simulink model "deltino"  (R2021b)
settings: Solver=VariableStepAuto  StartTime=0.0  StopTime=inf  FixedStep=0.0001  RelTol=1e-3
values from neighbouring files (symbols this model uses):
  alpha1 = 0    [compute_deltino_dyn_parallel.m]
  alpha2 = 2/3*pi    (= 2.09439510239)    [compute_deltino_dyn_parallel.m]
  alpha3 = 4/3*pi    (= 4.18879020479)    [compute_deltino_dyn_parallel.m]
  H = 0.05    [main.m]
  J_T = [J_1', J_2', J_3', J_4']    [main.m]
  K_d = 10    [main.m]
  K_el = 10000    [main.m]
  K_i = 1    [main.m]
  K_p = 200    [main.m]
  K_v = 10    [main.m]
  mu = 0.8    [main.m]
  ni_0 = zeros(18,1)    [main.m]
  offset1 = [l1/2; l2/2; -h/2]    [compute_deltino_dyn_parallel.m]    (also in main.m = [+l1/2; +l2/2; -h/2])
  offset2 = [l1/2; -l2/2; -h/2]    [compute_deltino_dyn_parallel.m]    (also in main.m = [+l1/2; -l2/2; -h/2])
  offset3 = [-l1/2; -l2/2; -h/2]    [compute_deltino_dyn_parallel.m]    (also in main.m)
  offset4 = [-l1/2; l2/2; -h/2]    [compute_deltino_dyn_parallel.m]    (also in main.m = [-l1/2; +l2/2; -h/2])
  p_leg1_0 = forward_kin(theta_leg1_0)    [main.m]
  p_leg2_0 = forward_kin(theta_leg2_0)    [main.m]
  p_leg3_0 = forward_kin(theta_leg3_0)    [main.m]
  p_leg4_0 = forward_kin(theta_leg4_0)    [main.m]
  points_ccw = [+0.1,  0.00 ... (first row only)    [main.m]
  points_cw = [-0.1,  0.00 ... (first row only)    [main.m]
  q_0 = [base_0; ypr_0; theta_leg1_0; ee_leg1_0; theta_leg2_0; ee_leg2_0;        theta_leg3_0; ee_leg3_0; theta_leg4_0; ee_leg4_0;]    [main.m]
  ratio = 2    [main.m]
  steps = 4+2*ratio    (= 8)    [main.m]
  theta_leg1_0 = [pi/6; pi/6; pi/6]    [main.m]
  theta_leg2_0 = [pi/6; pi/6; pi/6]    [main.m]
  theta_leg3_0 = [pi/6; pi/6; pi/6]    [main.m]
  theta_leg4_0 = [pi/6; pi/6; pi/6]    [main.m]
  ts = T/steps    (= 0.1875)    [main.m]
  ts2 = 3*ts    (= 0.5625)    [main.m]
  vel = 0.2    [main.m]
undefined symbols (not defined in the file or in its folder): l1, l_A, l_B, R, radius0, radius1, radius2, theta, WPs
libraries: simulink x14, dspsigops x12
(part 7 of 10)

== matlab function deltino/DELTINO DYNAMICS /compute_C ==
  data: q input; C output; q_dot input
function C = C(q, q_dot)
%#codegen

%    This function was generated by the Symbolic Math Toolbox version 9.0.
%    03-May-2022 19:50:17
phi = q(4); zeta = q(5); psi = q(6);
th11 = q(7); th12 = q(8); th13 = q(9);
th21 = q(13); th22 = q(14); th23 = q(15);
th31 = q(19); th32 = q(20); th33 = q(21);
th41 = q(25); th42 = q(26); th43 = q(27);

bx_dot = q_dot(1); by_dot = q_dot(2); bz_dot = q_dot(3);
phi_dot = q_dot(4); zeta_dot = q_dot(5); psi_dot = q(6);
th11_dot = q_dot(7); th12_dot = q_dot(8); th13_dot = q_dot(9);
th21_dot = q_dot(13); th22_dot = q_dot(14); th23_dot = q_dot(15);
th31_dot = q_dot(19); th32_dot = q_dot(20); th33_dot = q_dot(21);
th41_dot = q_dot(25); th42_dot = q_dot(26); th43_dot = q_dot(27);

t2 = cos(phi);
t3 = cos(psi);
t4 = cos(th11);
t5 = cos(th12);
t6 = cos(th13);
t7 = cos(th21);
t8 = cos(th22);
t9 = cos(th23);
t10 = cos(th31);
t11 = cos(th32);
t12 = cos(th33);
t13 = cos(th41);
t14 = cos(th42);
t15 = cos(th43);
t16 = cos(zeta);
t17 = sin(phi);
t18 = sin(psi);
t19 = sin(th11);
t20 = sin(th12);
t21 = sin(th13);
t22 = sin(th21);
t23 = sin(th22);
t24 = sin(th23);
t25 = sin(th31);
t26 = sin(th32);
t27 = sin(th33);
t28 = sin(th41);
t29 = sin(th42);
t30 = sin(th43);
t31 = sin(zeta);
t32 = psi.*2.0;
t33 = th11.*2.0;
t34 = th12.*2.0;
t35 = th13.*2.0;
t36 = th21.*2.0;
t37 = th22.*2.0;
t38 = th23.*2.0;
t39 = th31.*2.0;
t40 = th32.*2.0;
t41 = th33.*2.0;
t42 = th41.*2.0;
t43 = th42.*2.0;
t44 = th43.*2.0;
t45 = zeta.*2.0;
t92 = sqrt(3.0);
t46 = cos(t32);
t47 = t3.^2;
t48 = cos(t33);
t49 = cos(t34);
t50 = cos(t35);
t51 = cos(t36);
t52 = cos(t37);
t53 = cos(t38);
t54 = cos(t39);
t55 = cos(t40);
t56 = cos(t41);
t57 = cos(t42);
t58 = cos(t43);
t59 = cos(t44);
t60 = t4.^2;
t61 = t5.^2;
t62 = t6.^2;
t63 = t7.^2;
t64 = t8.^2;
t65 = t9.^2;
t66 = t10.^2;
t67 = t11.^2;
t68 = t12.^2;
t69 = t13.^2;
t70 = t14.^2;
t71 = t15.^2;
t72 = cos(t45);
t73 = t16.^2;
t74 = sin(t32);
t75 = sin(t33);
t76 = sin(t34);
t77 = sin(t35);
t78 = sin(t36);
t79 = sin(t37);
t80 = sin(t38);
t81 = sin(t39);
t82 = sin(t40);
t83 = sin(t41);
t84 = sin(t42);
t85 = sin(t43);
t86 = sin(t44);
t87 = sin(t45);
t88 = t2.*t3;
t89 = t2.*t18;
t90 = t3.*t17;
t91 = t17.*t18;
t93 = t19.*t31.*3.0;
t94 = t22.*t31.*3.0;
t95 = t25.*t31.*3.0;
t96 = t28.*t31.*3.0;
t97 = t31./2.0;
t102 = (t2.*t16)./2.0;
t104 = (t16.*t17)./2.0;
t106 = t3.*t4.*t16.*3.0;
t107 = t3.*t7.*t16.*3.0;
t108 = t3.*t10.*t16.*3.0;
t109 = t3.*t13.*t16.*3.0;
t112 = phi_dot.*t4.*(3.0./5.0e+2);
t113 = phi_dot.*t5.*(3.0./5.0e+2);
t114 = phi_dot.*t6.*(3.0./5.0e+2);
t115 = phi_dot.*t7.*(3.0./5.0e+2);
t116 = phi_dot.*t8.*(3.0./5.0e+2);
t117 = phi_dot.*t9.*(3.0./5.0e+2);
t118 = phi_dot.*t10.*(3.0./5.0e+2);
t119 = phi_dot.*t11.*(3.0./5.0e+2);
t120 = phi_dot.*t12.*(3.0./5.0e+2);
t121 = phi_dot.*t13.*(3.0./5.0e+2);
t122 = phi_dot.*t14.*(3.0./5.0e+2);
t123 = phi_dot.*t15.*(3.0./5.0e+2);
t124 = psi_dot.*t4.*(3.0./5.0e+2);
t125 = psi_dot.*t5.*(3.0./5.0e+2);
t126 = psi_dot.*t6.*(3.0./5.0e+2);
t127 = psi_dot.*t7.*(3.0./5.0e+2);
t128 = psi_dot.*t8.*(3.0./5.0e+2);
t129 = psi_dot.*t9.*(3.0./5.0e+2);
t130 = psi_dot.*t10.*(3.0./5.0e+2);
t131 = psi_dot.*t11.*(3.0./5.0e+2);
t132 = psi_dot.*t12.*(3.0./5.0e+2);
t133 = psi_dot.*t13.*(3.0./5.0e+2);
t134 = psi_dot.*t14.*(3.0./5.0e+2);
t135 = psi_dot.*t15.*(3.0./5.0e+2);
t136 = psi_dot.*t18.*(2.0./3.75e+2);
t137 = psi_dot.*t18.*(4.0./3.75e+2);
t138 = t18.*th11_dot.*(2.0./3.75e+2);
t139 = (t18.*th12_dot)./3.75e+2;
t140 = (t18.*th13_dot)./3.75e+2;
t141 = t18.*th21_dot.*(2.0./3.75e+2);
t142 = (t18.*th22_dot)./3.75e+2;
t143 = (t18.*th23_dot)./3.75e+2;
t144 = t18.*th31_dot.*(2.0./3.75e+2);
t145 = (t18.*th32_dot)./3.75e+2;
t146 = (t18.*th33_dot)./3.75e+2;
t147 = t18.*th41_dot.*(2.0./3.75e+2);
t148 = (t18.*th42_dot)./3.75e+2;
t149 = (t18.*th43_dot)./3.75e+2;
t150 = t18.*zeta_dot.*(2.0./3.75e+2);
t151 = t19.*zeta_dot.*(3.0./1.0e+2);
t152 = t22.*zeta_dot.*(3.0./1.0e+2);
t153 = t25.*zeta_dot.*(3.0./2.5e+2);
t154 = t28.*zeta_dot.*(3.0./2.5e+2);
t161 = t20.*zeta_dot.*1.5e-3;
t162 = t21.*zeta_dot.*1.5e-3;
t163 = t23.*zeta_dot.*1.5e-3;
t164 = t24.*zeta_dot.*1.5e-3;
t185 = phi_dot.*t3.*t16.*(2.0./3.75e+2);
t186 = psi_dot.*t3.*t16.*(2.0./3.75e+2);
t187 = psi_dot.*t3.*t16.*(4.0./3.75e+2);
t189 = phi_dot.*t16.*t19.*(3.0./5.0e+2);
t191 = phi_dot.*t16.*t20.*(3.0./5.0e+2);
t193 = phi_dot.*t16.*t21.*(3.0./5.0e+2);
t195 = phi_dot.*t16.*t22.*(3.0./5.0e+2);
t197 = phi_dot.*t16.*t23.*(3.0./5.0e+2);
t199 = phi_dot.*t16.*t24.*(3.0./5.0e+2);
t201 = phi_dot.*t16.*t25.*(3.0./5.0e+2);
t203 = phi_dot.*t16.*t26.*(3.0./5.0e+2);
t205 = phi_dot.*t16.*t27.*(3.0./5.0e+2);
t207 = phi_dot.*t16.*t28.*(3.0./5.0e+2);
t209 = phi_dot.*t16.*t29.*(3.0./5.0e+2);
t211 = phi_dot.*t16.*t30.*(3.0./5.0e+2);
t213 = psi_dot.*t16.*t19.*(3.0./5.0e+2);
t215 = psi_dot.*t16.*t20.*(3.0./5.0e+2);
t217 = psi_dot.*t16.*t21.*(3.0./5.0e+2);
t219 = psi_dot.*t16.*t22.*(3.0./5.0e+2);
t221 = psi_dot.*t16.*t23.*(3.0./5.0e+2);
t223 = psi_dot.*t16.*t24.*(3.0./5.0e+2);
t225 = psi_dot.*t16.*t25.*(3.0./5.0e+2);
t227 = psi_dot.*t16.*t26.*(3.0./5.0e+2);
t229 = psi_dot.*t16.*t27.*(3.0./5.0e+2);
t231 = psi_dot.*t16.*t28.*(3.0./5.0e+2);
t233 = psi_dot.*t16.*t29.*(3.0./5.0e+2);
t235 = psi_dot.*t16.*t30.*(3.0./5.0e+2);
t236 = t4.*t31.*th11_dot.*(3.0./5.0e+2);
t237 = t5.*t31.*th12_dot.*(3.0./5.0e+2);
t238 = t6.*t31.*th13_dot.*(3.0./5.0e+2);
t239 = t7.*t31.*th21_dot.*(3.0./5.0e+2);
t240 = t8.*t31.*th22_dot.*(3.0./5.0e+2);
t241 = t9.*t31.*th23_dot.*(3.0./5.0e+2);
t242 = t10.*t31.*th31_dot.*(3.0./5.0e+2);
t243 = t11.*t31.*th32_dot.*(3.0./5.0e+2);
t244 = t12.*t31.*th33_dot.*(3.0./5.0e+2);
t245 = t13.*t31.*th41_dot.*(3.0./5.0e+2);
t246 = t14.*t31.*th42_dot.*(3.0./5.0e+2);
t247 = t15.*t31.*th43_dot.*(3.0./5.0e+2);
t248 = t18.*t19.*zeta_dot.*(3.0./5.0e+2);
t249 = t18.*t22.*zeta_dot.*(3.0./5.0e+2);
t250 = t18.*t25.*zeta_dot.*(3.0./5.0e+2);
t251 = t18.*t28.*zeta_dot.*(3.0./5.0e+2);
t265 = t18.*t31.*zeta_dot.*(4.0./3.75e+2);
t266 = phi_dot.*t20.*6.75e-3;
t267 = phi_dot.*t21.*6.75e-3;
t268 = phi_dot.*t23.*6.75e-3;
t269 = phi_dot.*t24.*6.75e-3;
t270 = phi_dot.*t26.*6.75e-3;
t271 = phi_dot.*t27.*6.75e-3;
t272 = phi_dot.*t29.*6.75e-3;
t273 = phi_dot.*t30.*6.75e-3;
t274 = psi_dot.*t20.*6.75e-3;
t275 = psi_dot.*t21.*6.75e-3;
t276 = psi_dot.*t23.*6.75e-3;
t277 = psi_dot.*t24.*6.75e-3;
t278 = psi_dot.*t26.*6.75e-3;
t279 = psi_dot.*t27.*6.75e-3;
t280 = psi_dot.*t29.*6.75e-3;
t281 = psi_dot.*t30.*6.75e-3;
t282 = t26.*zeta_dot.*1.95e-2;
t283 = t27.*zeta_dot.*1.95e-2;
t284 = t29.*zeta_dot.*1.95e-2;
t285 = t30.*zeta_dot.*1.95e-2;
t316 = t18.*t20.*zeta_dot.*(3.0./1.0e+3);
t317 = t18.*t21.*zeta_dot.*(3.0./1.0e+3);
t318 = t18.*t23.*zeta_dot.*(3.0./1.0e+3);
t319 = t18.*t24.*zeta_dot.*(3.0./1.0e+3);
t320 = t18.*t26.*zeta_dot.*(3.0./1.0e+3);
t321 = t18.*t27.*zeta_dot.*(3.0./1.0e+3);
t322 = t18.*t29.*zeta_dot.*(3.0./1.0e+3);
t323 = t18.*t30.*zeta_dot.*(3.0./1.0e+3);
t350 = phi_dot.*t3.*t16.*t31.*(4.0./3.75e+2);
t351 = phi_dot.*t3.*t19.*t31.*(3.0./1.0e+2);
t352 = phi_dot.*t4.*t18.*t31.*(3.0./1.0e+2);
t353 = phi_dot.*t3.*t22.*t31.*(3.0./1.0e+2);
t354 = phi_dot.*t7.*t18.*t31.*(3.0./1.0e+2);
t355 = phi_dot.*t3.*t25.*t31.*(3.0./2.5e+2);
t356 = phi_dot.*t10.*t18.*t31.*(3.0./2.5e+2);
t357 = phi_dot.*t3.*t28.*t31.*(3.0./2.5e+2);
t358 = phi_dot.*t13.*t18.*t31.*(3.0./2.5e+2);
t361 = (phi_dot.*t5.*t20.*t31)./3.75e+2;
t362 = (phi_dot.*t6.*t21.*t31)./3.75e+2;
t363 = (phi_dot.*t8.*t23.*t31)./3.75e+2;
t364 = (phi_dot.*t9.*t24.*t31)./3.75e+2;
t365 = (phi_dot.*t11.*t26.*t31)./3.75e+2;
t366 = (phi_dot.*t12.*t27.*t31)./3.75e+2;
t367 = (phi_dot.*t14.*t29.*t31)./3.75e+2;
t368 = (phi_dot.*t15.*t30.*t31)./3.75e+2;
t369 = (psi_dot.*t5.*t20.*t31)./3.75e+2;
t370 = psi_dot.*t4.*t19.*t31.*(4.0./3.75e+2);
t371 = (psi_dot.*t6.*t21.*t31)./3.75e+2;
t372 = (psi_dot.*t8.*t23.*t31)./3.75e+2;
t373 = psi_dot.*t7.*t22.*t31.*(4.0./3.75e+2);
t374 = (psi_dot.*t9.*t24.*t31)./3.75e+2;
t375 = (psi_dot.*t11.*t26.*t31)./3.75e+2;
t376 = psi_dot.*t10.*t25.*t31.*(4.0./3.75e+2);
t377 = (psi_dot.*t12.*t27.*t31)./3.75e+2;
t378 = (psi_dot.*t14.*t29.*t31)./3.75e+2;
t379 = psi_dot.*t13.*t28.*t31.*(4.0./3.75e+2);
t380 = (psi_dot.*t15.*t30.*t31)./3.75e+2;
t381 = (t16.*t18.*t92)./2.0;
t382 = t4.*t19.*t31.*th11_dot.*(4.0./3.75e+2);
t383 = (t5.*t20.*t31.*th12_dot)./3.75e+2;
t384 = (t6.*t21.*t31.*th13_dot)./3.75e+2;
t385 = t7.*t22.*t31.*th21_dot.*(4.0./3.75e+2);
t386 = (t8.*t23.*t31.*th22_dot)./3.75e+2;
t387 = (t9.*t24.*t31.*th23_dot)./3.75e+2;
t388 = t10.*t25.*t31.*th31_dot.*(4.0./3.75e+2);
t389 = (t11.*t26.*t31.*th32_dot)./3.75e+2;
t390 = (t12.*t27.*t31.*th33_dot)./3.75e+2;
t391 = t13.*t28.*t31.*th41_dot.*(4.0./3.75e+2);
t392 = (t14.*t29.*t31.*th42_dot)./3.75e+2;
t393 = (t15.*t30.*t31.*th43_dot)./3.75e+2;
t394 = phi_dot.*t4.*t16.*(2.1e+1./1.0e+3);
t395 = phi_dot.*t5.*t16.*(2.1e+1./1.0e+3);
t396 = phi_dot.*t6.*t16.*(2.1e+1./1.0e+3);
t397 = phi_dot.*t7.*t16.*(2.1e+1./1.0e+3);
t398 = phi_dot.*t8.*t16.*(2.1e+1./1.0e+3);
t399 = phi_dot.*t9.*t16.*(2.1e+1./1.0e+3);
t400 = phi_dot.*t10.*t16.*(2.1e+1./1.0e+3);
t401 = phi_dot.*t11.*t16.*(2.1e+1./1.0e+3);
t402 = phi_dot.*t12.*t16.*(2.1e+1./1.0e+3);
t403 = phi_dot.*t13.*t16.*(2.1e+1./1.0e+3);
t404 = phi_dot.*t14.*t16.*(2.1e+1./1.0e+3);
t405 = phi_dot.*t15.*t16.*(2.1e+1./1.0e+3);
t406 = phi_dot.*t5.*t16.*6.75e-3;
t407 = phi_dot.*t6.*t16.*6.75e-3;
t408 = phi_dot.*t8.*t16.*6.75e-3;
t409 = phi_dot.*t9.*t16.*6.75e-3;
t410 = phi_dot.*t11.*t16.*6.75e-3;
t411 = phi_dot.*t12.*t16.*6.75e-3;
t412 = phi_dot.*t14.*t16.*6.75e-3;
t413 = phi_dot.*t15.*t16.*6.75e-3;
t414 = psi_dot.*t5.*t16.*6.75e-3;
t415 = psi_dot.*t6.*t16.*6.75e-3;
t416 = psi_dot.*t8.*t16.*6.75e-3;
t417 = psi_dot.*t9.*t16.*6.75e-3;
t418 = psi_dot.*t11.*t16.*6.75e-3;
t419 = psi_dot.*t12.*t16.*6.75e-3;
t420 = psi_dot.*t14.*t16.*6.75e-3;
t421 = psi_dot.*t15.*t16.*6.75e-3;
t422 = t4.*t16.*th11_dot.*1.05e-2;
t423 = t5.*t16.*th12_dot.*1.05e-2;
t424 = t6.*t16.*th13_dot.*1.05e-2;
t425 = t7.*t16.*th21_dot.*1.05e-2;
t426 = t8.*t16.*th22_dot.*1.05e-2;
t427 = t9.*t16.*th23_dot.*1.05e-2;
t428 = t10.*t16.*th31_dot.*1.05e-2;
t429 = t11.*t16.*th32_dot.*1.05e-2;
t430 = t12.*t16.*th33_dot.*1.05e-2;
t431 = t13.*t16.*th41_dot.*1.05e-2;
t432 = t14.*t16.*th42_dot.*1.05e-2;
t433 = t15.*t16.*th43_dot.*1.05e-2;
t434 = t3.*t19.*zeta_dot.*(2.1e+1./1.0e+3);
t435 = t3.*t22.*zeta_dot.*(2.1e+1./1.0e+3);
t436 = t3.*t25.*zeta_dot.*(2.1e+1./1.0e+3);
t437 = t3.*t28.*zeta_dot.*(2.1e+1./1.0e+3);
t438 = t3.*t20.*zeta_dot.*1.05e-2;
t439 = t3.*t21.*zeta_dot.*1.05e-2;
t440 = t3.*t23.*zeta_dot.*1.05e-2;
t441 = t3.*t24.*zeta_dot.*1.05e-2;
t442 = t3.*t26.*zeta_dot.*1.05e-2;
t443 = t3.*t27.*zeta_dot.*1.05e-2;
t444 = t3.*t29.*zeta_dot.*1.05e-2;
t445 = t3.*t30.*zeta_dot.*1.05e-2;
t462 = t20.*t31.*th12_dot.*6.75e-3;
t463 = t21.*t31.*th13_dot.*6.75e-3;
t464 = t23.*t31.*th22_dot.*6.75e-3;
t465 = t24.*t31.*th23_dot.*6.75e-3;
t466 = t26.*t31.*th32_dot.*6.75e-3;
t467 = t27.*t31.*th33_dot.*6.75e-3;
t468 = t29.*t31.*th42_dot.*6.75e-3;
t469 = t30.*t31.*th43_dot.*6.75e-3;
t558 = (t16.*t92.*th12_dot)./3.75e+2;
t559 = (t16.*t92.*th13_dot)./3.75e+2;
t560 = (t16.*t92.*th22_dot)./3.75e+2;
t561 = (t16.*t92.*th23_dot)./3.75e+2;
t562 = (t16.*t92.*th32_dot)./3.75e+2;
t563 = (t16.*t92.*th33_dot)./3.75e+2;
t564 = (t16.*t92.*th42_dot)./3.75e+2;
t565 = (t16.*t92.*th43_dot)./3.75e+2;
t566 = t16.*t92.*zeta_dot.*(2.0./3.75e+2);
t567 = phi_dot.*t3.*t5.*t31.*(3.0./1.0e+3);
t568 = phi_dot.*t3.*t16.*t20.*(3.0./1.0e+3);
t569 = phi_dot.*t3.*t6.*t31.*(3.0./1.0e+3);
t570 = phi_dot.*t3.*t16.*t21.*(3.0./1.0e+3);
t571 = phi_dot.*t3.*t8.*t31.*(3.0./1.0e+3);
t572 = phi_dot.*t3.*t16.*t23.*(3.0./1.0e+3);
t573 = phi_dot.*t3.*t9.*t31.*(3.0./1.0e+3);
t574 = phi_dot.*t3.*t16.*t24.*(3.0./1.0e+3);
t575 = phi_dot.*t3.*t11.*t31.*(3.0./1.0e+3);
t576 = phi_dot.*t3.*t16.*t26.*(3.0./1.0e+3);
t577 = phi_dot.*t3.*t12.*t31.*(3.0./1.0e+3);
t578 = phi_dot.*t3.*t16.*t27.*(3.0./1.0e+3);
t579 = phi_dot.*t3.*t14.*t31.*(3.0./1.0e+3);
t580 = phi_dot.*t3.*t16.*t29.*(3.0./1.0e+3);
t581 = phi_dot.*t3.*t15.*t31.*(3.0./1.0e+3);
t582 = phi_dot.*t3.*t16.*t30.*(3.0./1.0e+3);
t583 = phi_dot.*t3.*t16.*t31.*(-2.0./3.75e+2);
t598 = phi_dot.*t16.*3.9545e-1;
t599 = psi_dot.*t16.*3.9545e-1;
t633 = phi_dot.*t3.*t4.*t16.*t31.*(3.0./1.0e+2);
t634 = phi_dot.*t3.*t7.*t16.*t31.*(3.0./1.0e+2);
t635 = phi_dot.*t3.*t10.*t16.*t31.*(3.0./2.5e+2);
t636 = phi_dot.*t3.*t13.*t16.*t31.*(3.0./2.5e+2);
t637 = t3.*t4.*t16.*t18.*zeta_dot.*(3.0./5.0e+2);
t638 = t3.*t5.*t16.*t18.*zeta_dot.*(3.0./5.0e+2);
t639 = t3.*t6.*t16.*t18.*zeta_dot.*(3.0./5.0e+2);
t640 = t3.*t7.*t16.*t18.*zeta_dot.*(3.0./5.0e+2);
t641 = t3.*t8.*t16.*t18.*zeta_dot.*(3.0./5.0e+2);
t642 = t3.*t9.*t16.*t18.*zeta_dot.*(3.0./5.0e+2);
t643 = t3.*t10.*t16.*t18.*zeta_dot.*(3.0./5.0e+2);
t644 = t3.*t11.*t16.*t18.*zeta_dot.*(3.0./5.0e+2);
t645 = t3.*t12.*t16.*t18.*zeta_dot.*(3.0./5.0e+2);
t646 = t3.*t13.*t16.*t18.*zeta_dot.*(3.0./5.0e+2);
t647 = t3.*t14.*t16.*t18.*zeta_dot.*(3.0./5.0e+2);
t648 = t3.*t15.*t16.*t18.*zeta_dot.*(3.0./5.0e+2);
t667 = phi_dot.*t16.*t18.*t19.*t31.*(3.0./1.0e+2);
t668 = phi_dot.*t16.*t18.*t22.*t31.*(3.0./1.0e+2);
t669 = phi_dot.*t16.*t18.*t25.*t31.*(3.0./2.5e+2);
t670 = phi_dot.*t16.*t18.*t28.*t31.*(3.0./2.5e+2);
t671 = t3.*t4.*t18.*zeta_dot.*(2.1e+1./1.0e+3);
t672 = t3.*t5.*t18.*zeta_dot.*(2.1e+1./1.0e+3);
t673 = t3.*t6.*t18.*zeta_dot.*(2.1e+1./1.0e+3);
t674 = t3.*t7.*t18.*zeta_dot.*(2.1e+1./1.0e+3);
t675 = t3.*t8.*t18.*zeta_dot.*(2.1e+1./1.0e+3);
t676 = t3.*t9.*t18.*zeta_dot.*(2.1e+1./1.0e+3);
t677 = t3.*t10.*t18.*zeta_dot.*(2.1e+1./1.0e+3);
t678 = t3.*t11.*t18.*zeta_dot.*(2.1e+1./1.0e+3);
t679 = t3.*t12.*t18.*zeta_dot.*(2.1e+1./1.0e+3);
t680 = t3.*t13.*t18.*zeta_dot.*(2.1e+1./1.0e+3);
t681 = t3.*t14.*t18.*zeta_dot.*(2.1e+1./1.0e+3);
t682 = t3.*t15.*t18.*zeta_dot.*(2.1e+1./1.0e+3);
t683 = phi_dot.*t4.*t18.*t31.*(2.1e+1./1.0e+3);
t684 = phi_dot.*t16.*t18.*t19.*(2.1e+1./1.0e+3);
t685 = phi_dot.*t7.*t18.*t31.*(2.1e+1./1.0e+3);
t686 = phi_dot.*t16.*t18.*t22.*(2.1e+1./1.0e+3);
t687 = phi_dot.*t10.*t18.*t31.*(2.1e+1./1.0e+3);
t688 = phi_dot.*t16.*t18.*t25.*(2.1e+1./1.0e+3);
t689 = phi_dot.*t13.*t18.*t31.*(2.1e+1./1.0e+3);
t690 = phi_dot.*t16.*t18.*t28.*(2.1e+1./1.0e+3);
t691 = phi_dot.*t5.*t18.*t31.*1.05e-2;
t692 = phi_dot.*t16.*t18.*t20.*1.05e-2;
t693 = phi_dot.*t6.*t18.*t31.*1.05e-2;
t694 = phi_dot.*t16.*t18.*t21.*1.05e-2;
t695 = phi_dot.*t8.*t18.*t31.*1.05e-2;
t696 = phi_dot.*t16.*t18.*t23.*1.05e-2;
t697 = phi_dot.*t9.*t18.*t31.*1.05e-2;
t698 = phi_dot.*t16.*t18.*t24.*1.05e-2;
t699 = phi_dot.*t3.*t20.*t31.*1.65e-2;
t700 = phi_dot.*t5.*t18.*t31.*1.65e-2;
t701 = phi_dot.*t3.*t21.*t31.*1.65e-2;
t702 = phi_dot.*t6.*t18.*t31.*1.65e-2;
t703 = phi_dot.*t11.*t18.*t31.*1.05e-2;
t704 = phi_dot.*t16.*t18.*t26.*1.05e-2;
t705 = phi_dot.*t12.*t18.*t31.*1.05e-2;
t706 = phi_dot.*t16.*t18.*t27.*1.05e-2;
t707 = phi_dot.*t3.*t23.*t31.*1.65e-2;
t708 = phi_dot.*t8.*t18.*t31.*1.65e-2;
t709 = phi_dot.*t3.*t24.*t31.*1.65e-2;
t710 = phi_dot.*t9.*t18.*t31.*1.65e-2;
t711 = phi_dot.*t14.*t18.*t31.*1.05e-2;
t712 = phi_dot.*t16.*t18.*t29.*1.05e-2;
t713 = phi_dot.*t15.*t18.*t31.*1.05e-2;
t714 = phi_dot.*t16.*t18.*t30.*1.05e-2;
t715 = phi_dot.*t3.*t26.*t31.*2.55e-2;
t716 = phi_dot.*t11.*t18.*t31.*2.55e-2;
t717 = phi_dot.*t3.*t27.*t31.*2.55e-2;
t718 = phi_dot.*t12.*t18.*t31.*2.55e-2;
t719 = phi_dot.*t3.*t29.*t31.*2.55e-2;
t720 = phi_dot.*t14.*t18.*t31.*2.55e-2;
t721 = phi_dot.*t3.*t30.*t31.*2.55e-2;
t722 = phi_dot.*t15.*t18.*t31.*2.55e-2;
t917 = phi_dot.*t20.*t92.*1.05e-2;
t918 = phi_dot.*t21.*t92.*1.05e-2;
t919 = phi_dot.*t23.*t92.*1.05e-2;
t920 = phi_dot.*t24.*t92.*1.05e-2;
t921 = phi_dot.*t26.*t92.*1.05e-2;
t922 = phi_dot.*t27.*t92.*1.05e-2;
t923 = phi_dot.*t29.*t92.*1.05e-2;
t924 = phi_dot.*t30.*t92.*1.05e-2;
t925 = psi_dot.*t20.*t92.*1.05e-2;
t926 = psi_dot.*t21.*t92.*1.05e-2;
t927 = psi_dot.*t23.*t92.*1.05e-2;
t928 = psi_dot.*t24.*t92.*1.05e-2;
t929 = psi_dot.*t26.*t92.*1.05e-2;
t930 = psi_dot.*t27.*t92.*1.05e-2;
t931 = psi_dot.*t29.*t92.*1.05e-2;
t932 = psi_dot.*t30.*t92.*1.05e-2;
t935 = t20.*t92.*zeta_dot.*1.05e-2;
t936 = t21.*t92.*zeta_dot.*1.05e-2;
t937 = t23.*t92.*zeta_dot.*1.05e-2;
t938 = t24.*t92.*zeta_dot.*1.05e-2;
t939 = t26.*t92.*zeta_dot.*1.05e-2;
t940 = t27.*t92.*zeta_dot.*1.05e-2;
t941 = t29.*t92.*zeta_dot.*1.05e-2;
t942 = t30.*t92.*zeta_dot.*1.05e-2;
t961 = phi_dot.*t5.*t16.*t18.*t31.*(3.0./1.0e+3);
t963 = phi_dot.*t6.*t16.*t18.*t31.*(3.0./1.0e+3);
t965 = phi_dot.*t8.*t16.*t18.*t31.*(3.0./1.0e+3);
t967 = phi_dot.*t9.*t16.*t18.*t31.*(3.0./1.0e+3);
t969 = phi_dot.*t11.*t16.*t18.*t31.*(3.0./1.0e+3);
t971 = phi_dot.*t12.*t16.*t18.*t31.*(3.0./1.0e+3);
t973 = phi_dot.*t14.*t16.*t18.*t31.*(3.0./1.0e+3);
t975 = phi_dot.*t15.*t16.*t18.*t31.*(3.0./1.0e+3);
t976 = t3.*t16.*t18.*t19.*zeta_dot.*(2.1e+1./5.0e+2);
t977 = t3.*t16.*t18.*t20.*zeta_dot.*(2.1e+1./5.0e+2);
t978 = t3.*t16.*t18.*t21.*zeta_dot.*(2.1e+1./5.0e+2);
t979 = t3.*t16.*t18.*t22.*zeta_dot.*(2.1e+1./5.0e+2);
t980 = t3.*t16.*t18.*t23.*zeta_dot.*(2.1e+1./5.0e+2);
t981 = t3.*t16.*t18.*t24.*zeta_dot.*(2.1e+1./5.0e+2);
t982 = t3.*t16.*t18.*t25.*zeta_dot.*(2.1e+1./5.0e+2);
t983 = t3.*t16.*t18.*t26.*zeta_dot.*(2.1e+1./5.0e+2);
t984 = t3.*t16.*t18.*t27.*zeta_dot.*(2.1e+1./5.0e+2);
t985 = t3.*t16.*t18.*t28.*zeta_dot.*(2.1e+1./5.0e+2);
t986 = t3.*t16.*t18.*t29.*zeta_dot.*(2.1e+1./5.0e+2);
t987 = t3.*t16.*t18.*t30.*zeta_dot.*(2.1e+1./5.0e+2);
t1066 = phi_dot.*t3.*t4.*t16.*t18.*t19.*(4.0./3.75e+2);
t1067 = phi_dot.*t3.*t5.*t16.*t18.*t20.*(7.0./3.75e+2);
t1068 = phi_dot.*t3.*t6.*t16.*t18.*t21.*(7.0./3.75e+2);
t1069 = phi_dot.*t3.*t7.*t16.*t18.*t22.*(4.0./3.75e+2);
t1070 = phi_dot.*t3.*t8.*t16.*t18.*t23.*(7.0./3.75e+2);
t1071 = phi_dot.*t3.*t9.*t16.*t18.*t24.*(7.0./3.75e+2);
t1072 = phi_dot.*t3.*t10.*t16.*t18.*t25.*(4.0./3.75e+2);
t1073 = phi_dot.*t3.*t11.*t16.*t18.*t26.*(7.0./3.75e+2);
t1074 = phi_dot.*t3.*t12.*t16.*t18.*t27.*(7.0./3.75e+2);
t1075 = phi_dot.*t3.*t13.*t16.*t18.*t28.*(4.0./3.75e+2);
t1076 = phi_dot.*t3.*t14.*t16.*t18.*t29.*(7.0./3.75e+2);
t1077 = phi_dot.*t3.*t15.*t16.*t18.*t30.*(7.0./3.75e+2);
t1090 = t3.*t4.*t16.*t18.*t19.*zeta_dot.*(4.0./3.75e+2);
t1091 = t3.*t5.*t16.*t18.*t20.*zeta_dot.*(7.0./3.75e+2);
t1092 = t3.*t6.*t16.*t18.*t21.*zeta_dot.*(7.0./3.75e+2);
t1093 = t3.*t7.*t16.*t18.*t22.*zeta_dot.*(4.0./3.75e+2);
t1094 = t3.*t8.*t16.*t18.*t23.*zeta_dot.*(7.0./3.75e+2);
t1095 = t3.*t9.*t16.*t18.*t24.*zeta_dot.*(7.0./3.75e+2);
t1096 = t3.*t10.*t16.*t18.*t25.*zeta_dot.*(4.0./3.75e+2);
t1097 = t3.*t11.*t16.*t18.*t26.*zeta_dot.*(7.0./3.75e+2);
t1098 = t3.*t12.*t16.*t18.*t27.*zeta_dot.*(7.0./3.75e+2);
t1099 = t3.*t13.*t16.*t18.*t28.*zeta_dot.*(4.0./3.75e+2);
t1100 = t3.*t14.*t16.*t18.*t29.*zeta_dot.*(7.0./3.75e+2);
t1101 = t3.*t15.*t16.*t18.*t30.*zeta_dot.*(7.0./3.75e+2);
t1106 = phi_dot.*t4.*t16.*t18.*t19.*t31.*(4.0./3.75e+2);
t1107 = phi_dot.*t5.*t16.*t18.*t20.*t31.*(2.0./3.75e+2);
t1108 = phi_dot.*t6.*t16.*t18.*t21.*t31.*(2.0./3.75e+2);
t1109 = phi_dot.*t7.*t16.*t18.*t22.*t31.*(4.0./3.75e+2);
t1110 = phi_dot.*t8.*t16.*t18.*t23.*t31.*(2.0./3.75e+2);
t1111 = phi_dot.*t9.*t16.*t18.*t24.*t31.*(2.0./3.75e+2);
t1112 = phi_dot.*t10.*t16.*t18.*t25.*t31.*(4.0./3.75e+2);
t1113 = phi_dot.*t11.*t16.*t18.*t26.*t31.*(2.0./3.75e+2);
t1114 = phi_dot.*t12.*t16.*t18.*t27.*t31.*(2.0./3.75e+2);
C = ft_1({phi_dot,psi_dot,t10,t102,t104,t106,t1066,t1067,t1068,t1069,t107,t1070,t1071,t1072,t1073,t1074,t1075,t1076,t1077,t108,t109,t1090,t1091,t1092,t1093,t1094,t1095,t1096,t1097,t1098,t1099,t11,t1100,t1101,t1106,t1107,t1108,t1109,t1110,t1111,t1112,t1113,t1114,t112,t113,t114,t115,t116,t117,t118,t119,t12,t120,t121,t122,t123,t124,t125,t126,t127,t128,t129,t13,t130,t131,t132,t133,t134,t135,t136,t137,t138,t139,t14,t140,t141,t142,t143,t144,t145,t146,t147,t148,t149,t15,t150,t151,t152,t153,t154,t16,t161,t162,t163,t164,t17,t18,t185,t186,t187,t189,t19,t191,t193,t195,t197,t199,t2,t20,t201,t203,t205,t207,t209,t21,t211,t213,t215,t217,t219,t22,t221,t223,t225,t227,t229,t23,t231,t233,t235,t236,t237,t238,t239,t24,t240,t241,t242,t243,t244,t245,t246,t247,t248,t249,t25,t250,t251,t26,t265,t266,t267,t268,t269,t27,t270,t271,t272,t273,t274,t275,t276,t277,t278,t279,t28,t280,t281,t282,t283,t284,t285,t29,t3,t30,t31,t316,t317,t318,t319,t320,t321,t322,t323,t350,t351,t352,t353,t354,t355,t356,t357,t358,t361,t362,t363,t364,t365,t366,t367,t368,t369,t370,t371,t372,t373,t374,t375,t376,t377,t378,t379,t380,t381,t382,t383,t384,t385,t386,t387,t388,t389,t390,t391,t392,t393,t394,t395,t396,t397,t398,t399,t4,t400,t401,t402,t403,t404,t405,t406,t407,t408,t409,t410,t411,t412,t413,t414,t415,t416,t417,t418,t419,t420,t421,t422,t423,t424,t425,t426,t427,t428,t429,t430,t431,t432,t433,t434,t435,t436,t437,t438,t439,t440,t441,t442,t443,t444,t445,t46,t462,t463,t464,t465,t466,t467,t468,t469,t47,t48,t49,t5,t50,t51,t52,t53,t54,t55,t558,t559,t56,t560,t561,t562,t563,t564,t565,t566,t567,t568,t569,t57,t570,t571,t572,t573,t574,t575,t576,t577,t578,t579,t58,t580,t581,t582,t583,t59,t598,t599,t6,t60,t61,t62,t63,t633,t634,t635,t636,t637,t638,t639,t64,t640,t641,t642,t643,t644,t645,t646,t647,t648,t65,t66,t667,t668,t669,t67,t670,t671,t672,t673,t674,t675,t676,t677,t678,t679,t68,t680,t681,t682,t683,t684,t685,t686,t687,t688,t689,t69,t690,t691,t692,t693,t694,t695,t696,t697,t698,t699,t7,t70,t700,t701,t702,t703,t704,t705,t706,t707,t708,t709,t71,t710,t711,t712,t713,t714,t715,t716,t717,t718,t719,t72,t720,t721,t722,t73,t74,t75,t76,t77,t78,t79,t8,t80,t81,t82,t83,t84,t85,t86,t87,t88,t89,t9,t90,t91,t917,t918,t919,t92,t920,t921,t922,t923,t924,t925,t926,t927,t928,t929,t93,t930,t931,t932,t935,t936,t937,t938,t939,t94,t940,t941,t942,t95,t96,t961,t963,t965,t967,t969,t97,t971,t973,t975,t976,t977,t978,t979,t980,t981,t982,t983,t984,t985,t986,t987,th11_dot,th12_dot,th13_dot,th21_dot,th22_dot,th23_dot,th31_dot,th32_dot,th33_dot,th41_dot,th42_dot,th43_dot,zeta_dot});
end
function C = ft_1(ct)
phi_dot = ct{1};
psi_dot = ct{2};
t10 = ct{3};
t102 = ct{4};
t104 = ct{5};
t106 = ct{6};
t1066 = ct{7};
t1067 = ct{8};
t1068 = ct{9};
t1069 = ct{10};
t107 = ct{11};
t1070 = ct{12};
t1071 = ct{13};
t1072 = ct{14};
t1073 = ct{15};
t1074 = ct{16};
t1075 = ct{17};
t1076 = ct{18};
t1077 = ct{19};
t108 = ct{20};
t109 = ct{21};
t1090 = ct{22};
t1091 = ct{23};
t1092 = ct{24};
t1093 = ct{25};
t1094 = ct{26};
t1095 = ct{27};
t1096 = ct{28};
t1097 = ct{29};
t1098 = ct{30};
t1099 = ct{31};
t11 = ct{32};
t1100 = ct{33};
t1101 = ct{34};
t1106 = ct{35};
t1107 = ct{36};
t1108 = ct{37};
t1109 = ct{38};
t1110 = ct{39};
t1111 = ct{40};
t1112 = ct{41};
t1113 = ct{42};
t1114 = ct{43};
t112 = ct{44};
t113 = ct{45};
t114 = ct{46};
t115 = ct{47};
t116 = ct{48};
t117 = ct{49};
t118 = ct{50};
t119 = ct{51};
t12 = ct{52};
t120 = ct{53};
t121 = ct{54};
t122 = ct{55};
t123 = ct{56};
t124 = ct{57};
t125 = ct{58};
t126 = ct{59};
t127 = ct{60};
t128 = ct{61};
t129 = ct{62};
t13 = ct{63};
t130 = ct{64};
t131 = ct{65};
t132 = ct{66};
t133 = ct{67};
t134 = ct{68};
t135 = ct{69};
t136 = ct{70};
t137 = ct{71};
t138 = ct{72};
t139 = ct{73};
t14 = ct{74};
t140 = ct{75};
t141 = ct{76};
t142 = ct{77};
t143 = ct{78};
t144 = ct{79};
t145 = ct{80};
t146 = ct{81};
t147 = ct{82};
t148 = ct{83};
t149 = ct{84};
t15 = ct{85};
t150 = ct{86};
t151 = ct{87};
t152 = ct{88};
t153 = ct{89};
t154 = ct{90};
t16 = ct{91};
t161 = ct{92};
t162 = ct{93};
t163 = ct{94};
t164 = ct{95};
t17 = ct{96};
t18 = ct{97};
t185 = ct{98};
t186 = ct{99};
t187 = ct{100};
t189 = ct{101};
t19 = ct{102};
t191 = ct{103};
t193 = ct{104};
t195 = ct{105};
t197 = ct{106};
t199 = ct{107};
t2 = ct{108};
t20 = ct{109};
t201 = ct{110};
t203 = ct{111};
t205 = ct{112};
t207 = ct{113};
t209 = ct{114};
t21 = ct{115};
t211 = ct{116};
t213 = ct{117};
t215 = ct{118};
t217 = ct{119};
t219 = ct{120};
t22 = ct{121};
t221 = ct{122};
t223 = ct{123};
t225 = ct{124};
t227 = ct{125};
t229 = ct{126};
t23 = ct{127};
t231 = ct{128};
t233 = ct{129};
t235 = ct{130};
t236 = ct{131};
t237 = ct{132};
t238 = ct{133};
t239 = ct{134};
t24 = ct{135};
t240 = ct{136};
t241 = ct{137};
t242 = ct{138};
t243 = ct{139};
t244 = ct{140};
t245 = ct{141};
t246 = ct{142};
t247 = ct{143};
t248 = ct{144};
t249 = ct{145};
t25 = ct{146};
t250 = ct{147};
t251 = ct{148};
t26 = ct{149};
t265 = ct{150};
t266 = ct{151};
t267 = ct{152};
t268 = ct{153};
t269 = ct{154};
t27 = ct{155};
t270 = ct{156};
t271 = ct{157};
t272 = ct{158};
t273 = ct{159};
t274 = ct{160};
t275 = ct{161};
t276 = ct{162};
t277 = ct{163};
t278 = ct{164};
t279 = ct{165};
t28 = ct{166};
t280 = ct{167};
t281 = ct{168};
t282 = ct{169};
t283 = ct{170};
t284 = ct{171};
t285 = ct{172};
t29 = ct{173};
t3 = ct{174};
t30 = ct{175};
t31 = ct{176};
t316 = ct{177};
t317 = ct{178};
t318 = ct{179};
t319 = ct{180};
t320 = ct{181};
t321 = ct{182};
t322 = ct{183};
t323 = ct{184};
t350 = ct{185};
t351 = ct{186};
t352 = ct{187};
t353 = ct{188};
t354 = ct{189};
t355 = ct{190};
t356 = ct{191};
t357 = ct{192};
t358 = ct{193};
t361 = ct{194};
t362 = ct{195};
t363 = ct{196};
t364 = ct{197};
t365 = ct{198};
t366 = ct{199};
t367 = ct{200};
t368 = ct{201};
t369 = ct{202};
t370 = ct{203};
t371 = ct{204};
t372 = ct{205};
t373 = ct{206};
t374 = ct{207};
t375 = ct{208};
t376 = ct{209};
t377 = ct{210};
t378 = ct{211};
t379 = ct{212};
t380 = ct{213};
t381 = ct{214};
t382 = ct{215};
t383 = ct{216};
t384 = ct{217};
t385 = ct{218};
t386 = ct{219};
t387 = ct{220};
t388 = ct{221};
t389 = ct{222};
t390 = ct{223};
t391 = ct{224};
t392 = ct{225};
t393 = ct{226};
t394 = ct{227};
t395 = ct{228};
t396 = ct{229};
t397 = ct{230};
t398 = ct{231};
t399 = ct{232};
t4 = ct{233};
t400 = ct{234};
t401 = ct{235};
t402 = ct{236};
t403 = ct{237};
t404 = ct{238};
t405 = ct{239};
t406 = ct{240};
t407 = ct{241};
t408 = ct{242};
t409 = ct{243};
t410 = ct{244};
t411 = ct{245};
t412 = ct{246};
t413 = ct{247};
t414 = ct{248};
t415 = ct{249};
t416 = ct{250};
t417 = ct{251};
t418 = ct{252};
t419 = ct{253};
t420 = ct{254};
t421 = ct{255};
t422 = ct{256};
t423 = ct{257};
t424 = ct{258};
t425 = ct{259};
t426 = ct{260};
t427 = ct{261};
t428 = ct{262};
t429 = ct{263};
t430 = ct{264};
t431 = ct{265};
t432 = ct{266};
t433 = ct{267};
t434 = ct{268};
t435 = ct{269};
t436 = ct{270};
t437 = ct{271};
t438 = ct{272};
t439 = ct{273};
t440 = ct{274};
t441 = ct{275};
t442 = ct{276};
t443 = ct{277};
t444 = ct{278};
t445 = ct{279};
t46 = ct{280};
t462 = ct{281};
t463 = ct{282};
t464 = ct{283};
t465 = ct{284};
t466 = ct{285};
t467 = ct{286};
t468 = ct{287};
t469 = ct{288};
t47 = ct{289};
t48 = ct{290};
t49 = ct{291};
t5 = ct{292};
t50 = ct{293};
t51 = ct{294};
t52 = ct{295};
t53 = ct{296};
t54 = ct{297};
t55 = ct{298};
t558 = ct{299};
t559 = ct{300};
t56 = ct{301};
t560 = ct{302};
t561 = ct{303};
t562 = ct{304};
t563 = ct{305};
t564 = ct{306};
t565 = ct{307};
t566 = ct{308};
t567 = ct{309};
t568 = ct{310};
t569 = ct{311};
t57 = ct{312};
t570 = ct{313};
t571 = ct{314};
t572 = ct{315};
t573 = ct{316};
t574 = ct{317};
t575 = ct{318};
t576 = ct{319};
t577 = ct{320};
t578 = ct{321};
t579 = ct{322};
t58 = ct{323};
t580 = ct{324};
t581 = ct{325};
t582 = ct{326};
t583 = ct{327};
t59 = ct{328};
t598 = ct{329};
t599 = ct{330};
t6 = ct{331};
t60 = ct{332};
t61 = ct{333};
t62 = ct{334};
t63 = ct{335};
t633 = ct{336};
t634 = ct{337};
t635 = ct{338};
t636 = ct{339};
t637 = ct{340};
t638 = ct{341};
t639 = ct{342};
t64 = ct{343};
t640 = ct{344};
t641 = ct{345};
t642 = ct{346};
t643 = ct{347};
t644 = ct{348};
t645 = ct{349};
t646 = ct{350};
t647 = ct{351};
t648 = ct{352};
t65 = ct{353};
t66 = ct{354};
t667 = ct{355};
t668 = ct{356};
t669 = ct{357};
t67 = ct{358};
t670 = ct{359};
t671 = ct{360};
t672 = ct{361};
t673 = ct{362};
t674 = ct{363};
t675 = ct{364};
t676 = ct{365};
t677 = ct{366};
t678 = ct{367};
t679 = ct{368};
t68 = ct{369};
t680 = ct{370};
t681 = ct{371};
t682 = ct{372};
t683 = ct{373};
t684 = ct{374};
t685 = ct{375};
t686 = ct{376};
t687 = ct{377};
t688 = ct{378};
t689 = ct{379};
t69 = ct{380};
t690 = ct{381};
t691 = ct{382};
t692 = ct{383};
t693 = ct{384};
t694 = ct{385};
t695 = ct{386};
t696 = ct{387};
t697 = ct{388};
t698 = ct{389};
t699 = ct{390};
t7 = ct{391};
t70 = ct{392};
t700 = ct{393};
t701 = ct{394};
t702 = ct{395};
t703 = ct{396};
t704 = ct{397};
t705 = ct{398};
t706 = ct{399};
t707 = ct{400};
t708 = ct{401};
t709 = ct{402};
t71 = ct{403};
t710 = ct{404};
t711 = ct{405};
t712 = ct{406};
t713 = ct{407};
t714 = ct{408};
t715 = ct{409};
t716 = ct{410};
t717 = ct{411};
t718 = ct{412};
t719 = ct{413};
t72 = ct{414};
t720 = ct{415};
t721 = ct{416};
t722 = ct{417};
t73 = ct{418};
t74 = ct{419};
t75 = ct{420};
t76 = ct{421};
t77 = ct{422};
t78 = ct{423};
t79 = ct{424};
t8 = ct{425};
t80 = ct{426};
t81 = ct{427};
t82 = ct{428};
t83 = ct{429};
t84 = ct{430};
t85 = ct{431};
t86 = ct{432};
t87 = ct{433};
t88 = ct{434};
t89 = ct{435};
t9 = ct{436};
t90 = ct{437};
t91 = ct{438};
t917 = ct{439};
t918 = ct{440};
t919 = ct{441};
t92 = ct{442};
t920 = ct{443};
t921 = ct{444};
t922 = ct{445};
t923 = ct{446};
t924 = ct{447};
t925 = ct{448};
t926 = ct{449};
t927 = ct{450};
t928 = ct{451};
t929 = ct{452};
t93 = ct{453};
t930 = ct{454};
t931 = ct{455};
t932 = ct{456};
t935 = ct{457};
t936 = ct{458};
t937 = ct{459};
t938 = ct{460};
t939 = ct{461};
t94 = ct{462};
t940 = ct{463};
t941 = ct{464};
t942 = ct{465};
t95 = ct{466};
t96 = ct{467};
t961 = ct{468};
t963 = ct{469};
t965 = ct{470};
t967 = ct{471};
t969 = ct{472};
t97 = ct{473};
t971 = ct{474};
t973 = ct{475};
t975 = ct{476};
t976 = ct{477};
t977 = ct{478};
t978 = ct{479};
t979 = ct{480};
t980 = ct{481};
t981 = ct{482};
t982 = ct{483};
t983 = ct{484};
t984 = ct{485};
t985 = ct{486};
t986 = ct{487};
t987 = ct{488};
th11_dot = ct{489};
th12_dot = ct{490};
th13_dot = ct{491};
th21_dot = ct{492};
th22_dot = ct{493};
th23_dot = ct{494};
th31_dot = ct{495};
th32_dot = ct{496};
th33_dot = ct{497};
th41_dot = ct{498};
th42_dot = ct{499};
th43_dot = ct{500};
zeta_dot = ct{501};
t1115 = phi_dot.*t13.*t16.*t18.*t28.*t31.*(4.0./3.75e+2);
t1116 = phi_dot.*t14.*t16.*t18.*t29.*t31.*(2.0./3.75e+2);
t1117 = phi_dot.*t15.*t16.*t18.*t30.*t31.*(2.0./3.75e+2);
t1122 = phi_dot.*t3.*t5.*t16.*t31.*1.05e-2;
t1123 = phi_dot.*t3.*t6.*t16.*t31.*1.05e-2;
t1124 = phi_dot.*t3.*t8.*t16.*t31.*1.05e-2;
t1125 = phi_dot.*t3.*t9.*t16.*t31.*1.05e-2;
t1126 = phi_dot.*t3.*t5.*t16.*t31.*1.65e-2;
t1127 = phi_dot.*t3.*t6.*t16.*t31.*1.65e-2;
t1128 = phi_dot.*t3.*t11.*t16.*t31.*1.05e-2;
t1129 = phi_dot.*t3.*t12.*t16.*t31.*1.05e-2;
t1130 = phi_dot.*t3.*t8.*t16.*t31.*1.65e-2;
t1131 = phi_dot.*t3.*t9.*t16.*t31.*1.65e-2;
t1132 = phi_dot.*t3.*t14.*t16.*t31.*1.05e-2;
t1133 = phi_dot.*t3.*t15.*t16.*t31.*1.05e-2;
t1134 = phi_dot.*t3.*t11.*t16.*t31.*2.55e-2;
t1135 = phi_dot.*t3.*t12.*t16.*t31.*2.55e-2;
t1136 = phi_dot.*t3.*t14.*t16.*t31.*2.55e-2;
t1137 = phi_dot.*t3.*t15.*t16.*t31.*2.55e-2;
t1146 = t3.*t16.*t18.*t20.*zeta_dot.*6.75e-3;
t1147 = t3.*t16.*t18.*t21.*zeta_dot.*6.75e-3;
t1148 = t3.*t16.*t18.*t23.*zeta_dot.*6.75e-3;
t1149 = t3.*t16.*t18.*t24.*zeta_dot.*6.75e-3;
t1150 = t3.*t16.*t18.*t26.*zeta_dot.*6.75e-3;
t1151 = t3.*t16.*t18.*t27.*zeta_dot.*6.75e-3;
t1152 = t3.*t16.*t18.*t29.*zeta_dot.*6.75e-3;
t1153 = t3.*t16.*t18.*t30.*zeta_dot.*6.75e-3;
t1162 = phi_dot.*t16.*t18.*t20.*t31.*1.65e-2;
t1163 = phi_dot.*t16.*t18.*t21.*t31.*1.65e-2;
t1166 = phi_dot.*t16.*t18.*t23.*t31.*1.65e-2;
t1167 = phi_dot.*t16.*t18.*t24.*t31.*1.65e-2;
t1170 = phi_dot.*t16.*t18.*t26.*t31.*2.55e-2;
t1171 = phi_dot.*t16.*t18.*t27.*t31.*2.55e-2;
t1172 = phi_dot.*t16.*t18.*t29.*t31.*2.55e-2;
t1173 = phi_dot.*t16.*t18.*t30.*t31.*2.55e-2;
t1308 = t16.*t20.*t92.*th12_dot.*1.5e-3;
t1309 = t16.*t21.*t92.*th13_dot.*1.5e-3;
t1310 = t16.*t23.*t92.*th22_dot.*1.5e-3;
t1311 = t16.*t24.*t92.*th23_dot.*1.5e-3;
t1312 = t16.*t26.*t92.*th32_dot.*1.5e-3;
t1313 = t16.*t27.*t92.*th33_dot.*1.5e-3;
t1314 = t16.*t29.*t92.*th42_dot.*1.5e-3;
t1315 = t16.*t30.*t92.*th43_dot.*1.5e-3;
t1332 = t20.*t31.*t92.*th12_dot.*1.05e-2;
t1333 = t21.*t31.*t92.*th13_dot.*1.05e-2;
t1334 = t23.*t31.*t92.*th22_dot.*1.05e-2;
t1335 = t24.*t31.*t92.*th23_dot.*1.05e-2;
t1336 = t26.*t31.*t92.*th32_dot.*1.05e-2;
t1337 = t27.*t31.*t92.*th33_dot.*1.05e-2;
t1338 = t29.*t31.*t92.*th42_dot.*1.05e-2;
t1339 = t30.*t31.*t92.*th43_dot.*1.05e-2;
t1428 = (psi_dot.*t3.*t5.*t20.*t92)./3.75e+2;
t1429 = (psi_dot.*t3.*t6.*t21.*t92)./3.75e+2;
t1430 = (psi_dot.*t3.*t8.*t23.*t92)./3.75e+2;
t1431 = (psi_dot.*t3.*t9.*t24.*t92)./3.75e+2;
t1432 = (psi_dot.*t3.*t11.*t26.*t92)./3.75e+2;
t1433 = (psi_dot.*t3.*t12.*t27.*t92)./3.75e+2;
t1434 = (psi_dot.*t3.*t14.*t29.*t92)./3.75e+2;
t1435 = (psi_dot.*t3.*t15.*t30.*t92)./3.75e+2;
t1436 = (t3.*t5.*t20.*t92.*zeta_dot)./3.75e+2;
t1437 = (t3.*t6.*t21.*t92.*zeta_dot)./3.75e+2;
t1438 = (t3.*t8.*t23.*t92.*zeta_dot)./3.75e+2;
t1439 = (t3.*t9.*t24.*t92.*zeta_dot)./3.75e+2;
t1440 = (t3.*t11.*t26.*t92.*zeta_dot)./3.75e+2;
t1441 = (t3.*t12.*t27.*t92.*zeta_dot)./3.75e+2;
t1442 = (t3.*t14.*t29.*t92.*zeta_dot)./3.75e+2;
t1443 = (t3.*t15.*t30.*t92.*zeta_dot)./3.75e+2;
t1444 = phi_dot.*t11.*t18.*t31.*t92.*(3.0./2.0e+2);
t1445 = phi_dot.*t12.*t18.*t31.*t92.*(3.0./2.0e+2);
t1446 = phi_dot.*t14.*t18.*t31.*t92.*(3.0./2.0e+2);
t1447 = phi_dot.*t15.*t18.*t31.*t92.*(3.0./2.0e+2);
t1460 = phi_dot.*t5.*t16.*t92.*4.5e-3;
t1461 = phi_dot.*t6.*t16.*t92.*4.5e-3;
t1462 = phi_dot.*t8.*t16.*t92.*4.5e-3;
t1463 = phi_dot.*t9.*t16.*t92.*4.5e-3;
t1464 = phi_dot.*t5.*t16.*t92.*1.05e-2;
t1465 = phi_dot.*t6.*t16.*t92.*1.05e-2;
t1466 = phi_dot.*t11.*t16.*t92.*4.5e-3;
t1467 = phi_dot.*t12.*t16.*t92.*4.5e-3;
t1468 = phi_dot.*t8.*t16.*t92.*1.05e-2;
t1469 = phi_dot.*t9.*t16.*t92.*1.05e-2;
t1470 = phi_dot.*t14.*t16.*t92.*4.5e-3;
t1471 = phi_dot.*t15.*t16.*t92.*4.5e-3;
t1472 = phi_dot.*t11.*t16.*t92.*1.05e-2;
t1473 = phi_dot.*t12.*t16.*t92.*1.05e-2;
t1474 = phi_dot.*t14.*t16.*t92.*1.05e-2;
t1475 = phi_dot.*t15.*t16.*t92.*1.05e-2;
t1476 = psi_dot.*t5.*t16.*t92.*1.05e-2;
t1477 = psi_dot.*t6.*t16.*t92.*1.05e-2;
t1478 = psi_dot.*t8.*t16.*t92.*1.05e-2;
t1479 = psi_dot.*t9.*t16.*t92.*1.05e-2;
t1480 = psi_dot.*t11.*t16.*t92.*1.05e-2;
t1481 = psi_dot.*t12.*t16.*t92.*1.05e-2;
t1482 = psi_dot.*t14.*t16.*t92.*1.05e-2;
t1483 = psi_dot.*t15.*t16.*t92.*1.05e-2;
t1484 = t5.*t16.*t92.*th12_dot.*2.25e-3;
t1485 = t6.*t16.*t92.*th13_dot.*2.25e-3;
t1486 = t8.*t16.*t92.*th22_dot.*2.25e-3;
t1487 = t9.*t16.*t92.*th23_dot.*2.25e-3;
t1488 = t11.*t16.*t92.*th32_dot.*2.25e-3;
t1489 = t12.*t16.*t92.*th33_dot.*2.25e-3;
t1490 = t14.*t16.*t92.*th42_dot.*2.25e-3;
t1491 = t15.*t16.*t92.*th43_dot.*2.25e-3;
t1492 = t3.*t20.*t92.*zeta_dot.*2.25e-3;
t1493 = t3.*t21.*t92.*zeta_dot.*2.25e-3;
t1494 = t3.*t23.*t92.*zeta_dot.*2.25e-3;
t1495 = t3.*t24.*t92.*zeta_dot.*2.25e-3;
t1496 = t3.*t26.*t92.*zeta_dot.*2.25e-3;
t1497 = t3.*t27.*t92.*zeta_dot.*2.25e-3;
t1498 = t3.*t29.*t92.*zeta_dot.*2.25e-3;
t1499 = t3.*t30.*t92.*zeta_dot.*2.25e-3;
t1711 = phi_dot.*t3.*t11.*t16.*t31.*t92.*(3.0./2.0e+2);
t1712 = phi_dot.*t3.*t12.*t16.*t31.*t92.*(3.0./2.0e+2);
t1713 = phi_dot.*t3.*t14.*t16.*t31.*t92.*(3.0./2.0e+2);
t1714 = phi_dot.*t3.*t15.*t16.*t31.*t92.*(3.0./2.0e+2);
t1728 = (phi_dot.*t5.*t16.*t18.*t20.*t92)./3.75e+2;
t1730 = (phi_dot.*t6.*t16.*t18.*t21.*t92)./3.75e+2;
t1732 = (phi_dot.*t8.*t16.*t18.*t23.*t92)./3.75e+2;
t1734 = (phi_dot.*t9.*t16.*t18.*t24.*t92)./3.75e+2;
t1736 = (phi_dot.*t11.*t16.*t18.*t26.*t92)./3.75e+2;
t1738 = (phi_dot.*t12.*t16.*t18.*t27.*t92)./3.75e+2;
t1740 = (phi_dot.*t14.*t16.*t18.*t29.*t92)./3.75e+2;
t1742 = (phi_dot.*t15.*t16.*t18.*t30.*t92)./3.75e+2;
t1743 = (psi_dot.*t5.*t16.*t18.*t20.*t92)./3.75e+2;
t1744 = (psi_dot.*t6.*t16.*t18.*t21.*t92)./3.75e+2;
t1745 = (psi_dot.*t8.*t16.*t18.*t23.*t92)./3.75e+2;
t1746 = (psi_dot.*t9.*t16.*t18.*t24.*t92)./3.75e+2;
t1747 = (psi_dot.*t11.*t16.*t18.*t26.*t92)./3.75e+2;
t1748 = (psi_dot.*t12.*t16.*t18.*t27.*t92)./3.75e+2;
t1749 = (psi_dot.*t14.*t16.*t18.*t29.*t92)./3.75e+2;
t1750 = (psi_dot.*t15.*t16.*t18.*t30.*t92)./3.75e+2;
t1775 = phi_dot.*t16.*t18.*t26.*t31.*t92.*(3.0./2.0e+2);
t1776 = phi_dot.*t16.*t18.*t27.*t31.*t92.*(3.0./2.0e+2);
t1777 = phi_dot.*t16.*t18.*t29.*t31.*t92.*(3.0./2.0e+2);
t1778 = phi_dot.*t16.*t18.*t30.*t31.*t92.*(3.0./2.0e+2);
t1783 = t3.*t5.*t18.*t92.*zeta_dot.*4.5e-3;
t1784 = t3.*t6.*t18.*t92.*zeta_dot.*4.5e-3;
t1785 = t3.*t8.*t18.*t92.*zeta_dot.*4.5e-3;
t1786 = t3.*t9.*t18.*t92.*zeta_dot.*4.5e-3;
t1787 = t3.*t11.*t18.*t92.*zeta_dot.*4.5e-3;
t1788 = t3.*t12.*t18.*t92.*zeta_dot.*4.5e-3;
t1789 = t3.*t14.*t18.*t92.*zeta_dot.*4.5e-3;
t1790 = t3.*t15.*t18.*t92.*zeta_dot.*4.5e-3;
t1791 = phi_dot.*t16.*t18.*t20.*t92.*2.25e-3;
t1792 = phi_dot.*t16.*t18.*t21.*t92.*2.25e-3;
t1793 = phi_dot.*t16.*t18.*t23.*t92.*2.25e-3;
t1794 = phi_dot.*t16.*t18.*t24.*t92.*2.25e-3;
t1795 = phi_dot.*t16.*t18.*t26.*t92.*2.25e-3;
t1796 = phi_dot.*t16.*t18.*t27.*t92.*2.25e-3;
t1797 = phi_dot.*t3.*t20.*t31.*t92.*8.25e-3;
t1798 = phi_dot.*t3.*t21.*t31.*t92.*8.25e-3;
t1799 = phi_dot.*t16.*t18.*t29.*t92.*2.25e-3;
t1800 = phi_dot.*t16.*t18.*t30.*t92.*2.25e-3;
t1801 = phi_dot.*t3.*t23.*t31.*t92.*8.25e-3;
t1802 = phi_dot.*t3.*t24.*t31.*t92.*8.25e-3;
t1803 = phi_dot.*t3.*t26.*t31.*t92.*1.275e-2;
t1804 = phi_dot.*t3.*t27.*t31.*t92.*1.275e-2;
t1805 = phi_dot.*t3.*t29.*t31.*t92.*1.275e-2;
t1806 = phi_dot.*t3.*t30.*t31.*t92.*1.275e-2;
t1865 = t5.*t16.*t18.*t20.*t92.*th12_dot.*(-1.0./3.75e+2);
t1866 = t8.*t16.*t18.*t23.*t92.*th22_dot.*(-1.0./3.75e+2);
t1867 = t11.*t16.*t18.*t26.*t92.*th32_dot.*(-1.0./3.75e+2);
t1868 = t14.*t16.*t18.*t29.*t92.*th42_dot.*(-1.0./3.75e+2);
t1994 = t3.*t5.*t16.*t18.*t20.*t92.*zeta_dot.*(4.0./3.75e+2);
t1995 = t3.*t6.*t16.*t18.*t21.*t92.*zeta_dot.*(4.0./3.75e+2);
t1996 = t3.*t8.*t16.*t18.*t23.*t92.*zeta_dot.*(4.0./3.75e+2);
t1997 = t3.*t9.*t16.*t18.*t24.*t92.*zeta_dot.*(4.0./3.75e+2);
t1998 = t3.*t11.*t16.*t18.*t26.*t92.*zeta_dot.*(4.0./3.75e+2);
t1999 = t3.*t12.*t16.*t18.*t27.*t92.*zeta_dot.*(4.0./3.75e+2);
t2000 = t3.*t14.*t16.*t18.*t29.*t92.*zeta_dot.*(4.0./3.75e+2);
t2001 = t3.*t15.*t16.*t18.*t30.*t92.*zeta_dot.*(4.0./3.75e+2);
t2034 = t3.*t16.*t18.*t20.*t92.*zeta_dot.*(9.0./1.0e+3);
t2035 = t3.*t16.*t18.*t21.*t92.*zeta_dot.*(9.0./1.0e+3);
t2036 = t3.*t16.*t18.*t23.*t92.*zeta_dot.*(9.0./1.0e+3);
t2037 = t3.*t16.*t18.*t24.*t92.*zeta_dot.*(9.0./1.0e+3);
t2038 = t3.*t16.*t18.*t26.*t92.*zeta_dot.*(9.0./1.0e+3);
t2039 = t3.*t16.*t18.*t27.*t92.*zeta_dot.*(9.0./1.0e+3);
t2040 = t3.*t16.*t18.*t29.*t92.*zeta_dot.*(9.0./1.0e+3);
t2041 = t3.*t16.*t18.*t30.*t92.*zeta_dot.*(9.0./1.0e+3);
t98 = t31.*t89;
t99 = t31.*t90;
t100 = t31.*t91;
t101 = t31.*t88;
t103 = t2.*t97;
t105 = t17.*t97;
t155 = -t106;
t156 = -t107;
t157 = -t108;
t158 = -t109;
t159 = -t137;
t160 = -t150;
t165 = phi_dot.*t75.*(2.0./3.75e+2);
t166 = phi_dot.*t78.*(2.0./3.75e+2);
t167 = phi_dot.*t81.*(2.0./3.75e+2);
t168 = phi_dot.*t84.*(2.0./3.75e+2);
t169 = psi_dot.*t75.*(2.0./3.75e+2);
t170 = psi_dot.*t78.*(2.0./3.75e+2);
t171 = psi_dot.*t81.*(2.0./3.75e+2);
t172 = psi_dot.*t84.*(2.0./3.75e+2);
t173 = t75.*zeta_dot.*(2.0./3.75e+2);
t174 = t76.*zeta_dot.*(2.0./3.75e+2);
t175 = t77.*zeta_dot.*(2.0./3.75e+2);
t176 = t78.*zeta_dot.*(2.0./3.75e+2);
t177 = t79.*zeta_dot.*(2.0./3.75e+2);
t178 = t80.*zeta_dot.*(2.0./3.75e+2);
t179 = t81.*zeta_dot.*(2.0./3.75e+2);
t180 = t82.*zeta_dot.*(2.0./3.75e+2);
t181 = t83.*zeta_dot.*(2.0./3.75e+2);
t182 = t84.*zeta_dot.*(2.0./3.75e+2);
t183 = t85.*zeta_dot.*(2.0./3.75e+2);
t184 = t86.*zeta_dot.*(2.0./3.75e+2);
t188 = t31.*t112;
t190 = t31.*t113;
t192 = t31.*t114;
t194 = t31.*t115;
t196 = t31.*t116;
t198 = t31.*t117;
t200 = t31.*t118;
t202 = t31.*t119;
t204 = t31.*t120;
t206 = t31.*t121;
t208 = t31.*t122;
t210 = t31.*t123;
t212 = t31.*t124;
t214 = t31.*t125;
t216 = t31.*t126;
t218 = t31.*t127;
t220 = t31.*t128;
t222 = t31.*t129;
t224 = t31.*t130;
t226 = t31.*t131;
t228 = t31.*t132;
t230 = t31.*t133;
t232 = t31.*t134;
t234 = t31.*t135;
t252 = t31.*t138;
t253 = t31.*t139;
t254 = t31.*t140;
t255 = t31.*t141;
t256 = t31.*t142;
t257 = t31.*t143;
t258 = t31.*t144;
t259 = t31.*t145;
t260 = t31.*t146;
t261 = t31.*t147;
t262 = t31.*t148;
t263 = t31.*t149;
t264 = t31.*t150;
t286 = (phi_dot.*t76)./7.5e+2;
t287 = (phi_dot.*t77)./7.5e+2;
t288 = (phi_dot.*t79)./7.5e+2;
t289 = (phi_dot.*t80)./7.5e+2;
t290 = (phi_dot.*t82)./7.5e+2;
t291 = (phi_dot.*t83)./7.5e+2;
t292 = (phi_dot.*t85)./7.5e+2;
t293 = (phi_dot.*t86)./7.5e+2;
t294 = (psi_dot.*t76)./7.5e+2;
t295 = (psi_dot.*t77)./7.5e+2;
t296 = (psi_dot.*t79)./7.5e+2;
t297 = (psi_dot.*t80)./7.5e+2;
t298 = (psi_dot.*t82)./7.5e+2;
t299 = (psi_dot.*t83)./7.5e+2;
t300 = (psi_dot.*t85)./7.5e+2;
t301 = (psi_dot.*t86)./7.5e+2;
t302 = -t185;
t303 = -t186;
t304 = -t236;
t305 = -t237;
t306 = -t238;
t307 = -t239;
t308 = -t240;
t309 = -t241;
t310 = -t242;
t311 = -t243;
t312 = -t244;
t313 = -t245;
t314 = -t246;
t315 = -t247;
t324 = -t265;
t329 = t19.*t74.*zeta_dot.*(3.0./5.0e+2);
t330 = t20.*t74.*zeta_dot.*(3.0./5.0e+2);
t331 = t21.*t74.*zeta_dot.*(3.0./5.0e+2);
t332 = t22.*t74.*zeta_dot.*(3.0./5.0e+2);
t333 = t23.*t74.*zeta_dot.*(3.0./5.0e+2);
t334 = t24.*t74.*zeta_dot.*(3.0./5.0e+2);
t335 = t25.*t74.*zeta_dot.*(3.0./5.0e+2);
t336 = t26.*t74.*zeta_dot.*(3.0./5.0e+2);
t337 = t27.*t74.*zeta_dot.*(3.0./5.0e+2);
t338 = t28.*t74.*zeta_dot.*(3.0./5.0e+2);
t339 = t29.*t74.*zeta_dot.*(3.0./5.0e+2);
t340 = t30.*t74.*zeta_dot.*(3.0./5.0e+2);
t342 = t3.*t189;
t344 = t3.*t195;
t346 = t3.*t201;
t348 = t3.*t207;
t349 = t31.*t185;
t446 = t31.*t266;
t447 = t31.*t267;
t448 = t31.*t268;
t449 = t31.*t269;
t450 = t31.*t270;
t451 = t31.*t271;
t452 = t31.*t272;
t453 = t31.*t273;
t454 = t31.*t274;
t455 = t31.*t275;
t456 = t31.*t276;
t457 = t31.*t277;
t458 = t31.*t278;
t459 = t31.*t279;
t460 = t31.*t280;
t461 = t31.*t281;
t470 = (phi_dot.*t16.*t48)./3.75e+2;
t471 = (phi_dot.*t16.*t51)./3.75e+2;
t472 = (phi_dot.*t16.*t54)./3.75e+2;
t473 = (phi_dot.*t16.*t57)./3.75e+2;
t474 = (psi_dot.*t16.*t48)./3.75e+2;
t475 = (psi_dot.*t16.*t51)./3.75e+2;
t476 = (psi_dot.*t16.*t54)./3.75e+2;
t477 = (psi_dot.*t16.*t57)./3.75e+2;
t478 = t4.*t47.*zeta_dot.*(3.0./5.0e+2);
t479 = t5.*t47.*zeta_dot.*(3.0./5.0e+2);
t480 = t6.*t47.*zeta_dot.*(3.0./5.0e+2);
t481 = t7.*t47.*zeta_dot.*(3.0./5.0e+2);
t482 = t8.*t47.*zeta_dot.*(3.0./5.0e+2);
t483 = t9.*t47.*zeta_dot.*(3.0./5.0e+2);
t484 = t10.*t47.*zeta_dot.*(3.0./5.0e+2);
t485 = t11.*t47.*zeta_dot.*(3.0./5.0e+2);
t486 = t12.*t47.*zeta_dot.*(3.0./5.0e+2);
t487 = t13.*t47.*zeta_dot.*(3.0./5.0e+2);
t488 = t14.*t47.*zeta_dot.*(3.0./5.0e+2);
t489 = t15.*t47.*zeta_dot.*(3.0./5.0e+2);
t490 = t61.*t136;
t491 = t60.*t137;
t492 = t62.*t136;
t493 = t64.*t136;
t494 = t63.*t137;
t495 = t65.*t136;
t496 = t67.*t136;
t497 = t66.*t137;
t498 = t68.*t136;
t499 = t70.*t136;
t500 = t69.*t137;
t501 = t71.*t136;
t502 = t48.*t138;
t503 = t49.*t139;
t504 = t50.*t140;
t505 = t51.*t141;
t506 = t52.*t142;
t507 = t53.*t143;
t508 = t54.*t144;
t509 = t55.*t145;
t510 = t56.*t146;
t511 = t57.*t147;
t512 = t58.*t148;
t513 = t59.*t149;
t514 = phi_dot.*t4.*t87.*(3.0./1.0e+2);
t515 = phi_dot.*t7.*t87.*(3.0./1.0e+2);
t516 = phi_dot.*t10.*t87.*(3.0./2.5e+2);
t517 = phi_dot.*t13.*t87.*(3.0./2.5e+2);
t518 = phi_dot.*t11.*t87.*(3.0./3.2e+2);
t519 = phi_dot.*t12.*t87.*(3.0./3.2e+2);
t520 = phi_dot.*t14.*t87.*(3.0./3.2e+2);
t521 = phi_dot.*t15.*t87.*(3.0./3.2e+2);
t522 = phi_dot.*t19.*t73.*(3.0./1.0e+2);
t523 = phi_dot.*t22.*t73.*(3.0./1.0e+2);
t524 = phi_dot.*t20.*t73.*(3.0./2.0e+2);
t525 = phi_dot.*t21.*t73.*(3.0./2.0e+2);
t526 = phi_dot.*t23.*t73.*(3.0./2.0e+2);
t527 = phi_dot.*t24.*t73.*(3.0./2.0e+2);
t528 = phi_dot.*t25.*t73.*(3.0./2.5e+2);
t529 = phi_dot.*t28.*t73.*(3.0./2.5e+2);
t530 = phi_dot.*t26.*t73.*(3.0./5.0e+2);
t531 = phi_dot.*t27.*t73.*(3.0./5.0e+2);
t532 = phi_dot.*t29.*t73.*(3.0./5.0e+2);
t533 = phi_dot.*t30.*t73.*(3.0./5.0e+2);
t534 = t48.*t150;
t535 = t51.*t150;
t536 = t54.*t150;
t537 = t57.*t150;
t538 = t61.*t150;
t539 = t62.*t150;
t540 = t64.*t150;
t541 = t65.*t150;
t542 = t67.*t150;
t543 = t68.*t150;
t544 = t70.*t150;
t545 = t71.*t150;
t546 = phi_dot.*t19.*t87.*(3.0./1.0e+3);
t547 = phi_dot.*t20.*t87.*(3.0./1.0e+3);
t548 = phi_dot.*t21.*t87.*(3.0./1.0e+3);
t549 = phi_dot.*t22.*t87.*(3.0./1.0e+3);
t550 = phi_dot.*t23.*t87.*(3.0./1.0e+3);
t551 = phi_dot.*t24.*t87.*(3.0./1.0e+3);
t552 = phi_dot.*t25.*t87.*(3.0./1.0e+3);
t553 = phi_dot.*t26.*t87.*(3.0./1.0e+3);
t554 = phi_dot.*t27.*t87.*(3.0./1.0e+3);
t555 = phi_dot.*t28.*t87.*(3.0./1.0e+3);
t556 = phi_dot.*t29.*t87.*(3.0./1.0e+3);
t557 = phi_dot.*t30.*t87.*(3.0./1.0e+3);
t584 = -t350;
t585 = -t381;
t586 = -t382;
t587 = -t383;
t588 = -t384;
t589 = -t385;
t590 = -t386;
t591 = -t387;
t592 = -t388;
t593 = -t389;
t594 = -t390;
t595 = -t391;
t596 = -t392;
t597 = -t393;
t600 = (phi_dot.*t16.*t49)./1.5e+3;
t601 = (phi_dot.*t16.*t50)./1.5e+3;
t602 = (phi_dot.*t16.*t52)./1.5e+3;
t603 = (phi_dot.*t16.*t53)./1.5e+3;
t604 = (phi_dot.*t16.*t55)./1.5e+3;
t605 = (phi_dot.*t16.*t56)./1.5e+3;
t606 = (phi_dot.*t16.*t58)./1.5e+3;
t607 = (phi_dot.*t16.*t59)./1.5e+3;
t608 = (psi_dot.*t16.*t49)./1.5e+3;
t609 = (psi_dot.*t16.*t50)./1.5e+3;
t610 = (psi_dot.*t16.*t52)./1.5e+3;
t611 = (psi_dot.*t16.*t53)./1.5e+3;
t612 = (psi_dot.*t16.*t55)./1.5e+3;
t613 = (psi_dot.*t16.*t56)./1.5e+3;
t614 = (psi_dot.*t16.*t58)./1.5e+3;
t615 = (psi_dot.*t16.*t59)./1.5e+3;
t616 = t18.*t48.*th11_dot.*(-2.0./3.75e+2);
t617 = t18.*t51.*th21_dot.*(-2.0./3.75e+2);
t618 = t18.*t54.*th31_dot.*(-2.0./3.75e+2);
t619 = t18.*t57.*th41_dot.*(-2.0./3.75e+2);
t620 = -t566;
t621 = t3.*t16.*t18.*t112;
t622 = t3.*t16.*t18.*t113;
t623 = t3.*t16.*t18.*t114;
t624 = t3.*t16.*t18.*t115;
t625 = t3.*t16.*t18.*t116;
t626 = t3.*t16.*t18.*t117;
t627 = t3.*t16.*t18.*t118;
t628 = t3.*t16.*t18.*t119;
t629 = t3.*t16.*t18.*t120;
t630 = t3.*t16.*t18.*t121;
t631 = t3.*t16.*t18.*t122;
t632 = t3.*t16.*t18.*t123;
t649 = (phi_dot.*t48.*t87)./2.5e+2;
t650 = (phi_dot.*t51.*t87)./2.5e+2;
t651 = (phi_dot.*t54.*t87)./2.5e+2;
t652 = (phi_dot.*t57.*t87)./2.5e+2;
t653 = (t48.*t74.*zeta_dot)./3.75e+2;
t654 = (t51.*t74.*zeta_dot)./3.75e+2;
t655 = (t54.*t74.*zeta_dot)./3.75e+2;
t656 = (t57.*t74.*zeta_dot)./3.75e+2;
t657 = (t16.*t89.*t92)./2.0;
t666 = (t16.*t91.*t92)./2.0;
t725 = t48.*t185;
t726 = t51.*t185;
t727 = t54.*t185;
t728 = t57.*t185;
t729 = t3.*t72.*t112;
t730 = t3.*t72.*t115;
t731 = t3.*t72.*t118;
t732 = t3.*t72.*t121;
t733 = t61.*t185;
t734 = t62.*t185;
t735 = t64.*t185;
t736 = t65.*t185;
t737 = t67.*t185;
t738 = t68.*t185;
t739 = t70.*t185;
t740 = t71.*t185;
t741 = t61.*t186;
t742 = t60.*t187;
t743 = t62.*t186;
t744 = t64.*t186;
t745 = t63.*t187;
t746 = t65.*t186;
t747 = t67.*t186;
t748 = t66.*t187;
t749 = t68.*t186;
t750 = t70.*t186;
t751 = t69.*t187;
t752 = t71.*t186;
t753 = t3.*t16.*t60.*th11_dot.*(4.0./3.75e+2);
t754 = t3.*t16.*t61.*th12_dot.*(2.0./3.75e+2);
t755 = t3.*t16.*t62.*th13_dot.*(2.0./3.75e+2);
t756 = t3.*t16.*t63.*th21_dot.*(4.0./3.75e+2);
t757 = t3.*t16.*t64.*th22_dot.*(2.0./3.75e+2);
t758 = t3.*t16.*t65.*th23_dot.*(2.0./3.75e+2);
t759 = t3.*t16.*t66.*th31_dot.*(4.0./3.75e+2);
t760 = t3.*t16.*t67.*th32_dot.*(2.0./3.75e+2);
t761 = t3.*t16.*t68.*th33_dot.*(2.0./3.75e+2);
t762 = t3.*t16.*t69.*th41_dot.*(4.0./3.75e+2);
t763 = t3.*t16.*t70.*th42_dot.*(2.0./3.75e+2);
t764 = t3.*t16.*t71.*th43_dot.*(2.0./3.75e+2);
t765 = phi_dot.*t3.*t19.*t72.*(3.0./1.0e+2);
t766 = phi_dot.*t3.*t22.*t72.*(3.0./1.0e+2);
t767 = phi_dot.*t3.*t25.*t72.*(3.0./2.5e+2);
C = ft_2({phi_dot,psi_dot,t10,t100,t101,t102,t103,t104,t105,t1066,t1067,t1068,t1069,t1070,t1071,t1072,t1073,t1074,t1075,t1076,t1077,t1090,t1091,t1092,t1093,t1094,t1095,t1096,t1097,t1098,t1099,t11,t1100,t1101,t1106,t1107,t1108,t1109,t1110,t1111,t1112,t1113,t1114,t1115,t1116,t1117,t112,t1122,t1123,t1124,t1125,t1126,t1127,t1128,t1129,t113,t1130,t1131,t1132,t1133,t1134,t1135,t1136,t1137,t114,t1146,t1147,t1148,t1149,t115,t1150,t1151,t1152,t1153,t116,t1162,t1163,t1166,t1167,t117,t1170,t1171,t1172,t1173,t118,t119,t12,t120,t121,t122,t123,t124,t125,t126,t127,t128,t129,t13,t130,t1308,t1309,t131,t1310,t1311,t1312,t1313,t1314,t1315,t132,t133,t1332,t1333,t1334,t1335,t1336,t1337,t1338,t1339,t134,t135,t136,t138,t139,t14,t140,t141,t142,t1428,t1429,t143,t1430,t1431,t1432,t1433,t1434,t1435,t1436,t1437,t1438,t1439,t144,t1440,t1441,t1442,t1443,t1444,t1445,t1446,t1447,t145,t146,t1460,t1461,t1462,t1463,t1464,t1465,t1466,t1467,t1468,t1469,t147,t1470,t1471,t1472,t1473,t1474,t1475,t1476,t1477,t1478,t1479,t148,t1480,t1481,t1482,t1483,t1484,t1485,t1486,t1487,t1488,t1489,t149,t1490,t1491,t1492,t1493,t1494,t1495,t1496,t1497,t1498,t1499,t15,t150,t151,t152,t153,t154,t155,t156,t157,t158,t159,t16,t160,t161,t162,t163,t164,t165,t166,t167,t168,t169,t17,t170,t171,t1711,t1712,t1713,t1714,t172,t1728,t173,t1730,t1732,t1734,t1736,t1738,t174,t1740,t1742,t1743,t1744,t1745,t1746,t1747,t1748,t1749,t175,t1750,t176,t177,t1775,t1776,t1777,t1778,t178,t1783,t1784,t1785,t1786,t1787,t1788,t1789,t179,t1790,t1791,t1792,t1793,t1794,t1795,t1796,t1797,t1798,t1799,t18,t180,t1800,t1801,t1802,t1803,t1804,t1805,t1806,t181,t182,t183,t184,t185,t1865,t1866,t1867,t1868,t187,t188,t189,t19,t190,t191,t192,t193,t194,t195,t196,t197,t198,t199,t1994,t1995,t1996,t1997,t1998,t1999,t2,t20,t200,t2000,t2001,t201,t202,t203,t2034,t2035,t2036,t2037,t2038,t2039,t204,t2040,t2041,t205,t206,t207,t208,t209,t21,t210,t211,t212,t213,t214,t215,t216,t217,t218,t219,t22,t220,t221,t222,t223,t224,t225,t226,t227,t228,t229,t23,t230,t231,t232,t233,t234,t235,t24,t248,t249,t25,t250,t251,t252,t253,t254,t255,t256,t257,t258,t259,t26,t260,t261,t262,t263,t264,t265,t266,t267,t268,t269,t27,t270,t271,t272,t273,t274,t275,t276,t277,t278,t279,t28,t280,t281,t282,t283,t284,t285,t286,t287,t288,t289,t29,t290,t291,t292,t293,t294,t295,t296,t297,t298,t299,t3,t30,t300,t301,t302,t303,t304,t305,t306,t307,t308,t309,t31,t310,t311,t312,t313,t314,t315,t316,t317,t318,t319,t320,t321,t322,t323,t324,t329,t330,t331,t332,t333,t334,t335,t336,t337,t338,t339,t340,t342,t344,t346,t348,t349,t350,t351,t352,t353,t354,t355,t356,t357,t358,t361,t362,t363,t364,t365,t366,t367,t368,t369,t370,t371,t372,t373,t374,t375,t376,t377,t378,t379,t380,t381,t394,t395,t396,t397,t398,t399,t4,t400,t401,t402,t403,t404,t405,t406,t407,t408,t409,t410,t411,t412,t413,t414,t415,t416,t417,t418,t419,t420,t421,t422,t423,t424,t425,t426,t427,t428,t429,t430,t431,t432,t433,t434,t435,t436,t437,t438,t439,t440,t441,t442,t443,t444,t445,t446,t447,t448,t449,t450,t451,t452,t453,t454,t455,t456,t457,t458,t459,t46,t460,t461,t462,t463,t464,t465,t466,t467,t468,t469,t47,t470,t471,t472,t473,t474,t475,t476,t477,t478,t479,t48,t480,t481,t482,t483,t484,t485,t486,t487,t488,t489,t49,t490,t491,t492,t493,t494,t495,t496,t497,t498,t499,t5,t50,t500,t501,t503,t504,t506,t507,t509,t51,t510,t512,t513,t514,t515,t516,t517,t518,t519,t52,t520,t521,t522,t523,t524,t525,t526,t527,t528,t529,t53,t530,t531,t532,t533,t534,t535,t536,t537,t538,t539,t54,t540,t541,t542,t543,t544,t545,t546,t547,t548,t549,t55,t550,t551,t552,t553,t554,t555,t556,t557,t558,t559,t56,t560,t561,t562,t563,t564,t565,t566,t567,t568,t569,t57,t570,t571,t572,t573,t574,t575,t576,t577,t578,t579,t58,t580,t581,t582,t583,t584,t585,t586,t587,t588,t589,t59,t590,t591,t592,t593,t594,t595,t596,t597,t598,t599,t6,t60,t600,t601,t602,t603,t604,t605,t606,t607,t608,t609,t61,t610,t611,t612,t613,t614,t615,t616,t617,t618,t619,t62,t620,t621,t622,t623,t624,t625,t626,t627,t628,t629,t63,t630,t631,t632,t633,t634,t635,t636,t637,t638,t639,t64,t640,t641,t642,t643,t644,t645,t646,t647,t648,t649,t65,t650,t651,t652,t653,t654,t655,t656,t657,t66,t666,t667,t668,t669,t67,t670,t671,t672,t673,t674,t675,t676,t677,t678,t679,t68,t680,t681,t682,t683,t684,t685,t686,t687,t688,t689,t69,t690,t691,t692,t693,t694,t695,t696,t697,t698,t699,t7,t70,t700,t701,t702,t703,t704,t705,t706,t707,t708,t709,t71,t710,t711,t712,t713,t714,t715,t716,t717,t718,t719,t72,t720,t721,t722,t725,t726,t727,t728,t729,t73,t730,t731,t732,t733,t734,t735,t736,t737,t738,t739,t74,t740,t741,t742,t743,t744,t745,t746,t747,t748,t749,t75,t750,t751,t752,t753,t754,t755,t756,t757,t758,t759,t76,t760,t761,t762,t763,t764,t765,t766,t767,t77,t78,t79,t8,t80,t81,t82,t83,t84,t85,t86,t87,t88,t89,t9,t90,t91,t917,t918,t919,t92,t920,t921,t922,t923,t924,t925,t926,t927,t928,t929,t93,t930,t931,t932,t935,t936,t937,t938,t939,t94,t940,t941,t942,t95,t96,t961,t963,t965,t967,t969,t97,t971,t973,t975,t976,t977,t978,t979,t98,t980,t981,t982,t983,t984,t985,t986,t987,t99,th11_dot,th12_dot,th13_dot,th21_dot,th22_dot,th23_dot,th31_dot,th32_dot,th33_dot,th41_dot,th42_dot,th43_dot,zeta_dot});
end
function C = ft_2(ct)
phi_dot = ct{1};
psi_dot = ct{2};
t10 = ct{3};
t100 = ct{4};
t101 = ct{5};
t102 = ct{6};
t103 = ct{7};
t104 = ct{8};
t105 = ct{9};
t1066 = ct{10};
t1067 = ct{11};
t1068 = ct{12};
t1069 = ct{13};
t1070 = ct{14};
t1071 = ct{15};
t1072 = ct{16};
t1073 = ct{17};
t1074 = ct{18};
t1075 = ct{19};
t1076 = ct{20};
t1077 = ct{21};
t1090 = ct{22};
t1091 = ct{23};
t1092 = ct{24};
t1093 = ct{25};
t1094 = ct{26};
t1095 = ct{27};
t1096 = ct{28};
t1097 = ct{29};
t1098 = ct{30};
t1099 = ct{31};
t11 = ct{32};
t1100 = ct{33};
t1101 = ct{34};
t1106 = ct{35};
t1107 = ct{36};
t1108 = ct{37};
t1109 = ct{38};
t1110 = ct{39};
t1111 = ct{40};
t1112 = ct{41};
t1113 = ct{42};
t1114 = ct{43};
t1115 = ct{44};
t1116 = ct{45};
t1117 = ct{46};
t112 = ct{47};
t1122 = ct{48};
t1123 = ct{49};
t1124 = ct{50};
t1125 = ct{51};
t1126 = ct{52};
t1127 = ct{53};
t1128 = ct{54};
t1129 = ct{55};
t113 = ct{56};
t1130 = ct{57};
t1131 = ct{58};
t1132 = ct{59};
t1133 = ct{60};
t1134 = ct{61};
t1135 = ct{62};
t1136 = ct{63};
t1137 = ct{64};
t114 = ct{65};
t1146 = ct{66};
t1147 = ct{67};
t1148 = ct{68};
t1149 = ct{69};
t115 = ct{70};
t1150 = ct{71};
t1151 = ct{72};
t1152 = ct{73};
t1153 = ct{74};
t116 = ct{75};
t1162 = ct{76};
t1163 = ct{77};
t1166 = ct{78};
t1167 = ct{79};
t117 = ct{80};
t1170 = ct{81};
t1171 = ct{82};
t1172 = ct{83};
t1173 = ct{84};
t118 = ct{85};
t119 = ct{86};
t12 = ct{87};
t120 = ct{88};
t121 = ct{89};
t122 = ct{90};
t123 = ct{91};
t124 = ct{92};
t125 = ct{93};
t126 = ct{94};
t127 = ct{95};
t128 = ct{96};
t129 = ct{97};
t13 = ct{98};
t130 = ct{99};
t1308 = ct{100};
t1309 = ct{101};
t131 = ct{102};
t1310 = ct{103};
t1311 = ct{104};
t1312 = ct{105};
t1313 = ct{106};
t1314 = ct{107};
t1315 = ct{108};
t132 = ct{109};
t133 = ct{110};
t1332 = ct{111};
t1333 = ct{112};
t1334 = ct{113};
t1335 = ct{114};
t1336 = ct{115};
t1337 = ct{116};
t1338 = ct{117};
t1339 = ct{118};
t134 = ct{119};
t135 = ct{120};
t136 = ct{121};
t138 = ct{122};
t139 = ct{123};
t14 = ct{124};
t140 = ct{125};
t141 = ct{126};
t142 = ct{127};
t1428 = ct{128};
t1429 = ct{129};
t143 = ct{130};
t1430 = ct{131};
t1431 = ct{132};
t1432 = ct{133};
t1433 = ct{134};
t1434 = ct{135};
t1435 = ct{136};
t1436 = ct{137};
t1437 = ct{138};
t1438 = ct{139};
t1439 = ct{140};
t144 = ct{141};
t1440 = ct{142};
t1441 = ct{143};
t1442 = ct{144};
t1443 = ct{145};
t1444 = ct{146};
t1445 = ct{147};
t1446 = ct{148};
t1447 = ct{149};
t145 = ct{150};
t146 = ct{151};
t1460 = ct{152};
t1461 = ct{153};
t1462 = ct{154};
t1463 = ct{155};
t1464 = ct{156};
t1465 = ct{157};
t1466 = ct{158};
t1467 = ct{159};
t1468 = ct{160};
t1469 = ct{161};
t147 = ct{162};
t1470 = ct{163};
t1471 = ct{164};
t1472 = ct{165};
t1473 = ct{166};
t1474 = ct{167};
t1475 = ct{168};
t1476 = ct{169};
t1477 = ct{170};
t1478 = ct{171};
t1479 = ct{172};
t148 = ct{173};
t1480 = ct{174};
t1481 = ct{175};
t1482 = ct{176};
t1483 = ct{177};
t1484 = ct{178};
t1485 = ct{179};
t1486 = ct{180};
t1487 = ct{181};
t1488 = ct{182};
t1489 = ct{183};
t149 = ct{184};
t1490 = ct{185};
t1491 = ct{186};
t1492 = ct{187};
t1493 = ct{188};
t1494 = ct{189};
t1495 = ct{190};
t1496 = ct{191};
t1497 = ct{192};
t1498 = ct{193};
t1499 = ct{194};
t15 = ct{195};
t150 = ct{196};
t151 = ct{197};
t152 = ct{198};
t153 = ct{199};
t154 = ct{200};
t155 = ct{201};
t156 = ct{202};
t157 = ct{203};
t158 = ct{204};
t159 = ct{205};
t16 = ct{206};
t160 = ct{207};
t161 = ct{208};
t162 = ct{209};
t163 = ct{210};
t164 = ct{211};
t165 = ct{212};
t166 = ct{213};
t167 = ct{214};
t168 = ct{215};
t169 = ct{216};
t17 = ct{217};
t170 = ct{218};
t171 = ct{219};
t1711 = ct{220};
t1712 = ct{221};
t1713 = ct{222};
t1714 = ct{223};
t172 = ct{224};
t1728 = ct{225};
t173 = ct{226};
t1730 = ct{227};
t1732 = ct{228};
t1734 = ct{229};
t1736 = ct{230};
t1738 = ct{231};
t174 = ct{232};
t1740 = ct{233};
t1742 = ct{234};
t1743 = ct{235};
t1744 = ct{236};
t1745 = ct{237};
t1746 = ct{238};
t1747 = ct{239};
t1748 = ct{240};
t1749 = ct{241};
t175 = ct{242};
t1750 = ct{243};
t176 = ct{244};
t177 = ct{245};
t1775 = ct{246};
t1776 = ct{247};
t1777 = ct{248};
t1778 = ct{249};
t178 = ct{250};
t1783 = ct{251};
t1784 = ct{252};
t1785 = ct{253};
t1786 = ct{254};
t1787 = ct{255};
t1788 = ct{256};
t1789 = ct{257};
t179 = ct{258};
t1790 = ct{259};
t1791 = ct{260};
t1792 = ct{261};
t1793 = ct{262};
t1794 = ct{263};
t1795 = ct{264};
t1796 = ct{265};
t1797 = ct{266};
t1798 = ct{267};
t1799 = ct{268};
t18 = ct{269};
t180 = ct{270};
t1800 = ct{271};
t1801 = ct{272};
t1802 = ct{273};
t1803 = ct{274};
t1804 = ct{275};
t1805 = ct{276};
t1806 = ct{277};
t181 = ct{278};
t182 = ct{279};
t183 = ct{280};
t184 = ct{281};
t185 = ct{282};
t1865 = ct{283};
t1866 = ct{284};
t1867 = ct{285};
t1868 = ct{286};
t187 = ct{287};
t188 = ct{288};
t189 = ct{289};
t19 = ct{290};
t190 = ct{291};
t191 = ct{292};
t192 = ct{293};
t193 = ct{294};
t194 = ct{295};
t195 = ct{296};
t196 = ct{297};
t197 = ct{298};
t198 = ct{299};
t199 = ct{300};
t1994 = ct{301};
t1995 = ct{302};
t1996 = ct{303};
t1997 = ct{304};
t1998 = ct{305};
t1999 = ct{306};
t2 = ct{307};
t20 = ct{308};
t200 = ct{309};
t2000 = ct{310};
t2001 = ct{311};
t201 = ct{312};
t202 = ct{313};
t203 = ct{314};
t2034 = ct{315};
t2035 = ct{316};
t2036 = ct{317};
t2037 = ct{318};
t2038 = ct{319};
t2039 = ct{320};
t204 = ct{321};
t2040 = ct{322};
t2041 = ct{323};
t205 = ct{324};
t206 = ct{325};
t207 = ct{326};
t208 = ct{327};
t209 = ct{328};
t21 = ct{329};
t210 = ct{330};
t211 = ct{331};
t212 = ct{332};
t213 = ct{333};
t214 = ct{334};
t215 = ct{335};
t216 = ct{336};
t217 = ct{337};
t218 = ct{338};
t219 = ct{339};
t22 = ct{340};
t220 = ct{341};
t221 = ct{342};
t222 = ct{343};
t223 = ct{344};
t224 = ct{345};
t225 = ct{346};
t226 = ct{347};
t227 = ct{348};
t228 = ct{349};
t229 = ct{350};
t23 = ct{351};
t230 = ct{352};
t231 = ct{353};
t232 = ct{354};
t233 = ct{355};
t234 = ct{356};
t235 = ct{357};
t24 = ct{358};
t248 = ct{359};
t249 = ct{360};
t25 = ct{361};
t250 = ct{362};
t251 = ct{363};
t252 = ct{364};
t253 = ct{365};
t254 = ct{366};
t255 = ct{367};
t256 = ct{368};
t257 = ct{369};
t258 = ct{370};
t259 = ct{371};
t26 = ct{372};
t260 = ct{373};
t261 = ct{374};
t262 = ct{375};
t263 = ct{376};
t264 = ct{377};
t265 = ct{378};
t266 = ct{379};
t267 = ct{380};
t268 = ct{381};
t269 = ct{382};
t27 = ct{383};
t270 = ct{384};
t271 = ct{385};
t272 = ct{386};
t273 = ct{387};
t274 = ct{388};
t275 = ct{389};
t276 = ct{390};
t277 = ct{391};
t278 = ct{392};
t279 = ct{393};
t28 = ct{394};
t280 = ct{395};
t281 = ct{396};
t282 = ct{397};
t283 = ct{398};
t284 = ct{399};
t285 = ct{400};
t286 = ct{401};
t287 = ct{402};
t288 = ct{403};
t289 = ct{404};
t29 = ct{405};
t290 = ct{406};
t291 = ct{407};
t292 = ct{408};
t293 = ct{409};
t294 = ct{410};
t295 = ct{411};
t296 = ct{412};
t297 = ct{413};
t298 = ct{414};
t299 = ct{415};
t3 = ct{416};
t30 = ct{417};
t300 = ct{418};
t301 = ct{419};
t302 = ct{420};
t303 = ct{421};
t304 = ct{422};
t305 = ct{423};
t306 = ct{424};
t307 = ct{425};
t308 = ct{426};
t309 = ct{427};
t31 = ct{428};
t310 = ct{429};
t311 = ct{430};
t312 = ct{431};
t313 = ct{432};
t314 = ct{433};
t315 = ct{434};
t316 = ct{435};
t317 = ct{436};
t318 = ct{437};
t319 = ct{438};
t320 = ct{439};
t321 = ct{440};
t322 = ct{441};
t323 = ct{442};
t324 = ct{443};
t329 = ct{444};
t330 = ct{445};
t331 = ct{446};
t332 = ct{447};
t333 = ct{448};
t334 = ct{449};
t335 = ct{450};
t336 = ct{451};
t337 = ct{452};
t338 = ct{453};
t339 = ct{454};
t340 = ct{455};
t342 = ct{456};
t344 = ct{457};
t346 = ct{458};
t348 = ct{459};
t349 = ct{460};
t350 = ct{461};
t351 = ct{462};
t352 = ct{463};
t353 = ct{464};
t354 = ct{465};
t355 = ct{466};
t356 = ct{467};
t357 = ct{468};
t358 = ct{469};
t361 = ct{470};
t362 = ct{471};
t363 = ct{472};
t364 = ct{473};
t365 = ct{474};
t366 = ct{475};
t367 = ct{476};
t368 = ct{477};
t369 = ct{478};
t370 = ct{479};
t371 = ct{480};
t372 = ct{481};
t373 = ct{482};
t374 = ct{483};
t375 = ct{484};
t376 = ct{485};
t377 = ct{486};
t378 = ct{487};
t379 = ct{488};
t380 = ct{489};
t381 = ct{490};
t394 = ct{491};
t395 = ct{492};
t396 = ct{493};
t397 = ct{494};
t398 = ct{495};
t399 = ct{496};
t4 = ct{497};
t400 = ct{498};
t401 = ct{499};
t402 = ct{500};
t403 = ct{501};
t404 = ct{502};
t405 = ct{503};
t406 = ct{504};
t407 = ct{505};
t408 = ct{506};
t409 = ct{507};
t410 = ct{508};
t411 = ct{509};
t412 = ct{510};
t413 = ct{511};
t414 = ct{512};
t415 = ct{513};
t416 = ct{514};
t417 = ct{515};
t418 = ct{516};
t419 = ct{517};
t420 = ct{518};
t421 = ct{519};
t422 = ct{520};
t423 = ct{521};
t424 = ct{522};
t425 = ct{523};
t426 = ct{524};
t427 = ct{525};
t428 = ct{526};
t429 = ct{527};
t430 = ct{528};
t431 = ct{529};
t432 = ct{530};
t433 = ct{531};
t434 = ct{532};
t435 = ct{533};
t436 = ct{534};
t437 = ct{535};
t438 = ct{536};
t439 = ct{537};
t440 = ct{538};
t441 = ct{539};
t442 = ct{540};
t443 = ct{541};
t444 = ct{542};
t445 = ct{543};
t446 = ct{544};
t447 = ct{545};
t448 = ct{546};
t449 = ct{547};
t450 = ct{548};
t451 = ct{549};
t452 = ct{550};
t453 = ct{551};
t454 = ct{552};
t455 = ct{553};
t456 = ct{554};
t457 = ct{555};
t458 = ct{556};
t459 = ct{557};
t46 = ct{558};
t460 = ct{559};
t461 = ct{560};
t462 = ct{561};
t463 = ct{562};
t464 = ct{563};
t465 = ct{564};
t466 = ct{565};
t467 = ct{566};
t468 = ct{567};
t469 = ct{568};
t47 = ct{569};
t470 = ct{570};
t471 = ct{571};
t472 = ct{572};
t473 = ct{573};
t474 = ct{574};
t475 = ct{575};
t476 = ct{576};
t477 = ct{577};
t478 = ct{578};
t479 = ct{579};
t48 = ct{580};
t480 = ct{581};
t481 = ct{582};
t482 = ct{583};
t483 = ct{584};
t484 = ct{585};
t485 = ct{586};
t486 = ct{587};
t487 = ct{588};
t488 = ct{589};
t489 = ct{590};
t49 = ct{591};
t490 = ct{592};
t491 = ct{593};
t492 = ct{594};
t493 = ct{595};
t494 = ct{596};
t495 = ct{597};
t496 = ct{598};
t497 = ct{599};
t498 = ct{600};
t499 = ct{601};
t5 = ct{602};
t50 = ct{603};
t500 = ct{604};
t501 = ct{605};
t503 = ct{606};
t504 = ct{607};
t506 = ct{608};
t507 = ct{609};
t509 = ct{610};
t51 = ct{611};
t510 = ct{612};
t512 = ct{613};
t513 = ct{614};
t514 = ct{615};
t515 = ct{616};
t516 = ct{617};
t517 = ct{618};
t518 = ct{619};
t519 = ct{620};
t52 = ct{621};
t520 = ct{622};
t521 = ct{623};
t522 = ct{624};
t523 = ct{625};
t524 = ct{626};
t525 = ct{627};
t526 = ct{628};
t527 = ct{629};
t528 = ct{630};
t529 = ct{631};
t53 = ct{632};
t530 = ct{633};
t531 = ct{634};
t532 = ct{635};
t533 = ct{636};
t534 = ct{637};
t535 = ct{638};
t536 = ct{639};
t537 = ct{640};
t538 = ct{641};
t539 = ct{642};
t54 = ct{643};
t540 = ct{644};
t541 = ct{645};
t542 = ct{646};
t543 = ct{647};
t544 = ct{648};
t545 = ct{649};
t546 = ct{650};
t547 = ct{651};
t548 = ct{652};
t549 = ct{653};
t55 = ct{654};
t550 = ct{655};
t551 = ct{656};
t552 = ct{657};
t553 = ct{658};
t554 = ct{659};
t555 = ct{660};
t556 = ct{661};
t557 = ct{662};
t558 = ct{663};
t559 = ct{664};
t56 = ct{665};
t560 = ct{666};
t561 = ct{667};
t562 = ct{668};
t563 = ct{669};
t564 = ct{670};
t565 = ct{671};
t566 = ct{672};
t567 = ct{673};
t568 = ct{674};
t569 = ct{675};
t57 = ct{676};
t570 = ct{677};
t571 = ct{678};
t572 = ct{679};
t573 = ct{680};
t574 = ct{681};
t575 = ct{682};
t576 = ct{683};
t577 = ct{684};
t578 = ct{685};
t579 = ct{686};
t58 = ct{687};
t580 = ct{688};
t581 = ct{689};
t582 = ct{690};
t583 = ct{691};
t584 = ct{692};
t585 = ct{693};
t586 = ct{694};
t587 = ct{695};
t588 = ct{696};
t589 = ct{697};
t59 = ct{698};
t590 = ct{699};
t591 = ct{700};
t592 = ct{701};
t593 = ct{702};
t594 = ct{703};
t595 = ct{704};
t596 = ct{705};
t597 = ct{706};
t598 = ct{707};
t599 = ct{708};
t6 = ct{709};
t60 = ct{710};
t600 = ct{711};
t601 = ct{712};
t602 = ct{713};
t603 = ct{714};
t604 = ct{715};
t605 = ct{716};
t606 = ct{717};
t607 = ct{718};
t608 = ct{719};
t609 = ct{720};
t61 = ct{721};
t610 = ct{722};
t611 = ct{723};
t612 = ct{724};
t613 = ct{725};
t614 = ct{726};
t615 = ct{727};
t616 = ct{728};
t617 = ct{729};
t618 = ct{730};
t619 = ct{731};
t62 = ct{732};
t620 = ct{733};
t621 = ct{734};
t622 = ct{735};
t623 = ct{736};
t624 = ct{737};
t625 = ct{738};
t626 = ct{739};
t627 = ct{740};
t628 = ct{741};
t629 = ct{742};
t63 = ct{743};
t630 = ct{744};
t631 = ct{745};
t632 = ct{746};
t633 = ct{747};
t634 = ct{748};
t635 = ct{749};
t636 = ct{750};
t637 = ct{751};
t638 = ct{752};
t639 = ct{753};
t64 = ct{754};
t640 = ct{755};
t641 = ct{756};
t642 = ct{757};
t643 = ct{758};
t644 = ct{759};
t645 = ct{760};
t646 = ct{761};
t647 = ct{762};
t648 = ct{763};
t649 = ct{764};
t65 = ct{765};
t650 = ct{766};
t651 = ct{767};
t652 = ct{768};
t653 = ct{769};
t654 = ct{770};
t655 = ct{771};
t656 = ct{772};
t657 = ct{773};
t66 = ct{774};
t666 = ct{775};
t667 = ct{776};
t668 = ct{777};
t669 = ct{778};
t67 = ct{779};
t670 = ct{780};
t671 = ct{781};
t672 = ct{782};
t673 = ct{783};
t674 = ct{784};
t675 = ct{785};
t676 = ct{786};
t677 = ct{787};
t678 = ct{788};
t679 = ct{789};
t68 = ct{790};
t680 = ct{791};
t681 = ct{792};
t682 = ct{793};
t683 = ct{794};
t684 = ct{795};
t685 = ct{796};
t686 = ct{797};
t687 = ct{798};
t688 = ct{799};
t689 = ct{800};
t69 = ct{801};
t690 = ct{802};
t691 = ct{803};
t692 = ct{804};
t693 = ct{805};
t694 = ct{806};
t695 = ct{807};
t696 = ct{808};
t697 = ct{809};
t698 = ct{810};
t699 = ct{811};
t7 = ct{812};
t70 = ct{813};
t700 = ct{814};
t701 = ct{815};
t702 = ct{816};
t703 = ct{817};
t704 = ct{818};
t705 = ct{819};
t706 = ct{820};
t707 = ct{821};
t708 = ct{822};
t709 = ct{823};
t71 = ct{824};
t710 = ct{825};
t711 = ct{826};
t712 = ct{827};
t713 = ct{828};
t714 = ct{829};
t715 = ct{830};
t716 = ct{831};
t717 = ct{832};
t718 = ct{833};
t719 = ct{834};
t72 = ct{835};
t720 = ct{836};
t721 = ct{837};
t722 = ct{838};
t725 = ct{839};
t726 = ct{840};
t727 = ct{841};
t728 = ct{842};
t729 = ct{843};
t73 = ct{844};
t730 = ct{845};
t731 = ct{846};
t732 = ct{847};
t733 = ct{848};
t734 = ct{849};
t735 = ct{850};
t736 = ct{851};
t737 = ct{852};
t738 = ct{853};
t739 = ct{854};
t74 = ct{855};
t740 = ct{856};
t741 = ct{857};
t742 = ct{858};
t743 = ct{859};
t744 = ct{860};
t745 = ct{861};
t746 = ct{862};
t747 = ct{863};
t748 = ct{864};
t749 = ct{865};
t75 = ct{866};
t750 = ct{867};
t751 = ct{868};
t752 = ct{869};
t753 = ct{870};
t754 = ct{871};
t755 = ct{872};
t756 = ct{873};
t757 = ct{874};
t758 = ct{875};
t759 = ct{876};
t76 = ct{877};
t760 = ct{878};
t761 = ct{879};
t762 = ct{880};
t763 = ct{881};
t764 = ct{882};
t765 = ct{883};
t766 = ct{884};
t767 = ct{885};
t77 = ct{886};
t78 = ct{887};
t79 = ct{888};
t8 = ct{889};
t80 = ct{890};
t81 = ct{891};
t82 = ct{892};
t83 = ct{893};
t84 = ct{894};
t85 = ct{895};
t86 = ct{896};
t87 = ct{897};
t88 = ct{898};
t89 = ct{899};
t9 = ct{900};
t90 = ct{901};
t91 = ct{902};
t917 = ct{903};
t918 = ct{904};
t919 = ct{905};
t92 = ct{906};
t920 = ct{907};
t921 = ct{908};
t922 = ct{909};
t923 = ct{910};
t924 = ct{911};
t925 = ct{912};
t926 = ct{913};
t927 = ct{914};
t928 = ct{915};
t929 = ct{916};
t93 = ct{917};
t930 = ct{918};
t931 = ct{919};
t932 = ct{920};
t935 = ct{921};
t936 = ct{922};
t937 = ct{923};
t938 = ct{924};
t939 = ct{925};
t94 = ct{926};
t940 = ct{927};
t941 = ct{928};
t942 = ct{929};
t95 = ct{930};
t96 = ct{931};
t961 = ct{932};
t963 = ct{933};
t965 = ct{934};
t967 = ct{935};
t969 = ct{936};
t97 = ct{937};
t971 = ct{938};
t973 = ct{939};
t975 = ct{940};
t976 = ct{941};
t977 = ct{942};
t978 = ct{943};
t979 = ct{944};
t98 = ct{945};
t980 = ct{946};
t981 = ct{947};
t982 = ct{948};
t983 = ct{949};
t984 = ct{950};
t985 = ct{951};
t986 = ct{952};
t987 = ct{953};
t99 = ct{954};
th11_dot = ct{955};
th12_dot = ct{956};
th13_dot = ct{957};
th21_dot = ct{958};
th22_dot = ct{959};
th23_dot = ct{960};
th31_dot = ct{961};
th32_dot = ct{962};
th33_dot = ct{963};
th41_dot = ct{964};
th42_dot = ct{965};
th43_dot = ct{966};
zeta_dot = ct{967};
t768 = phi_dot.*t3.*t28.*t72.*(3.0./2.5e+2);
t769 = t46.*t189;
t770 = t46.*t191;
t771 = t46.*t193;
t772 = t46.*t195;
t773 = t46.*t197;
t774 = t46.*t199;
t775 = t46.*t201;
t776 = t46.*t203;
t777 = t46.*t205;
t778 = t46.*t207;
t779 = t46.*t209;
t780 = t46.*t211;
t781 = t46.*t213;
t782 = t46.*t215;
t783 = t46.*t217;
t784 = t46.*t219;
t785 = t46.*t221;
t786 = t46.*t223;
t787 = t46.*t225;
t788 = t46.*t227;
t789 = t46.*t229;
t790 = t46.*t231;
t791 = t46.*t233;
t792 = t46.*t235;
t793 = phi_dot.*t4.*t19.*t73.*(4.0./3.75e+2);
t794 = phi_dot.*t5.*t20.*t73.*(2.0./3.75e+2);
t795 = phi_dot.*t6.*t21.*t73.*(2.0./3.75e+2);
t796 = phi_dot.*t7.*t22.*t73.*(4.0./3.75e+2);
t797 = phi_dot.*t8.*t23.*t73.*(2.0./3.75e+2);
t798 = phi_dot.*t9.*t24.*t73.*(2.0./3.75e+2);
t799 = phi_dot.*t10.*t25.*t73.*(4.0./3.75e+2);
t800 = phi_dot.*t11.*t26.*t73.*(2.0./3.75e+2);
t801 = phi_dot.*t12.*t27.*t73.*(2.0./3.75e+2);
t802 = phi_dot.*t13.*t28.*t73.*(4.0./3.75e+2);
t803 = phi_dot.*t14.*t29.*t73.*(2.0./3.75e+2);
t804 = phi_dot.*t15.*t30.*t73.*(2.0./3.75e+2);
t805 = t4.*t19.*t47.*zeta_dot.*(4.0./3.75e+2);
t806 = t5.*t20.*t47.*zeta_dot.*(7.0./3.75e+2);
t807 = t6.*t21.*t47.*zeta_dot.*(7.0./3.75e+2);
t808 = t7.*t22.*t47.*zeta_dot.*(4.0./3.75e+2);
t809 = t8.*t23.*t47.*zeta_dot.*(7.0./3.75e+2);
t810 = t9.*t24.*t47.*zeta_dot.*(7.0./3.75e+2);
t811 = t10.*t25.*t47.*zeta_dot.*(4.0./3.75e+2);
t812 = t11.*t26.*t47.*zeta_dot.*(7.0./3.75e+2);
t813 = t12.*t27.*t47.*zeta_dot.*(7.0./3.75e+2);
t814 = t13.*t28.*t47.*zeta_dot.*(4.0./3.75e+2);
t815 = t14.*t29.*t47.*zeta_dot.*(7.0./3.75e+2);
t816 = t15.*t30.*t47.*zeta_dot.*(7.0./3.75e+2);
t817 = t16.*t19.*t47.*zeta_dot.*(3.0./2.5e+2);
t818 = t16.*t20.*t47.*zeta_dot.*(3.0./2.5e+2);
t819 = t16.*t21.*t47.*zeta_dot.*(3.0./2.5e+2);
t820 = t16.*t22.*t47.*zeta_dot.*(3.0./2.5e+2);
t821 = t16.*t23.*t47.*zeta_dot.*(3.0./2.5e+2);
t822 = t16.*t24.*t47.*zeta_dot.*(3.0./2.5e+2);
t823 = t16.*t47.*t153;
t824 = t16.*t26.*t47.*zeta_dot.*(3.0./2.5e+2);
t825 = t16.*t27.*t47.*zeta_dot.*(3.0./2.5e+2);
t826 = t16.*t47.*t154;
t827 = t16.*t29.*t47.*zeta_dot.*(3.0./2.5e+2);
t828 = t16.*t30.*t47.*zeta_dot.*(3.0./2.5e+2);
t830 = (phi_dot.*t3.*t31.*t76)./3.75e+2;
t831 = (phi_dot.*t3.*t31.*t77)./3.75e+2;
t833 = (phi_dot.*t3.*t31.*t79)./3.75e+2;
t834 = (phi_dot.*t3.*t31.*t80)./3.75e+2;
t836 = (phi_dot.*t3.*t31.*t82)./3.75e+2;
t837 = (phi_dot.*t3.*t31.*t83)./3.75e+2;
t839 = (phi_dot.*t3.*t31.*t85)./3.75e+2;
t840 = (phi_dot.*t3.*t31.*t86)./3.75e+2;
t841 = phi_dot.*t18.*t31.*t61.*(2.0./3.75e+2);
t842 = phi_dot.*t18.*t31.*t60.*(4.0./3.75e+2);
t843 = phi_dot.*t18.*t31.*t62.*(2.0./3.75e+2);
t844 = phi_dot.*t18.*t31.*t64.*(2.0./3.75e+2);
t845 = phi_dot.*t18.*t31.*t63.*(4.0./3.75e+2);
t846 = phi_dot.*t18.*t31.*t65.*(2.0./3.75e+2);
t847 = phi_dot.*t18.*t31.*t67.*(2.0./3.75e+2);
t848 = phi_dot.*t18.*t31.*t66.*(4.0./3.75e+2);
t849 = phi_dot.*t18.*t31.*t68.*(2.0./3.75e+2);
t850 = phi_dot.*t18.*t31.*t70.*(2.0./3.75e+2);
t851 = phi_dot.*t18.*t31.*t69.*(4.0./3.75e+2);
t852 = phi_dot.*t18.*t31.*t71.*(2.0./3.75e+2);
t866 = t60.*t265;
t869 = t63.*t265;
t872 = t66.*t265;
t875 = t69.*t265;
t877 = phi_dot.*t19.*t73.*(2.1e+1./1.0e+3);
t878 = phi_dot.*t20.*t73.*(2.1e+1./1.0e+3);
t879 = phi_dot.*t21.*t73.*(2.1e+1./1.0e+3);
t880 = phi_dot.*t22.*t73.*(2.1e+1./1.0e+3);
t881 = phi_dot.*t23.*t73.*(2.1e+1./1.0e+3);
t882 = phi_dot.*t24.*t73.*(2.1e+1./1.0e+3);
t883 = phi_dot.*t25.*t73.*(2.1e+1./1.0e+3);
t884 = phi_dot.*t26.*t73.*(2.1e+1./1.0e+3);
t885 = phi_dot.*t27.*t73.*(2.1e+1./1.0e+3);
t886 = phi_dot.*t28.*t73.*(2.1e+1./1.0e+3);
t887 = phi_dot.*t29.*t73.*(2.1e+1./1.0e+3);
t888 = phi_dot.*t30.*t73.*(2.1e+1./1.0e+3);
t889 = t19.*t46.*zeta_dot.*(2.1e+1./1.0e+3);
t890 = t20.*t46.*zeta_dot.*(2.1e+1./1.0e+3);
t891 = t21.*t46.*zeta_dot.*(2.1e+1./1.0e+3);
t892 = t22.*t46.*zeta_dot.*(2.1e+1./1.0e+3);
t893 = t23.*t46.*zeta_dot.*(2.1e+1./1.0e+3);
t894 = t24.*t46.*zeta_dot.*(2.1e+1./1.0e+3);
t895 = t25.*t46.*zeta_dot.*(2.1e+1./1.0e+3);
t896 = t26.*t46.*zeta_dot.*(2.1e+1./1.0e+3);
t897 = t27.*t46.*zeta_dot.*(2.1e+1./1.0e+3);
t898 = t28.*t46.*zeta_dot.*(2.1e+1./1.0e+3);
t899 = t29.*t46.*zeta_dot.*(2.1e+1./1.0e+3);
t900 = t30.*t46.*zeta_dot.*(2.1e+1./1.0e+3);
t901 = t5.*t74.*zeta_dot.*6.75e-3;
t902 = t6.*t74.*zeta_dot.*6.75e-3;
t903 = t8.*t74.*zeta_dot.*6.75e-3;
t904 = t9.*t74.*zeta_dot.*6.75e-3;
t905 = t11.*t74.*zeta_dot.*6.75e-3;
t906 = t12.*t74.*zeta_dot.*6.75e-3;
t907 = t14.*t74.*zeta_dot.*6.75e-3;
t908 = t15.*t74.*zeta_dot.*6.75e-3;
t909 = t20.*t47.*zeta_dot.*6.75e-3;
t910 = t21.*t47.*zeta_dot.*6.75e-3;
t911 = t23.*t47.*zeta_dot.*6.75e-3;
t912 = t24.*t47.*zeta_dot.*6.75e-3;
t913 = t26.*t47.*zeta_dot.*6.75e-3;
t914 = t27.*t47.*zeta_dot.*6.75e-3;
t915 = t29.*t47.*zeta_dot.*6.75e-3;
t916 = t30.*t47.*zeta_dot.*6.75e-3;
t933 = phi_dot.*t87.*1.5428125e-1;
t934 = t74.*zeta_dot.*3.085625e-1;
t943 = (phi_dot.*t49.*t87)./1.0e+3;
t944 = (phi_dot.*t50.*t87)./1.0e+3;
t945 = (phi_dot.*t52.*t87)./1.0e+3;
t946 = (phi_dot.*t53.*t87)./1.0e+3;
t947 = (phi_dot.*t55.*t87)./1.0e+3;
t948 = (phi_dot.*t56.*t87)./1.0e+3;
t949 = (phi_dot.*t58.*t87)./1.0e+3;
t950 = (phi_dot.*t59.*t87)./1.0e+3;
t951 = t49.*t74.*zeta_dot.*4.666666666666667e-3;
t952 = t50.*t74.*zeta_dot.*4.666666666666667e-3;
t953 = t52.*t74.*zeta_dot.*4.666666666666667e-3;
t954 = t53.*t74.*zeta_dot.*4.666666666666667e-3;
t955 = t55.*t74.*zeta_dot.*4.666666666666667e-3;
t956 = t56.*t74.*zeta_dot.*4.666666666666667e-3;
t957 = t58.*t74.*zeta_dot.*4.666666666666667e-3;
t958 = t59.*t74.*zeta_dot.*4.666666666666667e-3;
t960 = t31.*t568;
t962 = t31.*t570;
t964 = t31.*t572;
t966 = t31.*t574;
t968 = t31.*t576;
t970 = t31.*t578;
t972 = t31.*t580;
t974 = t31.*t582;
t989 = (t74.*t92.*zeta_dot)./3.75e+2;
t994 = phi_dot.*t3.*t5.*t72.*(3.0./1.0e+3);
t995 = phi_dot.*t3.*t6.*t72.*(3.0./1.0e+3);
t996 = phi_dot.*t3.*t8.*t72.*(3.0./1.0e+3);
t997 = phi_dot.*t3.*t9.*t72.*(3.0./1.0e+3);
t998 = phi_dot.*t3.*t11.*t72.*(3.0./1.0e+3);
t999 = phi_dot.*t3.*t12.*t72.*(3.0./1.0e+3);
t1000 = phi_dot.*t3.*t14.*t72.*(3.0./1.0e+3);
t1001 = phi_dot.*t3.*t15.*t72.*(3.0./1.0e+3);
t1010 = t4.*t16.*t74.*th11_dot.*(3.0./1.0e+3);
t1011 = t5.*t16.*t74.*th12_dot.*(3.0./1.0e+3);
t1012 = t6.*t16.*t74.*th13_dot.*(3.0./1.0e+3);
t1013 = t7.*t16.*t74.*th21_dot.*(3.0./1.0e+3);
t1014 = t8.*t16.*t74.*th22_dot.*(3.0./1.0e+3);
t1015 = t9.*t16.*t74.*th23_dot.*(3.0./1.0e+3);
t1016 = t10.*t16.*t74.*th31_dot.*(3.0./1.0e+3);
t1017 = t11.*t16.*t74.*th32_dot.*(3.0./1.0e+3);
t1018 = t12.*t16.*t74.*th33_dot.*(3.0./1.0e+3);
t1019 = t13.*t16.*t74.*th41_dot.*(3.0./1.0e+3);
t1020 = t14.*t16.*t74.*th42_dot.*(3.0./1.0e+3);
t1021 = t15.*t16.*t74.*th43_dot.*(3.0./1.0e+3);
t1022 = t18.*t31.*t49.*th12_dot.*(-1.0./3.75e+2);
t1023 = t18.*t31.*t50.*th13_dot.*(-1.0./3.75e+2);
t1024 = t18.*t31.*t52.*th22_dot.*(-1.0./3.75e+2);
t1025 = t18.*t31.*t53.*th23_dot.*(-1.0./3.75e+2);
t1026 = t18.*t31.*t55.*th32_dot.*(-1.0./3.75e+2);
t1027 = t18.*t31.*t56.*th33_dot.*(-1.0./3.75e+2);
t1028 = t18.*t31.*t58.*th42_dot.*(-1.0./3.75e+2);
t1029 = t18.*t31.*t59.*th43_dot.*(-1.0./3.75e+2);
t1030 = phi_dot.*t5.*t87.*1.1625e-2;
t1031 = phi_dot.*t6.*t87.*1.1625e-2;
t1032 = phi_dot.*t8.*t87.*1.1625e-2;
t1033 = phi_dot.*t9.*t87.*1.1625e-2;
t1038 = t47.*t73.*t112;
t1039 = t47.*t73.*t113;
t1040 = t47.*t73.*t114;
t1041 = t47.*t73.*t115;
t1042 = t47.*t73.*t116;
t1043 = t47.*t73.*t117;
t1044 = t47.*t73.*t118;
t1045 = t47.*t73.*t119;
t1046 = t47.*t73.*t120;
t1047 = t47.*t73.*t121;
t1048 = t47.*t73.*t122;
t1049 = t47.*t73.*t123;
t1054 = t16.*t47.*t60.*zeta_dot.*(4.0./3.75e+2);
t1055 = t16.*t47.*t61.*zeta_dot.*(7.0./3.75e+2);
t1056 = t16.*t47.*t62.*zeta_dot.*(7.0./3.75e+2);
t1057 = t16.*t47.*t63.*zeta_dot.*(4.0./3.75e+2);
t1058 = t16.*t47.*t64.*zeta_dot.*(7.0./3.75e+2);
t1059 = t16.*t47.*t65.*zeta_dot.*(7.0./3.75e+2);
t1060 = t16.*t47.*t66.*zeta_dot.*(4.0./3.75e+2);
t1061 = t16.*t47.*t67.*zeta_dot.*(7.0./3.75e+2);
t1062 = t16.*t47.*t68.*zeta_dot.*(7.0./3.75e+2);
t1063 = t16.*t47.*t69.*zeta_dot.*(4.0./3.75e+2);
t1064 = t16.*t47.*t70.*zeta_dot.*(7.0./3.75e+2);
t1065 = t16.*t47.*t71.*zeta_dot.*(7.0./3.75e+2);
t1079 = (phi_dot.*t3.*t72.*t76)./3.75e+2;
t1080 = (phi_dot.*t3.*t72.*t77)./3.75e+2;
t1082 = (phi_dot.*t3.*t72.*t79)./3.75e+2;
t1083 = (phi_dot.*t3.*t72.*t80)./3.75e+2;
t1085 = (phi_dot.*t3.*t72.*t82)./3.75e+2;
t1086 = (phi_dot.*t3.*t72.*t83)./3.75e+2;
t1088 = (phi_dot.*t3.*t72.*t85)./3.75e+2;
t1089 = (phi_dot.*t3.*t72.*t86)./3.75e+2;
t1102 = (t16.*t74.*t75.*th11_dot)./3.75e+2;
t1103 = (t16.*t74.*t78.*th21_dot)./3.75e+2;
t1104 = (t16.*t74.*t81.*th31_dot)./3.75e+2;
t1105 = (t16.*t74.*t84.*th41_dot)./3.75e+2;
t1118 = t3.*t31.*t394;
t1119 = t3.*t31.*t397;
t1120 = t3.*t31.*t400;
t1121 = t3.*t31.*t403;
t1138 = t3.*t16.*t18.*t266;
t1139 = t3.*t16.*t18.*t267;
t1140 = t3.*t16.*t18.*t268;
t1141 = t3.*t16.*t18.*t269;
t1142 = t3.*t16.*t18.*t270;
t1143 = t3.*t16.*t18.*t271;
t1144 = t3.*t16.*t18.*t272;
t1145 = t3.*t16.*t18.*t273;
t1154 = t31.*t684;
t1155 = t31.*t686;
t1156 = t31.*t688;
t1157 = t31.*t690;
t1158 = t31.*t692;
t1159 = t31.*t694;
t1160 = t31.*t696;
t1161 = t31.*t698;
t1164 = t31.*t704;
t1165 = t31.*t706;
t1168 = t31.*t712;
t1169 = t31.*t714;
t1175 = t61.*t350;
t1176 = t62.*t350;
t1177 = t64.*t350;
t1178 = t65.*t350;
t1179 = t67.*t350;
t1180 = t68.*t350;
t1181 = t70.*t350;
t1182 = t71.*t350;
t1183 = phi_dot.*t3.*t18.*t19.*t73.*(3.0./2.5e+2);
t1184 = phi_dot.*t3.*t18.*t20.*t73.*(3.0./2.5e+2);
t1185 = phi_dot.*t3.*t18.*t21.*t73.*(3.0./2.5e+2);
t1186 = phi_dot.*t3.*t18.*t22.*t73.*(3.0./2.5e+2);
t1187 = phi_dot.*t3.*t18.*t23.*t73.*(3.0./2.5e+2);
t1188 = phi_dot.*t3.*t18.*t24.*t73.*(3.0./2.5e+2);
t1190 = phi_dot.*t3.*t18.*t26.*t73.*(3.0./2.5e+2);
t1191 = phi_dot.*t3.*t18.*t27.*t73.*(3.0./2.5e+2);
t1193 = phi_dot.*t3.*t18.*t29.*t73.*(3.0./2.5e+2);
t1194 = phi_dot.*t3.*t18.*t30.*t73.*(3.0./2.5e+2);
t1195 = t46.*t406;
t1196 = t46.*t407;
t1197 = t46.*t408;
t1198 = t46.*t409;
t1199 = t46.*t410;
t1200 = t46.*t411;
t1201 = t46.*t412;
t1202 = t46.*t413;
t1203 = t47.*t394;
t1204 = t47.*t395;
t1205 = t47.*t396;
t1206 = t47.*t397;
t1207 = t47.*t398;
t1208 = t47.*t399;
t1209 = t47.*t400;
t1210 = t47.*t401;
t1211 = t47.*t402;
t1212 = t47.*t403;
t1213 = t47.*t404;
t1214 = t47.*t405;
t1215 = t46.*t414;
t1216 = t46.*t415;
t1217 = t46.*t416;
t1218 = t46.*t417;
t1219 = t46.*t418;
t1220 = t46.*t419;
t1221 = t46.*t420;
t1222 = t46.*t421;
t1223 = t46.*t422;
t1224 = t46.*t423;
t1225 = t46.*t424;
t1226 = t46.*t425;
t1227 = t46.*t426;
t1228 = t46.*t427;
t1229 = t46.*t428;
t1230 = t46.*t429;
t1231 = t46.*t430;
t1232 = t46.*t431;
t1233 = t46.*t432;
t1234 = t46.*t433;
t1235 = t4.*t16.*t47.*zeta_dot.*(2.1e+1./1.0e+3);
t1236 = t5.*t16.*t47.*zeta_dot.*(2.1e+1./1.0e+3);
t1237 = t6.*t16.*t47.*zeta_dot.*(2.1e+1./1.0e+3);
t1238 = t7.*t16.*t47.*zeta_dot.*(2.1e+1./1.0e+3);
t1239 = t8.*t16.*t47.*zeta_dot.*(2.1e+1./1.0e+3);
t1240 = t9.*t16.*t47.*zeta_dot.*(2.1e+1./1.0e+3);
t1241 = t10.*t16.*t47.*zeta_dot.*(2.1e+1./1.0e+3);
t1242 = t11.*t16.*t47.*zeta_dot.*(2.1e+1./1.0e+3);
t1243 = t12.*t16.*t47.*zeta_dot.*(2.1e+1./1.0e+3);
t1244 = t13.*t16.*t47.*zeta_dot.*(2.1e+1./1.0e+3);
t1245 = t14.*t16.*t47.*zeta_dot.*(2.1e+1./1.0e+3);
t1246 = t15.*t16.*t47.*zeta_dot.*(2.1e+1./1.0e+3);
t1247 = t5.*t16.*t47.*zeta_dot.*1.35e-2;
t1248 = t6.*t16.*t47.*zeta_dot.*1.35e-2;
t1249 = t8.*t16.*t47.*zeta_dot.*1.35e-2;
t1250 = t9.*t16.*t47.*zeta_dot.*1.35e-2;
t1251 = t11.*t16.*t47.*zeta_dot.*1.35e-2;
t1252 = t12.*t16.*t47.*zeta_dot.*1.35e-2;
t1253 = t14.*t16.*t47.*zeta_dot.*1.35e-2;
t1254 = t15.*t16.*t47.*zeta_dot.*1.35e-2;
t1255 = phi_dot.*t4.*t18.*t72.*(2.1e+1./1.0e+3);
t1256 = phi_dot.*t7.*t18.*t72.*(2.1e+1./1.0e+3);
t1257 = phi_dot.*t10.*t18.*t72.*(2.1e+1./1.0e+3);
t1258 = phi_dot.*t13.*t18.*t72.*(2.1e+1./1.0e+3);
t1259 = phi_dot.*t5.*t18.*t72.*1.05e-2;
t1260 = phi_dot.*t6.*t18.*t72.*1.05e-2;
t1261 = phi_dot.*t8.*t18.*t72.*1.05e-2;
t1262 = phi_dot.*t9.*t18.*t72.*1.05e-2;
t1263 = phi_dot.*t3.*t20.*t72.*1.65e-2;
t1264 = phi_dot.*t3.*t21.*t72.*1.65e-2;
t1265 = phi_dot.*t11.*t18.*t72.*1.05e-2;
t1266 = phi_dot.*t12.*t18.*t72.*1.05e-2;
t1267 = phi_dot.*t3.*t23.*t72.*1.65e-2;
t1268 = phi_dot.*t3.*t24.*t72.*1.65e-2;
t1269 = phi_dot.*t14.*t18.*t72.*1.05e-2;
t1270 = phi_dot.*t15.*t18.*t72.*1.05e-2;
t1271 = phi_dot.*t3.*t26.*t72.*2.55e-2;
t1272 = phi_dot.*t3.*t27.*t72.*2.55e-2;
t1273 = phi_dot.*t3.*t29.*t72.*2.55e-2;
t1274 = phi_dot.*t3.*t30.*t72.*2.55e-2;
t1275 = phi_dot.*t16.*t19.*t74.*(2.1e+1./1.0e+3);
t1276 = phi_dot.*t16.*t20.*t74.*(2.1e+1./1.0e+3);
t1277 = phi_dot.*t16.*t21.*t74.*(2.1e+1./1.0e+3);
t1278 = phi_dot.*t16.*t22.*t74.*(2.1e+1./1.0e+3);
t1279 = phi_dot.*t16.*t23.*t74.*(2.1e+1./1.0e+3);
t1280 = phi_dot.*t16.*t24.*t74.*(2.1e+1./1.0e+3);
t1281 = phi_dot.*t16.*t25.*t74.*(2.1e+1./1.0e+3);
t1282 = phi_dot.*t16.*t26.*t74.*(2.1e+1./1.0e+3);
t1283 = phi_dot.*t16.*t27.*t74.*(2.1e+1./1.0e+3);
t1284 = phi_dot.*t16.*t28.*t74.*(2.1e+1./1.0e+3);
t1285 = phi_dot.*t16.*t29.*t74.*(2.1e+1./1.0e+3);
t1286 = phi_dot.*t16.*t30.*t74.*(2.1e+1./1.0e+3);
t1287 = psi_dot.*t16.*t19.*t74.*(2.1e+1./1.0e+3);
t1288 = psi_dot.*t16.*t20.*t74.*(2.1e+1./1.0e+3);
t1289 = psi_dot.*t16.*t21.*t74.*(2.1e+1./1.0e+3);
t1290 = psi_dot.*t16.*t22.*t74.*(2.1e+1./1.0e+3);
t1291 = psi_dot.*t16.*t23.*t74.*(2.1e+1./1.0e+3);
t1292 = psi_dot.*t16.*t24.*t74.*(2.1e+1./1.0e+3);
t1293 = psi_dot.*t16.*t25.*t74.*(2.1e+1./1.0e+3);
t1294 = psi_dot.*t16.*t26.*t74.*(2.1e+1./1.0e+3);
t1295 = psi_dot.*t16.*t27.*t74.*(2.1e+1./1.0e+3);
t1296 = psi_dot.*t16.*t28.*t74.*(2.1e+1./1.0e+3);
t1297 = psi_dot.*t16.*t29.*t74.*(2.1e+1./1.0e+3);
t1298 = psi_dot.*t16.*t30.*t74.*(2.1e+1./1.0e+3);
t1299 = t16.*t20.*t74.*th12_dot.*3.375e-3;
t1300 = t16.*t21.*t74.*th13_dot.*3.375e-3;
t1301 = t16.*t23.*t74.*th22_dot.*3.375e-3;
t1302 = t16.*t24.*t74.*th23_dot.*3.375e-3;
t1303 = t16.*t26.*t74.*th32_dot.*3.375e-3;
t1304 = t16.*t27.*t74.*th33_dot.*3.375e-3;
t1305 = t16.*t29.*t74.*th42_dot.*3.375e-3;
t1306 = t16.*t30.*t74.*th43_dot.*3.375e-3;
t1307 = t16.*t47.*zeta_dot.*5.21125e-1;
t1316 = t31.*t917;
t1317 = t31.*t918;
t1318 = t31.*t919;
t1319 = t31.*t920;
t1320 = t31.*t921;
t1321 = t31.*t922;
t1322 = t31.*t923;
t1323 = t31.*t924;
t1324 = t31.*t925;
t1325 = t31.*t926;
t1326 = t31.*t927;
t1327 = t31.*t928;
t1328 = t31.*t929;
t1329 = t31.*t930;
t1330 = t31.*t931;
t1331 = t31.*t932;
t1340 = phi_dot.*t16.*t46.*t49.*4.666666666666667e-3;
t1341 = phi_dot.*t16.*t46.*t50.*4.666666666666667e-3;
t1342 = phi_dot.*t16.*t46.*t52.*4.666666666666667e-3;
t1343 = phi_dot.*t16.*t46.*t53.*4.666666666666667e-3;
t1344 = phi_dot.*t16.*t46.*t55.*4.666666666666667e-3;
t1345 = phi_dot.*t16.*t46.*t56.*4.666666666666667e-3;
t1346 = phi_dot.*t16.*t46.*t58.*4.666666666666667e-3;
t1347 = phi_dot.*t16.*t46.*t59.*4.666666666666667e-3;
t1348 = psi_dot.*t16.*t46.*t48.*(-1.0./3.75e+2);
t1349 = psi_dot.*t16.*t46.*t51.*(-1.0./3.75e+2);
t1350 = psi_dot.*t16.*t46.*t54.*(-1.0./3.75e+2);
t1351 = psi_dot.*t16.*t46.*t57.*(-1.0./3.75e+2);
t1352 = psi_dot.*t16.*t46.*t49.*4.666666666666667e-3;
t1353 = psi_dot.*t16.*t46.*t50.*4.666666666666667e-3;
t1354 = psi_dot.*t16.*t46.*t52.*4.666666666666667e-3;
t1355 = psi_dot.*t16.*t46.*t53.*4.666666666666667e-3;
t1356 = psi_dot.*t16.*t46.*t55.*4.666666666666667e-3;
t1357 = psi_dot.*t16.*t46.*t56.*4.666666666666667e-3;
t1358 = psi_dot.*t16.*t46.*t58.*4.666666666666667e-3;
t1359 = psi_dot.*t16.*t46.*t59.*4.666666666666667e-3;
t1360 = phi_dot.*t19.*t47.*t73.*(2.1e+1./5.0e+2);
t1361 = phi_dot.*t20.*t47.*t73.*(2.1e+1./5.0e+2);
t1362 = phi_dot.*t21.*t47.*t73.*(2.1e+1./5.0e+2);
t1363 = phi_dot.*t22.*t47.*t73.*(2.1e+1./5.0e+2);
t1364 = phi_dot.*t23.*t47.*t73.*(2.1e+1./5.0e+2);
t1365 = phi_dot.*t24.*t47.*t73.*(2.1e+1./5.0e+2);
t1366 = phi_dot.*t25.*t47.*t73.*(2.1e+1./5.0e+2);
t1367 = phi_dot.*t26.*t47.*t73.*(2.1e+1./5.0e+2);
t1368 = phi_dot.*t27.*t47.*t73.*(2.1e+1./5.0e+2);
t1369 = phi_dot.*t28.*t47.*t73.*(2.1e+1./5.0e+2);
t1370 = phi_dot.*t29.*t47.*t73.*(2.1e+1./5.0e+2);
t1371 = phi_dot.*t30.*t47.*t73.*(2.1e+1./5.0e+2);
t1384 = t16.*t74.*t76.*th12_dot.*4.666666666666667e-3;
t1385 = t16.*t74.*t77.*th13_dot.*4.666666666666667e-3;
t1386 = t16.*t74.*t79.*th22_dot.*4.666666666666667e-3;
t1387 = t16.*t74.*t80.*th23_dot.*4.666666666666667e-3;
t1388 = t16.*t74.*t82.*th32_dot.*4.666666666666667e-3;
t1389 = t16.*t74.*t83.*th33_dot.*4.666666666666667e-3;
t1390 = t16.*t74.*t85.*th42_dot.*4.666666666666667e-3;
t1391 = t16.*t74.*t86.*th43_dot.*4.666666666666667e-3;
t1392 = phi_dot.*t16.*t47.*t92.*(2.0./3.75e+2);
t1393 = phi_dot.*t16.*t61.*t92.*(2.0./3.75e+2);
t1394 = phi_dot.*t16.*t62.*t92.*(2.0./3.75e+2);
t1395 = phi_dot.*t16.*t64.*t92.*(2.0./3.75e+2);
t1396 = phi_dot.*t16.*t65.*t92.*(2.0./3.75e+2);
t1397 = phi_dot.*t16.*t67.*t92.*(2.0./3.75e+2);
t1398 = phi_dot.*t16.*t68.*t92.*(2.0./3.75e+2);
t1399 = phi_dot.*t16.*t70.*t92.*(2.0./3.75e+2);
t1400 = phi_dot.*t16.*t71.*t92.*(2.0./3.75e+2);
t1401 = t47.*t566;
t1402 = t61.*t566;
t1403 = t62.*t566;
t1404 = t64.*t566;
t1405 = t65.*t566;
t1406 = t67.*t566;
t1407 = t68.*t566;
t1408 = t70.*t566;
t1409 = t71.*t566;
t1410 = phi_dot.*t3.*t16.*t31.*t60.*(8.0./3.75e+2);
t1411 = phi_dot.*t3.*t16.*t31.*t63.*(8.0./3.75e+2);
t1412 = phi_dot.*t3.*t16.*t31.*t66.*(8.0./3.75e+2);
t1413 = phi_dot.*t3.*t16.*t31.*t69.*(8.0./3.75e+2);
t1414 = psi_dot.*t5.*t16.*t46.*(-6.75e-3);
t1415 = psi_dot.*t6.*t16.*t46.*(-6.75e-3);
t1416 = psi_dot.*t8.*t16.*t46.*(-6.75e-3);
t1417 = psi_dot.*t9.*t16.*t46.*(-6.75e-3);
t1418 = psi_dot.*t11.*t16.*t46.*(-6.75e-3);
t1419 = psi_dot.*t12.*t16.*t46.*(-6.75e-3);
t1420 = psi_dot.*t14.*t16.*t46.*(-6.75e-3);
t1421 = psi_dot.*t15.*t16.*t46.*(-6.75e-3);
t1422 = t7.*t16.*t46.*th21_dot.*(-1.05e-2);
t1423 = t8.*t16.*t46.*th22_dot.*(-1.05e-2);
t1424 = t9.*t16.*t46.*th23_dot.*(-1.05e-2);
t1425 = t10.*t16.*t46.*th31_dot.*(-1.05e-2);
t1426 = t11.*t16.*t46.*th32_dot.*(-1.05e-2);
t1427 = t12.*t16.*t46.*th33_dot.*(-1.05e-2);
t1458 = phi_dot.*t16.*t46.*3.085625e-1;
t1459 = psi_dot.*t16.*t46.*3.085625e-1;
t1501 = phi_dot.*t5.*t20.*t47.*t73.*(7.0./3.75e+2);
t1502 = phi_dot.*t6.*t21.*t47.*t73.*(7.0./3.75e+2);
t1504 = phi_dot.*t8.*t23.*t47.*t73.*(7.0./3.75e+2);
t1505 = phi_dot.*t9.*t24.*t47.*t73.*(7.0./3.75e+2);
t1507 = phi_dot.*t11.*t26.*t47.*t73.*(7.0./3.75e+2);
t1508 = phi_dot.*t12.*t27.*t47.*t73.*(7.0./3.75e+2);
t1510 = phi_dot.*t14.*t29.*t47.*t73.*(7.0./3.75e+2);
t1511 = phi_dot.*t15.*t30.*t47.*t73.*(7.0./3.75e+2);
t1512 = -t1333;
t1513 = -t1334;
t1514 = -t1336;
t1515 = -t1339;
t1524 = phi_dot.*t5.*t46.*t87.*3.375e-3;
t1525 = phi_dot.*t6.*t46.*t87.*3.375e-3;
t1526 = phi_dot.*t8.*t46.*t87.*3.375e-3;
t1527 = phi_dot.*t9.*t46.*t87.*3.375e-3;
t1528 = phi_dot.*t11.*t46.*t87.*3.375e-3;
t1529 = phi_dot.*t12.*t46.*t87.*3.375e-3;
t1530 = phi_dot.*t14.*t46.*t87.*3.375e-3;
t1531 = phi_dot.*t15.*t46.*t87.*3.375e-3;
t1532 = t47.*t73.*t266;
t1533 = t47.*t73.*t267;
t1534 = t47.*t73.*t268;
t1535 = t47.*t73.*t269;
t1536 = t47.*t73.*t270;
t1537 = t47.*t73.*t271;
t1538 = t47.*t73.*t272;
t1539 = t47.*t73.*t273;
t1541 = phi_dot.*t5.*t73.*t92.*(3.0./1.0e+3);
t1542 = phi_dot.*t6.*t73.*t92.*(3.0./1.0e+3);
t1543 = phi_dot.*t8.*t73.*t92.*(3.0./1.0e+3);
C = ft_3({phi_dot,psi_dot,t10,t100,t1000,t1001,t101,t1010,t1011,t1012,t1013,t1014,t1015,t1016,t1017,t1018,t1019,t102,t1020,t1021,t1022,t1023,t1024,t1025,t1026,t1027,t1028,t1029,t103,t1030,t1031,t1032,t1033,t1038,t1039,t104,t1040,t1041,t1042,t1043,t1044,t1045,t1046,t1047,t1048,t1049,t105,t1054,t1055,t1056,t1057,t1058,t1059,t1060,t1061,t1062,t1063,t1064,t1065,t1066,t1067,t1068,t1069,t1070,t1071,t1072,t1073,t1074,t1075,t1076,t1077,t1079,t1080,t1082,t1083,t1085,t1086,t1088,t1089,t1090,t1091,t1092,t1093,t1094,t1095,t1096,t1097,t1098,t1099,t11,t1100,t1101,t1102,t1103,t1104,t1105,t1106,t1107,t1108,t1109,t1110,t1111,t1112,t1113,t1114,t1115,t1116,t1117,t1118,t1119,t112,t1120,t1121,t1122,t1123,t1124,t1125,t1126,t1127,t1128,t1129,t113,t1130,t1131,t1132,t1133,t1134,t1135,t1136,t1137,t1138,t1139,t114,t1140,t1141,t1142,t1143,t1144,t1145,t1146,t1147,t1148,t1149,t115,t1150,t1151,t1152,t1153,t1154,t1155,t1156,t1157,t1158,t1159,t116,t1160,t1161,t1162,t1163,t1164,t1165,t1166,t1167,t1168,t1169,t117,t1170,t1171,t1172,t1173,t1175,t1176,t1177,t1178,t1179,t118,t1180,t1181,t1182,t1183,t1184,t1185,t1186,t1187,t1188,t119,t1190,t1191,t1193,t1194,t1195,t1196,t1197,t1198,t1199,t12,t120,t1200,t1201,t1202,t1203,t1204,t1205,t1206,t1207,t1208,t1209,t121,t1210,t1211,t1212,t1213,t1214,t122,t1223,t1224,t1225,t123,t1232,t1233,t1234,t1235,t1236,t1237,t1238,t1239,t124,t1240,t1241,t1242,t1243,t1244,t1245,t1246,t1247,t1248,t1249,t125,t1250,t1251,t1252,t1253,t1254,t1255,t1256,t1257,t1258,t1259,t126,t1260,t1261,t1262,t1263,t1264,t1265,t1266,t1267,t1268,t1269,t127,t1270,t1271,t1272,t1273,t1274,t1275,t1276,t1277,t1278,t1279,t128,t1280,t1281,t1282,t1283,t1284,t1285,t1286,t1287,t1288,t1289,t129,t1290,t1291,t1292,t1293,t1294,t1295,t1296,t1297,t1298,t1299,t13,t130,t1300,t1301,t1302,t1303,t1304,t1305,t1306,t1307,t1308,t1309,t131,t1310,t1311,t1312,t1313,t1314,t1315,t1316,t1317,t1318,t1319,t132,t1320,t1321,t1322,t1323,t1324,t1325,t1326,t1327,t1328,t1329,t133,t1330,t1331,t1332,t1335,t1337,t1338,t134,t1340,t1341,t1342,t1343,t1344,t1345,t1346,t1347,t1348,t1349,t135,t1350,t1351,t1352,t1353,t1354,t1355,t1356,t1357,t1358,t1359,t136,t1360,t1361,t1362,t1363,t1364,t1365,t1366,t1367,t1368,t1369,t1370,t1371,t138,t1384,t1385,t1386,t1387,t1388,t1389,t139,t1390,t1391,t1392,t1393,t1394,t1395,t1396,t1397,t1398,t1399,t14,t140,t1400,t1401,t1402,t1403,t1404,t1405,t1406,t1407,t1408,t1409,t141,t1410,t1411,t1412,t1413,t1414,t1415,t1416,t1417,t1418,t1419,t142,t1420,t1421,t1422,t1423,t1424,t1425,t1426,t1427,t1428,t1429,t143,t1430,t1431,t1432,t1433,t1434,t1435,t1436,t1437,t1438,t1439,t144,t1440,t1441,t1442,t1443,t1444,t1445,t1446,t1447,t145,t1458,t1459,t146,t1460,t1461,t1462,t1463,t1464,t1465,t1466,t1467,t1468,t1469,t147,t1470,t1471,t1472,t1473,t1474,t1475,t1476,t1477,t1478,t1479,t148,t1480,t1481,t1482,t1483,t1484,t1485,t1486,t1487,t1488,t1489,t149,t1490,t1491,t1492,t1493,t1494,t1495,t1496,t1497,t1498,t1499,t15,t150,t1501,t1502,t1504,t1505,t1507,t1508,t151,t1510,t1511,t1512,t1513,t1514,t1515,t152,t1524,t1525,t1526,t1527,t1528,t1529,t153,t1530,t1531,t1532,t1533,t1534,t1535,t1536,t1537,t1538,t1539,t154,t1541,t1542,t1543,t155,t156,t157,t158,t159,t16,t160,t161,t162,t163,t164,t165,t166,t167,t168,t169,t17,t170,t171,t1711,t1712,t1713,t1714,t172,t1728,t173,t1730,t1732,t1734,t1736,t1738,t174,t1740,t1742,t1743,t1744,t1745,t1746,t1747,t1748,t1749,t175,t1750,t176,t177,t1775,t1776,t1777,t1778,t178,t1783,t1784,t1785,t1786,t1787,t1788,t1789,t179,t1790,t1791,t1792,t1793,t1794,t1795,t1796,t1797,t1798,t1799,t18,t180,t1800,t1801,t1802,t1803,t1804,t1805,t1806,t181,t182,t183,t184,t185,t1865,t1866,t1867,t1868,t187,t188,t189,t19,t190,t191,t192,t193,t194,t195,t196,t197,t198,t199,t1994,t1995,t1996,t1997,t1998,t1999,t2,t20,t200,t2000,t2001,t201,t202,t203,t2034,t2035,t2036,t2037,t2038,t2039,t204,t2040,t2041,t205,t206,t207,t208,t209,t21,t210,t211,t212,t213,t214,t215,t216,t217,t218,t219,t22,t220,t221,t222,t223,t224,t225,t226,t227,t228,t229,t23,t230,t231,t232,t233,t234,t235,t24,t248,t249,t25,t250,t251,t252,t253,t254,t255,t256,t257,t258,t259,t26,t260,t261,t262,t263,t264,t266,t267,t268,t269,t27,t270,t271,t272,t273,t274,t275,t276,t277,t278,t279,t28,t280,t281,t282,t283,t284,t285,t286,t287,t288,t289,t29,t290,t291,t292,t293,t294,t295,t296,t297,t298,t299,t3,t30,t300,t301,t302,t303,t304,t305,t306,t307,t308,t309,t31,t310,t311,t312,t313,t314,t315,t316,t317,t318,t319,t320,t321,t322,t323,t324,t329,t330,t331,t332,t333,t334,t335,t336,t337,t338,t339,t340,t342,t344,t346,t348,t349,t350,t351,t352,t353,t354,t355,t356,t357,t358,t361,t362,t363,t364,t365,t366,t367,t368,t369,t370,t371,t372,t373,t374,t375,t376,t377,t378,t379,t380,t381,t394,t395,t396,t397,t398,t399,t4,t400,t401,t402,t403,t404,t405,t406,t407,t408,t409,t410,t411,t412,t413,t414,t415,t416,t417,t418,t419,t420,t421,t422,t423,t424,t425,t426,t427,t428,t429,t430,t431,t432,t433,t434,t435,t436,t437,t438,t439,t440,t441,t442,t443,t444,t445,t446,t447,t448,t449,t450,t451,t452,t453,t454,t455,t456,t457,t458,t459,t46,t460,t461,t462,t463,t464,t465,t466,t467,t468,t469,t47,t470,t471,t472,t473,t474,t475,t476,t477,t478,t479,t48,t480,t481,t482,t483,t484,t485,t486,t487,t488,t489,t49,t490,t491,t492,t493,t494,t495,t496,t497,t498,t499,t5,t50,t500,t501,t503,t504,t506,t507,t509,t51,t510,t512,t513,t514,t515,t516,t517,t518,t519,t52,t520,t521,t522,t523,t524,t525,t526,t527,t528,t529,t53,t530,t531,t532,t533,t534,t535,t536,t537,t538,t539,t54,t540,t541,t542,t543,t544,t545,t546,t547,t548,t549,t55,t550,t551,t552,t553,t554,t555,t556,t557,t558,t559,t56,t560,t561,t562,t563,t564,t565,t566,t567,t568,t569,t57,t570,t571,t572,t573,t574,t575,t576,t577,t578,t579,t58,t580,t581,t582,t583,t584,t585,t586,t587,t588,t589,t59,t590,t591,t592,t593,t594,t595,t596,t597,t598,t599,t6,t60,t600,t601,t602,t603,t604,t605,t606,t607,t608,t609,t61,t610,t611,t612,t613,t614,t615,t616,t617,t618,t619,t62,t620,t621,t622,t623,t624,t625,t626,t627,t628,t629,t63,t630,t631,t632,t633,t634,t635,t636,t637,t638,t639,t64,t640,t641,t642,t643,t644,t645,t646,t647,t648,t649,t65,t650,t651,t652,t653,t654,t655,t656,t657,t66,t666,t667,t668,t669,t67,t670,t671,t672,t673,t674,t675,t676,t677,t678,t679,t68,t680,t681,t682,t683,t684,t685,t686,t687,t688,t689,t69,t690,t691,t692,t693,t694,t695,t696,t697,t698,t699,t7,t70,t700,t701,t702,t703,t704,t705,t706,t707,t708,t709,t71,t710,t711,t712,t713,t714,t715,t716,t717,t718,t719,t72,t720,t721,t722,t725,t726,t727,t728,t729,t73,t730,t731,t732,t733,t734,t735,t736,t737,t738,t739,t74,t740,t741,t742,t743,t744,t745,t746,t747,t748,t749,t75,t750,t751,t752,t753,t754,t755,t756,t757,t758,t759,t76,t760,t761,t762,t763,t764,t765,t766,t767,t768,t769,t77,t770,t771,t772,t773,t774,t775,t776,t777,t778,t779,t78,t780,t781,t782,t783,t784,t785,t786,t787,t788,t789,t79,t790,t791,t792,t793,t794,t795,t796,t797,t798,t799,t8,t80,t800,t801,t802,t803,t804,t805,t806,t807,t808,t809,t81,t810,t811,t812,t813,t814,t815,t816,t817,t818,t819,t82,t820,t821,t822,t823,t824,t825,t826,t827,t828,t83,t830,t831,t833,t834,t836,t837,t839,t84,t840,t841,t842,t843,t844,t845,t846,t847,t848,t849,t85,t850,t851,t852,t86,t866,t869,t87,t872,t875,t877,t878,t879,t88,t880,t881,t882,t883,t884,t885,t886,t887,t888,t889,t89,t890,t891,t892,t893,t894,t895,t896,t897,t898,t899,t9,t90,t900,t901,t902,t903,t904,t905,t906,t907,t908,t909,t91,t910,t911,t912,t913,t914,t915,t916,t917,t918,t919,t92,t920,t921,t922,t923,t924,t925,t926,t927,t928,t929,t93,t930,t931,t932,t933,t934,t935,t936,t937,t938,t939,t94,t940,t941,t942,t943,t944,t945,t946,t947,t948,t949,t95,t950,t951,t952,t953,t954,t955,t956,t957,t958,t96,t960,t961,t962,t963,t964,t965,t966,t967,t968,t969,t97,t970,t971,t972,t973,t974,t975,t976,t977,t978,t979,t98,t980,t981,t982,t983,t984,t985,t986,t987,t989,t99,t994,t995,t996,t997,t998,t999,th11_dot,th12_dot,th13_dot,th21_dot,th22_dot,th23_dot,th31_dot,th32_dot,th33_dot,th41_dot,th42_dot,th43_dot,zeta_dot});
end
function C = ft_3(ct)
phi_dot = ct{1};
psi_dot = ct{2};
t10 = ct{3};
t100 = ct{4};
t1000 = ct{5};
t1001 = ct{6};
t101 = ct{7};
t1010 = ct{8};
t1011 = ct{9};
t1012 = ct{10};
t1013 = ct{11};
t1014 = ct{12};
t1015 = ct{13};
t1016 = ct{14};
t1017 = ct{15};
t1018 = ct{16};
t1019 = ct{17};
t102 = ct{18};
t1020 = ct{19};
t1021 = ct{20};
t1022 = ct{21};
t1023 = ct{22};
t1024 = ct{23};
t1025 = ct{24};
t1026 = ct{25};
t1027 = ct{26};
t1028 = ct{27};
t1029 = ct{28};
t103 = ct{29};
t1030 = ct{30};
t1031 = ct{31};
t1032 = ct{32};
t1033 = ct{33};
t1038 = ct{34};
t1039 = ct{35};
t104 = ct{36};
t1040 = ct{37};
t1041 = ct{38};
t1042 = ct{39};
t1043 = ct{40};
t1044 = ct{41};
t1045 = ct{42};
t1046 = ct{43};
t1047 = ct{44};
t1048 = ct{45};
t1049 = ct{46};
t105 = ct{47};
t1054 = ct{48};
t1055 = ct{49};
t1056 = ct{50};
t1057 = ct{51};
t1058 = ct{52};
t1059 = ct{53};
t1060 = ct{54};
t1061 = ct{55};
t1062 = ct{56};
t1063 = ct{57};
t1064 = ct{58};
t1065 = ct{59};
t1066 = ct{60};
t1067 = ct{61};
t1068 = ct{62};
t1069 = ct{63};
t1070 = ct{64};
t1071 = ct{65};
t1072 = ct{66};
t1073 = ct{67};
t1074 = ct{68};
t1075 = ct{69};
t1076 = ct{70};
t1077 = ct{71};
t1079 = ct{72};
t1080 = ct{73};
t1082 = ct{74};
t1083 = ct{75};
t1085 = ct{76};
t1086 = ct{77};
t1088 = ct{78};
t1089 = ct{79};
t1090 = ct{80};
t1091 = ct{81};
t1092 = ct{82};
t1093 = ct{83};
t1094 = ct{84};
t1095 = ct{85};
t1096 = ct{86};
t1097 = ct{87};
t1098 = ct{88};
t1099 = ct{89};
t11 = ct{90};
t1100 = ct{91};
t1101 = ct{92};
t1102 = ct{93};
t1103 = ct{94};
t1104 = ct{95};
t1105 = ct{96};
t1106 = ct{97};
t1107 = ct{98};
t1108 = ct{99};
t1109 = ct{100};
t1110 = ct{101};
t1111 = ct{102};
t1112 = ct{103};
t1113 = ct{104};
t1114 = ct{105};
t1115 = ct{106};
t1116 = ct{107};
t1117 = ct{108};
t1118 = ct{109};
t1119 = ct{110};
t112 = ct{111};
t1120 = ct{112};
t1121 = ct{113};
t1122 = ct{114};
t1123 = ct{115};
t1124 = ct{116};
t1125 = ct{117};
t1126 = ct{118};
t1127 = ct{119};
t1128 = ct{120};
t1129 = ct{121};
t113 = ct{122};
t1130 = ct{123};
t1131 = ct{124};
t1132 = ct{125};
t1133 = ct{126};
t1134 = ct{127};
t1135 = ct{128};
t1136 = ct{129};
t1137 = ct{130};
t1138 = ct{131};
t1139 = ct{132};
t114 = ct{133};
t1140 = ct{134};
t1141 = ct{135};
t1142 = ct{136};
t1143 = ct{137};
t1144 = ct{138};
t1145 = ct{139};
t1146 = ct{140};
t1147 = ct{141};
t1148 = ct{142};
t1149 = ct{143};
t115 = ct{144};
t1150 = ct{145};
t1151 = ct{146};
t1152 = ct{147};
t1153 = ct{148};
t1154 = ct{149};
t1155 = ct{150};
t1156 = ct{151};
t1157 = ct{152};
t1158 = ct{153};
t1159 = ct{154};
t116 = ct{155};
t1160 = ct{156};
t1161 = ct{157};
t1162 = ct{158};
t1163 = ct{159};
t1164 = ct{160};
t1165 = ct{161};
t1166 = ct{162};
t1167 = ct{163};
t1168 = ct{164};
t1169 = ct{165};
t117 = ct{166};
t1170 = ct{167};
t1171 = ct{168};
t1172 = ct{169};
t1173 = ct{170};
t1175 = ct{171};
t1176 = ct{172};
t1177 = ct{173};
t1178 = ct{174};
t1179 = ct{175};
t118 = ct{176};
t1180 = ct{177};
t1181 = ct{178};
t1182 = ct{179};
t1183 = ct{180};
t1184 = ct{181};
t1185 = ct{182};
t1186 = ct{183};
t1187 = ct{184};
t1188 = ct{185};
t119 = ct{186};
t1190 = ct{187};
t1191 = ct{188};
t1193 = ct{189};
t1194 = ct{190};
t1195 = ct{191};
t1196 = ct{192};
t1197 = ct{193};
t1198 = ct{194};
t1199 = ct{195};
t12 = ct{196};
t120 = ct{197};
t1200 = ct{198};
t1201 = ct{199};
t1202 = ct{200};
t1203 = ct{201};
t1204 = ct{202};
t1205 = ct{203};
t1206 = ct{204};
t1207 = ct{205};
t1208 = ct{206};
t1209 = ct{207};
t121 = ct{208};
t1210 = ct{209};
t1211 = ct{210};
t1212 = ct{211};
t1213 = ct{212};
t1214 = ct{213};
t122 = ct{214};
t1223 = ct{215};
t1224 = ct{216};
t1225 = ct{217};
t123 = ct{218};
t1232 = ct{219};
t1233 = ct{220};
t1234 = ct{221};
t1235 = ct{222};
t1236 = ct{223};
t1237 = ct{224};
t1238 = ct{225};
t1239 = ct{226};
t124 = ct{227};
t1240 = ct{228};
t1241 = ct{229};
t1242 = ct{230};
t1243 = ct{231};
t1244 = ct{232};
t1245 = ct{233};
t1246 = ct{234};
t1247 = ct{235};
t1248 = ct{236};
t1249 = ct{237};
t125 = ct{238};
t1250 = ct{239};
t1251 = ct{240};
t1252 = ct{241};
t1253 = ct{242};
t1254 = ct{243};
t1255 = ct{244};
t1256 = ct{245};
t1257 = ct{246};
t1258 = ct{247};
t1259 = ct{248};
t126 = ct{249};
t1260 = ct{250};
t1261 = ct{251};
t1262 = ct{252};
t1263 = ct{253};
t1264 = ct{254};
t1265 = ct{255};
t1266 = ct{256};
t1267 = ct{257};
t1268 = ct{258};
t1269 = ct{259};
t127 = ct{260};
t1270 = ct{261};
t1271 = ct{262};
t1272 = ct{263};
t1273 = ct{264};
t1274 = ct{265};
t1275 = ct{266};
t1276 = ct{267};
t1277 = ct{268};
t1278 = ct{269};
t1279 = ct{270};
t128 = ct{271};
t1280 = ct{272};
t1281 = ct{273};
t1282 = ct{274};
t1283 = ct{275};
t1284 = ct{276};
t1285 = ct{277};
t1286 = ct{278};
t1287 = ct{279};
t1288 = ct{280};
t1289 = ct{281};
t129 = ct{282};
t1290 = ct{283};
t1291 = ct{284};
t1292 = ct{285};
t1293 = ct{286};
t1294 = ct{287};
t1295 = ct{288};
t1296 = ct{289};
t1297 = ct{290};
t1298 = ct{291};
t1299 = ct{292};
t13 = ct{293};
t130 = ct{294};
t1300 = ct{295};
t1301 = ct{296};
t1302 = ct{297};
t1303 = ct{298};
t1304 = ct{299};
t1305 = ct{300};
t1306 = ct{301};
t1307 = ct{302};
t1308 = ct{303};
t1309 = ct{304};
t131 = ct{305};
t1310 = ct{306};
t1311 = ct{307};
t1312 = ct{308};
t1313 = ct{309};
t1314 = ct{310};
t1315 = ct{311};
t1316 = ct{312};
t1317 = ct{313};
t1318 = ct{314};
t1319 = ct{315};
t132 = ct{316};
t1320 = ct{317};
t1321 = ct{318};
t1322 = ct{319};
t1323 = ct{320};
t1324 = ct{321};
t1325 = ct{322};
t1326 = ct{323};
t1327 = ct{324};
t1328 = ct{325};
t1329 = ct{326};
t133 = ct{327};
t1330 = ct{328};
t1331 = ct{329};
t1332 = ct{330};
t1335 = ct{331};
t1337 = ct{332};
t1338 = ct{333};
t134 = ct{334};
t1340 = ct{335};
t1341 = ct{336};
t1342 = ct{337};
t1343 = ct{338};
t1344 = ct{339};
t1345 = ct{340};
t1346 = ct{341};
t1347 = ct{342};
t1348 = ct{343};
t1349 = ct{344};
t135 = ct{345};
t1350 = ct{346};
t1351 = ct{347};
t1352 = ct{348};
t1353 = ct{349};
t1354 = ct{350};
t1355 = ct{351};
t1356 = ct{352};
t1357 = ct{353};
t1358 = ct{354};
t1359 = ct{355};
t136 = ct{356};
t1360 = ct{357};
t1361 = ct{358};
t1362 = ct{359};
t1363 = ct{360};
t1364 = ct{361};
t1365 = ct{362};
t1366 = ct{363};
t1367 = ct{364};
t1368 = ct{365};
t1369 = ct{366};
t1370 = ct{367};
t1371 = ct{368};
t138 = ct{369};
t1384 = ct{370};
t1385 = ct{371};
t1386 = ct{372};
t1387 = ct{373};
t1388 = ct{374};
t1389 = ct{375};
t139 = ct{376};
t1390 = ct{377};
t1391 = ct{378};
t1392 = ct{379};
t1393 = ct{380};
t1394 = ct{381};
t1395 = ct{382};
t1396 = ct{383};
t1397 = ct{384};
t1398 = ct{385};
t1399 = ct{386};
t14 = ct{387};
t140 = ct{388};
t1400 = ct{389};
t1401 = ct{390};
t1402 = ct{391};
t1403 = ct{392};
t1404 = ct{393};
t1405 = ct{394};
t1406 = ct{395};
t1407 = ct{396};
t1408 = ct{397};
t1409 = ct{398};
t141 = ct{399};
t1410 = ct{400};
t1411 = ct{401};
t1412 = ct{402};
t1413 = ct{403};
t1414 = ct{404};
t1415 = ct{405};
t1416 = ct{406};
t1417 = ct{407};
t1418 = ct{408};
t1419 = ct{409};
t142 = ct{410};
t1420 = ct{411};
t1421 = ct{412};
t1422 = ct{413};
t1423 = ct{414};
t1424 = ct{415};
t1425 = ct{416};
t1426 = ct{417};
t1427 = ct{418};
t1428 = ct{419};
t1429 = ct{420};
t143 = ct{421};
t1430 = ct{422};
t1431 = ct{423};
t1432 = ct{424};
t1433 = ct{425};
t1434 = ct{426};
t1435 = ct{427};
t1436 = ct{428};
t1437 = ct{429};
t1438 = ct{430};
t1439 = ct{431};
t144 = ct{432};
t1440 = ct{433};
t1441 = ct{434};
t1442 = ct{435};
t1443 = ct{436};
t1444 = ct{437};
t1445 = ct{438};
t1446 = ct{439};
t1447 = ct{440};
t145 = ct{441};
t1458 = ct{442};
t1459 = ct{443};
t146 = ct{444};
t1460 = ct{445};
t1461 = ct{446};
t1462 = ct{447};
t1463 = ct{448};
t1464 = ct{449};
t1465 = ct{450};
t1466 = ct{451};
t1467 = ct{452};
t1468 = ct{453};
t1469 = ct{454};
t147 = ct{455};
t1470 = ct{456};
t1471 = ct{457};
t1472 = ct{458};
t1473 = ct{459};
t1474 = ct{460};
t1475 = ct{461};
t1476 = ct{462};
t1477 = ct{463};
t1478 = ct{464};
t1479 = ct{465};
t148 = ct{466};
t1480 = ct{467};
t1481 = ct{468};
t1482 = ct{469};
t1483 = ct{470};
t1484 = ct{471};
t1485 = ct{472};
t1486 = ct{473};
t1487 = ct{474};
t1488 = ct{475};
t1489 = ct{476};
t149 = ct{477};
t1490 = ct{478};
t1491 = ct{479};
t1492 = ct{480};
t1493 = ct{481};
t1494 = ct{482};
t1495 = ct{483};
t1496 = ct{484};
t1497 = ct{485};
t1498 = ct{486};
t1499 = ct{487};
t15 = ct{488};
t150 = ct{489};
t1501 = ct{490};
t1502 = ct{491};
t1504 = ct{492};
t1505 = ct{493};
t1507 = ct{494};
t1508 = ct{495};
t151 = ct{496};
t1510 = ct{497};
t1511 = ct{498};
t1512 = ct{499};
t1513 = ct{500};
t1514 = ct{501};
t1515 = ct{502};
t152 = ct{503};
t1524 = ct{504};
t1525 = ct{505};
t1526 = ct{506};
t1527 = ct{507};
t1528 = ct{508};
t1529 = ct{509};
t153 = ct{510};
t1530 = ct{511};
t1531 = ct{512};
t1532 = ct{513};
t1533 = ct{514};
t1534 = ct{515};
t1535 = ct{516};
t1536 = ct{517};
t1537 = ct{518};
t1538 = ct{519};
t1539 = ct{520};
t154 = ct{521};
t1541 = ct{522};
t1542 = ct{523};
t1543 = ct{524};
t155 = ct{525};
t156 = ct{526};
t157 = ct{527};
t158 = ct{528};
t159 = ct{529};
t16 = ct{530};
t160 = ct{531};
t161 = ct{532};
t162 = ct{533};
t163 = ct{534};
t164 = ct{535};
t165 = ct{536};
t166 = ct{537};
t167 = ct{538};
t168 = ct{539};
t169 = ct{540};
t17 = ct{541};
t170 = ct{542};
t171 = ct{543};
t1711 = ct{544};
t1712 = ct{545};
t1713 = ct{546};
t1714 = ct{547};
t172 = ct{548};
t1728 = ct{549};
t173 = ct{550};
t1730 = ct{551};
t1732 = ct{552};
t1734 = ct{553};
t1736 = ct{554};
t1738 = ct{555};
t174 = ct{556};
t1740 = ct{557};
t1742 = ct{558};
t1743 = ct{559};
t1744 = ct{560};
t1745 = ct{561};
t1746 = ct{562};
t1747 = ct{563};
t1748 = ct{564};
t1749 = ct{565};
t175 = ct{566};
t1750 = ct{567};
t176 = ct{568};
t177 = ct{569};
t1775 = ct{570};
t1776 = ct{571};
t1777 = ct{572};
t1778 = ct{573};
t178 = ct{574};
t1783 = ct{575};
t1784 = ct{576};
t1785 = ct{577};
t1786 = ct{578};
t1787 = ct{579};
t1788 = ct{580};
t1789 = ct{581};
t179 = ct{582};
t1790 = ct{583};
t1791 = ct{584};
t1792 = ct{585};
t1793 = ct{586};
t1794 = ct{587};
t1795 = ct{588};
t1796 = ct{589};
t1797 = ct{590};
t1798 = ct{591};
t1799 = ct{592};
t18 = ct{593};
t180 = ct{594};
t1800 = ct{595};
t1801 = ct{596};
t1802 = ct{597};
t1803 = ct{598};
t1804 = ct{599};
t1805 = ct{600};
t1806 = ct{601};
t181 = ct{602};
t182 = ct{603};
t183 = ct{604};
t184 = ct{605};
t185 = ct{606};
t1865 = ct{607};
t1866 = ct{608};
t1867 = ct{609};
t1868 = ct{610};
t187 = ct{611};
t188 = ct{612};
t189 = ct{613};
t19 = ct{614};
t190 = ct{615};
t191 = ct{616};
t192 = ct{617};
t193 = ct{618};
t194 = ct{619};
t195 = ct{620};
t196 = ct{621};
t197 = ct{622};
t198 = ct{623};
t199 = ct{624};
t1994 = ct{625};
t1995 = ct{626};
t1996 = ct{627};
t1997 = ct{628};
t1998 = ct{629};
t1999 = ct{630};
t2 = ct{631};
t20 = ct{632};
t200 = ct{633};
t2000 = ct{634};
t2001 = ct{635};
t201 = ct{636};
t202 = ct{637};
t203 = ct{638};
t2034 = ct{639};
t2035 = ct{640};
t2036 = ct{641};
t2037 = ct{642};
t2038 = ct{643};
t2039 = ct{644};
t204 = ct{645};
t2040 = ct{646};
t2041 = ct{647};
t205 = ct{648};
t206 = ct{649};
t207 = ct{650};
t208 = ct{651};
t209 = ct{652};
t21 = ct{653};
t210 = ct{654};
t211 = ct{655};
t212 = ct{656};
t213 = ct{657};
t214 = ct{658};
t215 = ct{659};
t216 = ct{660};
t217 = ct{661};
t218 = ct{662};
t219 = ct{663};
t22 = ct{664};
t220 = ct{665};
t221 = ct{666};
t222 = ct{667};
t223 = ct{668};
t224 = ct{669};
t225 = ct{670};
t226 = ct{671};
t227 = ct{672};
t228 = ct{673};
t229 = ct{674};
t23 = ct{675};
t230 = ct{676};
t231 = ct{677};
t232 = ct{678};
t233 = ct{679};
t234 = ct{680};
t235 = ct{681};
t24 = ct{682};
t248 = ct{683};
t249 = ct{684};
t25 = ct{685};
t250 = ct{686};
t251 = ct{687};
t252 = ct{688};
t253 = ct{689};
t254 = ct{690};
t255 = ct{691};
t256 = ct{692};
t257 = ct{693};
t258 = ct{694};
t259 = ct{695};
t26 = ct{696};
t260 = ct{697};
t261 = ct{698};
t262 = ct{699};
t263 = ct{700};
t264 = ct{701};
t266 = ct{702};
t267 = ct{703};
t268 = ct{704};
t269 = ct{705};
t27 = ct{706};
t270 = ct{707};
t271 = ct{708};
t272 = ct{709};
t273 = ct{710};
t274 = ct{711};
t275 = ct{712};
t276 = ct{713};
t277 = ct{714};
t278 = ct{715};
t279 = ct{716};
t28 = ct{717};
t280 = ct{718};
t281 = ct{719};
t282 = ct{720};
t283 = ct{721};
t284 = ct{722};
t285 = ct{723};
t286 = ct{724};
t287 = ct{725};
t288 = ct{726};
t289 = ct{727};
t29 = ct{728};
t290 = ct{729};
t291 = ct{730};
t292 = ct{731};
t293 = ct{732};
t294 = ct{733};
t295 = ct{734};
t296 = ct{735};
t297 = ct{736};
t298 = ct{737};
t299 = ct{738};
t3 = ct{739};
t30 = ct{740};
t300 = ct{741};
t301 = ct{742};
t302 = ct{743};
t303 = ct{744};
t304 = ct{745};
t305 = ct{746};
t306 = ct{747};
t307 = ct{748};
t308 = ct{749};
t309 = ct{750};
t31 = ct{751};
t310 = ct{752};
t311 = ct{753};
t312 = ct{754};
t313 = ct{755};
t314 = ct{756};
t315 = ct{757};
t316 = ct{758};
t317 = ct{759};
t318 = ct{760};
t319 = ct{761};
t320 = ct{762};
t321 = ct{763};
t322 = ct{764};
t323 = ct{765};
t324 = ct{766};
t329 = ct{767};
t330 = ct{768};
t331 = ct{769};
t332 = ct{770};
t333 = ct{771};
t334 = ct{772};
t335 = ct{773};
t336 = ct{774};
t337 = ct{775};
t338 = ct{776};
t339 = ct{777};
t340 = ct{778};
t342 = ct{779};
t344 = ct{780};
t346 = ct{781};
t348 = ct{782};
t349 = ct{783};
t350 = ct{784};
t351 = ct{785};
t352 = ct{786};
t353 = ct{787};
t354 = ct{788};
t355 = ct{789};
t356 = ct{790};
t357 = ct{791};
t358 = ct{792};
t361 = ct{793};
t362 = ct{794};
t363 = ct{795};
t364 = ct{796};
t365 = ct{797};
t366 = ct{798};
t367 = ct{799};
t368 = ct{800};
t369 = ct{801};
t370 = ct{802};
t371 = ct{803};
t372 = ct{804};
t373 = ct{805};
t374 = ct{806};
t375 = ct{807};
t376 = ct{808};
t377 = ct{809};
t378 = ct{810};
t379 = ct{811};
t380 = ct{812};
t381 = ct{813};
t394 = ct{814};
t395 = ct{815};
t396 = ct{816};
t397 = ct{817};
t398 = ct{818};
t399 = ct{819};
t4 = ct{820};
t400 = ct{821};
t401 = ct{822};
t402 = ct{823};
t403 = ct{824};
t404 = ct{825};
t405 = ct{826};
t406 = ct{827};
t407 = ct{828};
t408 = ct{829};
t409 = ct{830};
t410 = ct{831};
t411 = ct{832};
t412 = ct{833};
t413 = ct{834};
t414 = ct{835};
t415 = ct{836};
t416 = ct{837};
t417 = ct{838};
t418 = ct{839};
t419 = ct{840};
t420 = ct{841};
t421 = ct{842};
t422 = ct{843};
t423 = ct{844};
t424 = ct{845};
t425 = ct{846};
t426 = ct{847};
t427 = ct{848};
t428 = ct{849};
t429 = ct{850};
t430 = ct{851};
t431 = ct{852};
t432 = ct{853};
t433 = ct{854};
t434 = ct{855};
t435 = ct{856};
t436 = ct{857};
t437 = ct{858};
t438 = ct{859};
t439 = ct{860};
t440 = ct{861};
t441 = ct{862};
t442 = ct{863};
t443 = ct{864};
t444 = ct{865};
t445 = ct{866};
t446 = ct{867};
t447 = ct{868};
t448 = ct{869};
t449 = ct{870};
t450 = ct{871};
t451 = ct{872};
t452 = ct{873};
t453 = ct{874};
t454 = ct{875};
t455 = ct{876};
t456 = ct{877};
t457 = ct{878};
t458 = ct{879};
t459 = ct{880};
t46 = ct{881};
t460 = ct{882};
t461 = ct{883};
t462 = ct{884};
t463 = ct{885};
t464 = ct{886};
t465 = ct{887};
t466 = ct{888};
t467 = ct{889};
t468 = ct{890};
t469 = ct{891};
t47 = ct{892};
t470 = ct{893};
t471 = ct{894};
t472 = ct{895};
t473 = ct{896};
t474 = ct{897};
t475 = ct{898};
t476 = ct{899};
t477 = ct{900};
t478 = ct{901};
t479 = ct{902};
t48 = ct{903};
t480 = ct{904};
t481 = ct{905};
t482 = ct{906};
t483 = ct{907};
t484 = ct{908};
t485 = ct{909};
t486 = ct{910};
t487 = ct{911};
t488 = ct{912};
t489 = ct{913};
t49 = ct{914};
t490 = ct{915};
t491 = ct{916};
t492 = ct{917};
t493 = ct{918};
t494 = ct{919};
t495 = ct{920};
t496 = ct{921};
t497 = ct{922};
t498 = ct{923};
t499 = ct{924};
t5 = ct{925};
t50 = ct{926};
t500 = ct{927};
t501 = ct{928};
t503 = ct{929};
t504 = ct{930};
t506 = ct{931};
t507 = ct{932};
t509 = ct{933};
t51 = ct{934};
t510 = ct{935};
t512 = ct{936};
t513 = ct{937};
t514 = ct{938};
t515 = ct{939};
t516 = ct{940};
t517 = ct{941};
t518 = ct{942};
t519 = ct{943};
t52 = ct{944};
t520 = ct{945};
t521 = ct{946};
t522 = ct{947};
t523 = ct{948};
t524 = ct{949};
t525 = ct{950};
t526 = ct{951};
t527 = ct{952};
t528 = ct{953};
t529 = ct{954};
t53 = ct{955};
t530 = ct{956};
t531 = ct{957};
t532 = ct{958};
t533 = ct{959};
t534 = ct{960};
t535 = ct{961};
t536 = ct{962};
t537 = ct{963};
t538 = ct{964};
t539 = ct{965};
t54 = ct{966};
t540 = ct{967};
t541 = ct{968};
t542 = ct{969};
t543 = ct{970};
t544 = ct{971};
t545 = ct{972};
t546 = ct{973};
t547 = ct{974};
t548 = ct{975};
t549 = ct{976};
t55 = ct{977};
t550 = ct{978};
t551 = ct{979};
t552 = ct{980};
t553 = ct{981};
t554 = ct{982};
t555 = ct{983};
t556 = ct{984};
t557 = ct{985};
t558 = ct{986};
t559 = ct{987};
t56 = ct{988};
t560 = ct{989};
t561 = ct{990};
t562 = ct{991};
t563 = ct{992};
t564 = ct{993};
t565 = ct{994};
t566 = ct{995};
t567 = ct{996};
t568 = ct{997};
t569 = ct{998};
t57 = ct{999};
t570 = ct{1000};
t571 = ct{1001};
t572 = ct{1002};
t573 = ct{1003};
t574 = ct{1004};
t575 = ct{1005};
t576 = ct{1006};
t577 = ct{1007};
t578 = ct{1008};
t579 = ct{1009};
t58 = ct{1010};
t580 = ct{1011};
t581 = ct{1012};
t582 = ct{1013};
t583 = ct{1014};
t584 = ct{1015};
t585 = ct{1016};
t586 = ct{1017};
t587 = ct{1018};
t588 = ct{1019};
t589 = ct{1020};
t59 = ct{1021};
t590 = ct{1022};
t591 = ct{1023};
t592 = ct{1024};
t593 = ct{1025};
t594 = ct{1026};
t595 = ct{1027};
t596 = ct{1028};
t597 = ct{1029};
t598 = ct{1030};
t599 = ct{1031};
t6 = ct{1032};
t60 = ct{1033};
t600 = ct{1034};
t601 = ct{1035};
t602 = ct{1036};
t603 = ct{1037};
t604 = ct{1038};
t605 = ct{1039};
t606 = ct{1040};
t607 = ct{1041};
t608 = ct{1042};
t609 = ct{1043};
t61 = ct{1044};
t610 = ct{1045};
t611 = ct{1046};
t612 = ct{1047};
t613 = ct{1048};
t614 = ct{1049};
t615 = ct{1050};
t616 = ct{1051};
t617 = ct{1052};
t618 = ct{1053};
t619 = ct{1054};
t62 = ct{1055};
t620 = ct{1056};
t621 = ct{1057};
t622 = ct{1058};
t623 = ct{1059};
t624 = ct{1060};
t625 = ct{1061};
t626 = ct{1062};
t627 = ct{1063};
t628 = ct{1064};
t629 = ct{1065};
t63 = ct{1066};
t630 = ct{1067};
t631 = ct{1068};
t632 = ct{1069};
t633 = ct{1070};
t634 = ct{1071};
t635 = ct{1072};
t636 = ct{1073};
t637 = ct{1074};
t638 = ct{1075};
t639 = ct{1076};
t64 = ct{1077};
t640 = ct{1078};
t641 = ct{1079};
t642 = ct{1080};
t643 = ct{1081};
t644 = ct{1082};
t645 = ct{1083};
t646 = ct{1084};
t647 = ct{1085};
t648 = ct{1086};
t649 = ct{1087};
t65 = ct{1088};
t650 = ct{1089};
t651 = ct{1090};
t652 = ct{1091};
t653 = ct{1092};
t654 = ct{1093};
t655 = ct{1094};
t656 = ct{1095};
t657 = ct{1096};
t66 = ct{1097};
t666 = ct{1098};
t667 = ct{1099};
t668 = ct{1100};
t669 = ct{1101};
t67 = ct{1102};
t670 = ct{1103};
t671 = ct{1104};
t672 = ct{1105};
t673 = ct{1106};
t674 = ct{1107};
t675 = ct{1108};
t676 = ct{1109};
t677 = ct{1110};
t678 = ct{1111};
t679 = ct{1112};
t68 = ct{1113};
t680 = ct{1114};
t681 = ct{1115};
t682 = ct{1116};
t683 = ct{1117};
t684 = ct{1118};
t685 = ct{1119};
t686 = ct{1120};
t687 = ct{1121};
t688 = ct{1122};
t689 = ct{1123};
t69 = ct{1124};
t690 = ct{1125};
t691 = ct{1126};
t692 = ct{1127};
t693 = ct{1128};
t694 = ct{1129};
t695 = ct{1130};
t696 = ct{1131};
t697 = ct{1132};
t698 = ct{1133};
t699 = ct{1134};
t7 = ct{1135};
t70 = ct{1136};
t700 = ct{1137};
t701 = ct{1138};
t702 = ct{1139};
t703 = ct{1140};
t704 = ct{1141};
t705 = ct{1142};
t706 = ct{1143};
t707 = ct{1144};
t708 = ct{1145};
t709 = ct{1146};
t71 = ct{1147};
t710 = ct{1148};
t711 = ct{1149};
t712 = ct{1150};
t713 = ct{1151};
t714 = ct{1152};
t715 = ct{1153};
t716 = ct{1154};
t717 = ct{1155};
t718 = ct{1156};
t719 = ct{1157};
t72 = ct{1158};
t720 = ct{1159};
t721 = ct{1160};
t722 = ct{1161};
t725 = ct{1162};
t726 = ct{1163};
t727 = ct{1164};
t728 = ct{1165};
t729 = ct{1166};
t73 = ct{1167};
t730 = ct{1168};
t731 = ct{1169};
t732 = ct{1170};
t733 = ct{1171};
t734 = ct{1172};
t735 = ct{1173};
t736 = ct{1174};
t737 = ct{1175};
t738 = ct{1176};
t739 = ct{1177};
t74 = ct{1178};
t740 = ct{1179};
t741 = ct{1180};
t742 = ct{1181};
t743 = ct{1182};
t744 = ct{1183};
t745 = ct{1184};
t746 = ct{1185};
t747 = ct{1186};
t748 = ct{1187};
t749 = ct{1188};
t75 = ct{1189};
t750 = ct{1190};
t751 = ct{1191};
t752 = ct{1192};
t753 = ct{1193};
t754 = ct{1194};
t755 = ct{1195};
t756 = ct{1196};
t757 = ct{1197};
t758 = ct{1198};
t759 = ct{1199};
t76 = ct{1200};
t760 = ct{1201};
t761 = ct{1202};
t762 = ct{1203};
t763 = ct{1204};
t764 = ct{1205};
t765 = ct{1206};
t766 = ct{1207};
t767 = ct{1208};
t768 = ct{1209};
t769 = ct{1210};
t77 = ct{1211};
t770 = ct{1212};
t771 = ct{1213};
t772 = ct{1214};
t773 = ct{1215};
t774 = ct{1216};
t775 = ct{1217};
t776 = ct{1218};
t777 = ct{1219};
t778 = ct{1220};
t779 = ct{1221};
t78 = ct{1222};
t780 = ct{1223};
t781 = ct{1224};
t782 = ct{1225};
t783 = ct{1226};
t784 = ct{1227};
t785 = ct{1228};
t786 = ct{1229};
t787 = ct{1230};
t788 = ct{1231};
t789 = ct{1232};
t79 = ct{1233};
t790 = ct{1234};
t791 = ct{1235};
t792 = ct{1236};
t793 = ct{1237};
t794 = ct{1238};
t795 = ct{1239};
t796 = ct{1240};
t797 = ct{1241};
t798 = ct{1242};
t799 = ct{1243};
t8 = ct{1244};
t80 = ct{1245};
t800 = ct{1246};
t801 = ct{1247};
t802 = ct{1248};
t803 = ct{1249};
t804 = ct{1250};
t805 = ct{1251};
t806 = ct{1252};
t807 = ct{1253};
t808 = ct{1254};
t809 = ct{1255};
t81 = ct{1256};
t810 = ct{1257};
t811 = ct{1258};
t812 = ct{1259};
t813 = ct{1260};
t814 = ct{1261};
t815 = ct{1262};
t816 = ct{1263};
t817 = ct{1264};
t818 = ct{1265};
t819 = ct{1266};
t82 = ct{1267};
t820 = ct{1268};
t821 = ct{1269};
t822 = ct{1270};
t823 = ct{1271};
t824 = ct{1272};
t825 = ct{1273};
t826 = ct{1274};
t827 = ct{1275};
t828 = ct{1276};
t83 = ct{1277};
t830 = ct{1278};
t831 = ct{1279};
t833 = ct{1280};
t834 = ct{1281};
t836 = ct{1282};
t837 = ct{1283};
t839 = ct{1284};
t84 = ct{1285};
t840 = ct{1286};
t841 = ct{1287};
t842 = ct{1288};
t843 = ct{1289};
t844 = ct{1290};
t845 = ct{1291};
t846 = ct{1292};
t847 = ct{1293};
t848 = ct{1294};
t849 = ct{1295};
t85 = ct{1296};
t850 = ct{1297};
t851 = ct{1298};
t852 = ct{1299};
t86 = ct{1300};
t866 = ct{1301};
t869 = ct{1302};
t87 = ct{1303};
t872 = ct{1304};
t875 = ct{1305};
t877 = ct{1306};
t878 = ct{1307};
t879 = ct{1308};
t88 = ct{1309};
t880 = ct{1310};
t881 = ct{1311};
t882 = ct{1312};
t883 = ct{1313};
t884 = ct{1314};
t885 = ct{1315};
t886 = ct{1316};
t887 = ct{1317};
t888 = ct{1318};
t889 = ct{1319};
t89 = ct{1320};
t890 = ct{1321};
t891 = ct{1322};
t892 = ct{1323};
t893 = ct{1324};
t894 = ct{1325};
t895 = ct{1326};
t896 = ct{1327};
t897 = ct{1328};
t898 = ct{1329};
t899 = ct{1330};
t9 = ct{1331};
t90 = ct{1332};
t900 = ct{1333};
t901 = ct{1334};
t902 = ct{1335};
t903 = ct{1336};
t904 = ct{1337};
t905 = ct{1338};
t906 = ct{1339};
t907 = ct{1340};
t908 = ct{1341};
t909 = ct{1342};
t91 = ct{1343};
t910 = ct{1344};
t911 = ct{1345};
t912 = ct{1346};
t913 = ct{1347};
t914 = ct{1348};
t915 = ct{1349};
t916 = ct{1350};
t917 = ct{1351};
t918 = ct{1352};
t919 = ct{1353};
t92 = ct{1354};
t920 = ct{1355};
t921 = ct{1356};
t922 = ct{1357};
t923 = ct{1358};
t924 = ct{1359};
t925 = ct{1360};
t926 = ct{1361};
t927 = ct{1362};
t928 = ct{1363};
t929 = ct{1364};
t93 = ct{1365};
t930 = ct{1366};
t931 = ct{1367};
t932 = ct{1368};
t933 = ct{1369};
t934 = ct{1370};
t935 = ct{1371};
t936 = ct{1372};
t937 = ct{1373};
t938 = ct{1374};
t939 = ct{1375};
t94 = ct{1376};
t940 = ct{1377};
t941 = ct{1378};
t942 = ct{1379};
t943 = ct{1380};
t944 = ct{1381};
t945 = ct{1382};
t946 = ct{1383};
t947 = ct{1384};
t948 = ct{1385};
t949 = ct{1386};
t95 = ct{1387};
t950 = ct{1388};
t951 = ct{1389};
t952 = ct{1390};
t953 = ct{1391};
t954 = ct{1392};
t955 = ct{1393};
t956 = ct{1394};
t957 = ct{1395};
t958 = ct{1396};
t96 = ct{1397};
t960 = ct{1398};
t961 = ct{1399};
t962 = ct{1400};
t963 = ct{1401};
t964 = ct{1402};
t965 = ct{1403};
t966 = ct{1404};
t967 = ct{1405};
t968 = ct{1406};
t969 = ct{1407};
t97 = ct{1408};
t970 = ct{1409};
t971 = ct{1410};
t972 = ct{1411};
t973 = ct{1412};
t974 = ct{1413};
t975 = ct{1414};
t976 = ct{1415};
t977 = ct{1416};
t978 = ct{1417};
t979 = ct{1418};
t98 = ct{1419};
t980 = ct{1420};
t981 = ct{1421};
t982 = ct{1422};
t983 = ct{1423};
t984 = ct{1424};
t985 = ct{1425};
t986 = ct{1426};
t987 = ct{1427};
t989 = ct{1428};
t99 = ct{1429};
t994 = ct{1430};
t995 = ct{1431};
t996 = ct{1432};
t997 = ct{1433};
t998 = ct{1434};
t999 = ct{1435};
th11_dot = ct{1436};
th12_dot = ct{1437};
th13_dot = ct{1438};
th21_dot = ct{1439};
th22_dot = ct{1440};
th23_dot = ct{1441};
th31_dot = ct{1442};
th32_dot = ct{1443};
th33_dot = ct{1444};
th41_dot = ct{1445};
th42_dot = ct{1446};
th43_dot = ct{1447};
zeta_dot = ct{1448};
t1544 = phi_dot.*t9.*t73.*t92.*(3.0./1.0e+3);
t1545 = phi_dot.*t11.*t73.*t92.*(3.0./1.0e+3);
t1546 = phi_dot.*t12.*t73.*t92.*(3.0./1.0e+3);
t1547 = phi_dot.*t14.*t73.*t92.*(3.0./1.0e+3);
t1548 = phi_dot.*t15.*t73.*t92.*(3.0./1.0e+3);
t1549 = t5.*t46.*t92.*zeta_dot.*(3.0./1.0e+3);
t1550 = t6.*t46.*t92.*zeta_dot.*(3.0./1.0e+3);
t1551 = t8.*t46.*t92.*zeta_dot.*(3.0./1.0e+3);
t1552 = t9.*t46.*t92.*zeta_dot.*(3.0./1.0e+3);
t1553 = t11.*t46.*t92.*zeta_dot.*(3.0./1.0e+3);
t1554 = t12.*t46.*t92.*zeta_dot.*(3.0./1.0e+3);
t1555 = t14.*t46.*t92.*zeta_dot.*(3.0./1.0e+3);
t1556 = t15.*t46.*t92.*zeta_dot.*(3.0./1.0e+3);
t1557 = phi_dot.*t19.*t74.*t87.*1.05e-2;
t1558 = phi_dot.*t20.*t74.*t87.*1.05e-2;
t1559 = phi_dot.*t21.*t74.*t87.*1.05e-2;
t1560 = phi_dot.*t22.*t74.*t87.*1.05e-2;
t1561 = phi_dot.*t23.*t74.*t87.*1.05e-2;
t1562 = phi_dot.*t24.*t74.*t87.*1.05e-2;
t1563 = phi_dot.*t25.*t74.*t87.*1.05e-2;
t1564 = phi_dot.*t26.*t74.*t87.*1.05e-2;
t1565 = phi_dot.*t27.*t74.*t87.*1.05e-2;
t1566 = phi_dot.*t28.*t74.*t87.*1.05e-2;
t1567 = phi_dot.*t29.*t74.*t87.*1.05e-2;
t1568 = phi_dot.*t30.*t74.*t87.*1.05e-2;
t1569 = t16.*t47.*t92.*zeta_dot.*(-2.0./3.75e+2);
t1570 = (t3.*t76.*t92.*th12_dot)./7.5e+2;
t1571 = (t3.*t77.*t92.*th13_dot)./7.5e+2;
t1572 = (t3.*t79.*t92.*th22_dot)./7.5e+2;
t1573 = (t3.*t80.*t92.*th23_dot)./7.5e+2;
t1574 = (t3.*t82.*t92.*th32_dot)./7.5e+2;
t1575 = (t3.*t83.*t92.*th33_dot)./7.5e+2;
t1576 = (t3.*t85.*t92.*th42_dot)./7.5e+2;
t1577 = (t3.*t86.*t92.*th43_dot)./7.5e+2;
t1578 = phi_dot.*t3.*t4.*t18.*t73.*(2.1e+1./1.0e+3);
t1579 = phi_dot.*t3.*t5.*t18.*t73.*(2.1e+1./1.0e+3);
t1580 = phi_dot.*t3.*t6.*t18.*t73.*(2.1e+1./1.0e+3);
t1581 = phi_dot.*t3.*t7.*t18.*t73.*(2.1e+1./1.0e+3);
t1582 = phi_dot.*t3.*t8.*t18.*t73.*(2.1e+1./1.0e+3);
t1583 = phi_dot.*t3.*t9.*t18.*t73.*(2.1e+1./1.0e+3);
t1584 = phi_dot.*t3.*t10.*t18.*t73.*(2.1e+1./1.0e+3);
t1585 = phi_dot.*t3.*t11.*t18.*t73.*(2.1e+1./1.0e+3);
t1586 = phi_dot.*t3.*t12.*t18.*t73.*(2.1e+1./1.0e+3);
t1587 = phi_dot.*t3.*t13.*t18.*t73.*(2.1e+1./1.0e+3);
t1588 = phi_dot.*t3.*t14.*t18.*t73.*(2.1e+1./1.0e+3);
t1589 = phi_dot.*t3.*t15.*t18.*t73.*(2.1e+1./1.0e+3);
t1590 = phi_dot.*t3.*t5.*t18.*t73.*1.35e-2;
t1591 = phi_dot.*t3.*t6.*t18.*t73.*1.35e-2;
t1592 = phi_dot.*t3.*t8.*t18.*t73.*1.35e-2;
t1593 = phi_dot.*t3.*t9.*t18.*t73.*1.35e-2;
t1594 = phi_dot.*t3.*t11.*t18.*t73.*1.35e-2;
t1595 = phi_dot.*t3.*t12.*t18.*t73.*1.35e-2;
t1596 = phi_dot.*t3.*t14.*t18.*t73.*1.35e-2;
t1597 = phi_dot.*t3.*t15.*t18.*t73.*1.35e-2;
t1598 = phi_dot.*t3.*t18.*t73.*5.21125e-1;
t1599 = t3.*t92.*t316;
t1600 = t3.*t92.*t317;
t1601 = t3.*t92.*t318;
t1602 = t3.*t92.*t319;
t1603 = t3.*t92.*t320;
t1604 = t3.*t92.*t321;
t1605 = t3.*t92.*t322;
t1606 = t3.*t92.*t323;
t1608 = phi_dot.*t3.*t18.*t60.*t73.*(4.0./3.75e+2);
t1609 = phi_dot.*t3.*t18.*t61.*t73.*(7.0./3.75e+2);
t1610 = phi_dot.*t3.*t18.*t62.*t73.*(7.0./3.75e+2);
t1611 = phi_dot.*t3.*t18.*t63.*t73.*(4.0./3.75e+2);
t1612 = phi_dot.*t3.*t18.*t64.*t73.*(7.0./3.75e+2);
t1613 = phi_dot.*t3.*t18.*t65.*t73.*(7.0./3.75e+2);
t1614 = phi_dot.*t3.*t18.*t66.*t73.*(4.0./3.75e+2);
t1615 = phi_dot.*t3.*t18.*t67.*t73.*(7.0./3.75e+2);
t1616 = phi_dot.*t3.*t18.*t68.*t73.*(7.0./3.75e+2);
t1617 = phi_dot.*t3.*t18.*t69.*t73.*(4.0./3.75e+2);
t1618 = phi_dot.*t3.*t18.*t70.*t73.*(7.0./3.75e+2);
t1619 = phi_dot.*t3.*t18.*t71.*t73.*(7.0./3.75e+2);
t1620 = phi_dot.*t3.*t18.*t73.*t92.*(2.0./3.75e+2);
t1621 = phi_dot.*t11.*t18.*t72.*t92.*(3.0./2.0e+2);
t1622 = phi_dot.*t12.*t18.*t72.*t92.*(3.0./2.0e+2);
t1623 = phi_dot.*t14.*t18.*t72.*t92.*(3.0./2.0e+2);
t1624 = phi_dot.*t15.*t18.*t72.*t92.*(3.0./2.0e+2);
t1625 = t18.*t72.*t92.*t113;
t1626 = t18.*t72.*t92.*t114;
t1627 = t18.*t72.*t92.*t116;
t1628 = t18.*t72.*t92.*t117;
t1629 = t3.*t18.*t61.*t92.*zeta_dot.*(4.0./3.75e+2);
t1630 = t3.*t18.*t62.*t92.*zeta_dot.*(4.0./3.75e+2);
t1631 = t3.*t18.*t64.*t92.*zeta_dot.*(4.0./3.75e+2);
t1632 = t3.*t18.*t65.*t92.*zeta_dot.*(4.0./3.75e+2);
t1633 = t3.*t18.*t67.*t92.*zeta_dot.*(4.0./3.75e+2);
t1634 = t3.*t18.*t68.*t92.*zeta_dot.*(4.0./3.75e+2);
t1635 = t3.*t18.*t70.*t92.*zeta_dot.*(4.0./3.75e+2);
t1636 = t3.*t18.*t71.*t92.*zeta_dot.*(4.0./3.75e+2);
t1645 = t97+t381;
t1651 = phi_dot.*t5.*t87.*t92.*5.25e-3;
t1652 = phi_dot.*t6.*t87.*t92.*5.25e-3;
t1653 = phi_dot.*t8.*t87.*t92.*5.25e-3;
t1654 = phi_dot.*t9.*t87.*t92.*5.25e-3;
t1655 = phi_dot.*t11.*t87.*t92.*5.25e-3;
t1656 = phi_dot.*t12.*t87.*t92.*5.25e-3;
t1657 = phi_dot.*t14.*t87.*t92.*5.25e-3;
t1658 = phi_dot.*t15.*t87.*t92.*5.25e-3;
t1659 = phi_dot.*t20.*t73.*t92.*4.5e-3;
t1660 = phi_dot.*t21.*t73.*t92.*4.5e-3;
t1661 = phi_dot.*t23.*t73.*t92.*4.5e-3;
t1662 = phi_dot.*t24.*t73.*t92.*4.5e-3;
t1663 = t73.*t917;
t1664 = t73.*t918;
t1665 = phi_dot.*t26.*t73.*t92.*4.5e-3;
t1666 = phi_dot.*t27.*t73.*t92.*4.5e-3;
t1667 = t73.*t919;
t1668 = t73.*t920;
t1669 = phi_dot.*t29.*t73.*t92.*4.5e-3;
t1670 = phi_dot.*t30.*t73.*t92.*4.5e-3;
t1671 = t73.*t921;
t1672 = t73.*t922;
t1673 = t73.*t923;
t1674 = t73.*t924;
t1675 = t20.*t46.*t92.*zeta_dot.*4.5e-3;
t1676 = t21.*t46.*t92.*zeta_dot.*4.5e-3;
t1677 = t23.*t46.*t92.*zeta_dot.*4.5e-3;
t1678 = t24.*t46.*t92.*zeta_dot.*4.5e-3;
t1679 = t5.*t74.*t92.*zeta_dot.*1.05e-2;
t1680 = t6.*t74.*t92.*zeta_dot.*1.05e-2;
t1681 = t26.*t46.*t92.*zeta_dot.*4.5e-3;
t1682 = t27.*t46.*t92.*zeta_dot.*4.5e-3;
t1683 = t8.*t74.*t92.*zeta_dot.*1.05e-2;
t1684 = t9.*t74.*t92.*zeta_dot.*1.05e-2;
t1685 = t29.*t46.*t92.*zeta_dot.*4.5e-3;
t1686 = t30.*t46.*t92.*zeta_dot.*4.5e-3;
t1687 = t11.*t74.*t92.*zeta_dot.*1.05e-2;
t1688 = t12.*t74.*t92.*zeta_dot.*1.05e-2;
t1689 = t14.*t74.*t92.*zeta_dot.*1.05e-2;
t1690 = t15.*t74.*t92.*zeta_dot.*1.05e-2;
t1691 = t47.*t935;
t1692 = t47.*t936;
t1693 = t47.*t937;
t1694 = t47.*t938;
t1695 = t47.*t939;
t1696 = t47.*t940;
t1697 = t47.*t941;
t1698 = t47.*t942;
t1699 = (phi_dot.*t46.*t48.*t87)./7.5e+2;
t1700 = (phi_dot.*t46.*t51.*t87)./7.5e+2;
t1701 = (phi_dot.*t46.*t54.*t87)./7.5e+2;
t1702 = (phi_dot.*t46.*t57.*t87)./7.5e+2;
t1703 = phi_dot.*t46.*t49.*t87.*2.333333333333333e-3;
t1704 = phi_dot.*t46.*t50.*t87.*2.333333333333333e-3;
t1705 = phi_dot.*t46.*t52.*t87.*2.333333333333333e-3;
t1706 = phi_dot.*t46.*t53.*t87.*2.333333333333333e-3;
t1707 = phi_dot.*t46.*t55.*t87.*2.333333333333333e-3;
t1708 = phi_dot.*t46.*t56.*t87.*2.333333333333333e-3;
t1709 = phi_dot.*t46.*t58.*t87.*2.333333333333333e-3;
t1710 = phi_dot.*t46.*t59.*t87.*2.333333333333333e-3;
t1719 = t92.*t638;
t1720 = t92.*t639;
t1721 = t92.*t641;
t1722 = t92.*t642;
t1723 = t92.*t644;
t1724 = t92.*t645;
t1725 = t92.*t647;
t1726 = t92.*t648;
t1727 = t3.*t92.*t361;
t1729 = t3.*t92.*t362;
t1731 = t3.*t92.*t363;
t1733 = t3.*t92.*t364;
t1735 = t3.*t92.*t365;
t1737 = t3.*t92.*t366;
t1739 = t3.*t92.*t367;
t1741 = t3.*t92.*t368;
t1751 = (t46.*t76.*t92.*zeta_dot)./3.75e+2;
t1752 = (t46.*t77.*t92.*zeta_dot)./3.75e+2;
t1753 = (t46.*t79.*t92.*zeta_dot)./3.75e+2;
t1754 = (t46.*t80.*t92.*zeta_dot)./3.75e+2;
t1755 = (t46.*t82.*t92.*zeta_dot)./3.75e+2;
t1756 = (t46.*t83.*t92.*zeta_dot)./3.75e+2;
t1757 = (t46.*t85.*t92.*zeta_dot)./3.75e+2;
t1758 = (t46.*t86.*t92.*zeta_dot)./3.75e+2;
t1759 = t5.*t16.*t20.*t92.*t139;
t1760 = t6.*t16.*t21.*t92.*t140;
t1761 = t8.*t16.*t23.*t92.*t142;
t1762 = t9.*t16.*t24.*t92.*t143;
t1763 = t11.*t16.*t26.*t92.*t145;
t1764 = t12.*t16.*t27.*t92.*t146;
t1765 = t14.*t16.*t29.*t92.*t148;
t1766 = t15.*t16.*t30.*t92.*t149;
t1767 = t31.*t1436;
t1768 = t31.*t1437;
t1769 = t31.*t1438;
t1770 = t31.*t1439;
t1771 = t31.*t1440;
t1772 = t31.*t1441;
t1773 = t31.*t1442;
t1774 = t31.*t1443;
t1779 = t18.*t31.*t92.*t191;
t1780 = t18.*t31.*t92.*t193;
t1781 = t18.*t31.*t92.*t197;
t1782 = t18.*t31.*t92.*t199;
t1808 = phi_dot.*t5.*t16.*t74.*t92.*(3.0./1.0e+3);
t1809 = phi_dot.*t6.*t16.*t74.*t92.*(3.0./1.0e+3);
t1810 = phi_dot.*t8.*t16.*t74.*t92.*(3.0./1.0e+3);
t1811 = phi_dot.*t9.*t16.*t74.*t92.*(3.0./1.0e+3);
t1812 = phi_dot.*t11.*t16.*t74.*t92.*(3.0./1.0e+3);
t1813 = phi_dot.*t12.*t16.*t74.*t92.*(3.0./1.0e+3);
t1814 = phi_dot.*t14.*t16.*t74.*t92.*(3.0./1.0e+3);
t1815 = phi_dot.*t15.*t16.*t74.*t92.*(3.0./1.0e+3);
t1816 = phi_dot.*t16.*t20.*t47.*t92.*(3.0./1.0e+3);
t1817 = phi_dot.*t16.*t21.*t47.*t92.*(3.0./1.0e+3);
t1818 = phi_dot.*t16.*t23.*t47.*t92.*(3.0./1.0e+3);
t1819 = phi_dot.*t16.*t24.*t47.*t92.*(3.0./1.0e+3);
t1820 = phi_dot.*t16.*t26.*t47.*t92.*(3.0./1.0e+3);
t1821 = phi_dot.*t16.*t27.*t47.*t92.*(3.0./1.0e+3);
t1822 = phi_dot.*t16.*t29.*t47.*t92.*(3.0./1.0e+3);
t1823 = phi_dot.*t16.*t30.*t47.*t92.*(3.0./1.0e+3);
t1824 = psi_dot.*t5.*t16.*t74.*t92.*(3.0./1.0e+3);
t1825 = psi_dot.*t6.*t16.*t74.*t92.*(3.0./1.0e+3);
t1826 = psi_dot.*t8.*t16.*t74.*t92.*(3.0./1.0e+3);
t1827 = psi_dot.*t9.*t16.*t74.*t92.*(3.0./1.0e+3);
t1828 = psi_dot.*t11.*t16.*t74.*t92.*(3.0./1.0e+3);
t1829 = psi_dot.*t12.*t16.*t74.*t92.*(3.0./1.0e+3);
t1830 = psi_dot.*t14.*t16.*t74.*t92.*(3.0./1.0e+3);
t1831 = psi_dot.*t15.*t16.*t74.*t92.*(3.0./1.0e+3);
t1832 = t46.*t1308;
t1833 = t46.*t1309;
t1834 = t46.*t1310;
t1835 = t46.*t1311;
t1836 = t46.*t1312;
t1837 = t46.*t1313;
t1838 = t46.*t1314;
t1839 = t46.*t1315;
t1841 = t16.*t20.*t47.*t92.*zeta_dot.*(3.0./1.0e+3);
t1842 = t16.*t21.*t47.*t92.*zeta_dot.*(3.0./1.0e+3);
t1843 = t16.*t23.*t47.*t92.*zeta_dot.*(3.0./1.0e+3);
t1844 = t16.*t24.*t47.*t92.*zeta_dot.*(3.0./1.0e+3);
t1845 = t16.*t26.*t47.*t92.*zeta_dot.*(3.0./1.0e+3);
t1846 = t16.*t27.*t47.*t92.*zeta_dot.*(3.0./1.0e+3);
t1847 = t16.*t29.*t47.*t92.*zeta_dot.*(3.0./1.0e+3);
t1848 = t16.*t30.*t47.*t92.*zeta_dot.*(3.0./1.0e+3);
t1849 = (phi_dot.*t18.*t31.*t49.*t92)./7.5e+2;
t1850 = (phi_dot.*t18.*t31.*t50.*t92)./7.5e+2;
t1851 = (phi_dot.*t18.*t31.*t52.*t92)./7.5e+2;
t1852 = (phi_dot.*t18.*t31.*t53.*t92)./7.5e+2;
t1853 = (phi_dot.*t18.*t31.*t55.*t92)./7.5e+2;
t1854 = (phi_dot.*t18.*t31.*t56.*t92)./7.5e+2;
t1855 = (phi_dot.*t18.*t31.*t58.*t92)./7.5e+2;
t1856 = (phi_dot.*t18.*t31.*t59.*t92)./7.5e+2;
t1869 = (phi_dot.*t3.*t16.*t31.*t61.*t92)./3.75e+2;
t1870 = (phi_dot.*t3.*t16.*t31.*t62.*t92)./3.75e+2;
t1871 = (phi_dot.*t3.*t16.*t31.*t64.*t92)./3.75e+2;
t1872 = (phi_dot.*t3.*t16.*t31.*t65.*t92)./3.75e+2;
t1873 = (phi_dot.*t3.*t16.*t31.*t67.*t92)./3.75e+2;
t1874 = (phi_dot.*t3.*t16.*t31.*t68.*t92)./3.75e+2;
t1875 = (phi_dot.*t3.*t16.*t31.*t70.*t92)./3.75e+2;
t1876 = (phi_dot.*t3.*t16.*t31.*t71.*t92)./3.75e+2;
t1877 = t46.*t1464;
t1878 = t46.*t1465;
t1879 = t46.*t1468;
t1880 = t46.*t1469;
t1881 = t46.*t1472;
t1882 = t46.*t1473;
t1883 = t46.*t1474;
t1884 = t46.*t1475;
t1885 = t47.*t1460;
t1886 = t47.*t1461;
t1887 = t47.*t1462;
t1888 = t47.*t1463;
t1889 = t47.*t1466;
t1890 = t47.*t1467;
t1891 = t47.*t1470;
t1892 = t47.*t1471;
t1893 = t46.*t1476;
t1894 = t46.*t1477;
t1895 = t46.*t1478;
t1896 = t46.*t1479;
t1897 = t46.*t1480;
t1898 = t46.*t1481;
t1899 = t46.*t1482;
t1900 = t46.*t1483;
t1901 = t46.*t1484;
t1902 = t46.*t1485;
t1903 = t46.*t1486;
t1904 = t46.*t1487;
t1905 = t46.*t1488;
t1906 = t46.*t1489;
t1907 = t46.*t1490;
t1908 = t46.*t1491;
t1917 = t5.*t16.*t47.*t92.*zeta_dot.*4.5e-3;
t1918 = t6.*t16.*t47.*t92.*zeta_dot.*4.5e-3;
t1919 = t8.*t16.*t47.*t92.*zeta_dot.*4.5e-3;
t1920 = t9.*t16.*t47.*t92.*zeta_dot.*4.5e-3;
t1921 = t11.*t16.*t47.*t92.*zeta_dot.*4.5e-3;
t1922 = t12.*t16.*t47.*t92.*zeta_dot.*4.5e-3;
t1923 = t14.*t16.*t47.*t92.*zeta_dot.*4.5e-3;
t1924 = t15.*t16.*t47.*t92.*zeta_dot.*4.5e-3;
t1929 = t16.*t20.*t46.*t92.*th12_dot.*(-1.5e-3);
t1930 = t16.*t23.*t46.*t92.*th22_dot.*(-1.5e-3);
t1931 = t16.*t26.*t46.*t92.*th32_dot.*(-1.5e-3);
t1932 = t16.*t29.*t46.*t92.*th42_dot.*(-1.5e-3);
t1933 = phi_dot.*t16.*t20.*t74.*t92.*4.5e-3;
t1934 = phi_dot.*t16.*t21.*t74.*t92.*4.5e-3;
t1935 = phi_dot.*t16.*t23.*t74.*t92.*4.5e-3;
t1936 = phi_dot.*t16.*t24.*t74.*t92.*4.5e-3;
t1937 = phi_dot.*t16.*t26.*t74.*t92.*4.5e-3;
t1938 = phi_dot.*t16.*t27.*t74.*t92.*4.5e-3;
t1939 = phi_dot.*t16.*t29.*t74.*t92.*4.5e-3;
t1940 = phi_dot.*t16.*t30.*t74.*t92.*4.5e-3;
t1941 = psi_dot.*t16.*t20.*t74.*t92.*4.5e-3;
t1942 = psi_dot.*t16.*t21.*t74.*t92.*4.5e-3;
t1943 = psi_dot.*t16.*t23.*t74.*t92.*4.5e-3;
t1944 = psi_dot.*t16.*t24.*t74.*t92.*4.5e-3;
t1945 = psi_dot.*t16.*t26.*t74.*t92.*4.5e-3;
t1946 = psi_dot.*t16.*t27.*t74.*t92.*4.5e-3;
t1947 = psi_dot.*t16.*t29.*t74.*t92.*4.5e-3;
t1948 = psi_dot.*t16.*t30.*t74.*t92.*4.5e-3;
t1950 = t3.*t31.*t77.*t92.*th13_dot.*(-1.0./7.5e+2);
t1951 = t3.*t31.*t80.*t92.*th23_dot.*(-1.0./7.5e+2);
t1952 = t3.*t31.*t83.*t92.*th33_dot.*(-1.0./7.5e+2);
t1953 = t3.*t31.*t86.*t92.*th43_dot.*(-1.0./7.5e+2);
t1954 = t16.*t20.*t74.*t92.*th12_dot.*5.25e-3;
t1955 = t16.*t21.*t74.*t92.*th13_dot.*5.25e-3;
t1956 = t16.*t23.*t74.*t92.*th22_dot.*5.25e-3;
t1957 = t16.*t24.*t74.*t92.*th23_dot.*5.25e-3;
t1958 = t16.*t26.*t74.*t92.*th32_dot.*5.25e-3;
t1959 = t16.*t27.*t74.*t92.*th33_dot.*5.25e-3;
t1960 = t16.*t29.*t74.*t92.*th42_dot.*5.25e-3;
t1961 = t16.*t30.*t74.*t92.*th43_dot.*5.25e-3;
t1962 = phi_dot.*t16.*t47.*t61.*t92.*(4.0./3.75e+2);
t1963 = phi_dot.*t16.*t47.*t62.*t92.*(4.0./3.75e+2);
t1964 = phi_dot.*t16.*t47.*t64.*t92.*(4.0./3.75e+2);
t1965 = phi_dot.*t16.*t47.*t65.*t92.*(4.0./3.75e+2);
t1966 = phi_dot.*t16.*t47.*t67.*t92.*(4.0./3.75e+2);
t1967 = phi_dot.*t16.*t47.*t68.*t92.*(4.0./3.75e+2);
t1968 = phi_dot.*t16.*t47.*t70.*t92.*(4.0./3.75e+2);
t1969 = phi_dot.*t16.*t47.*t71.*t92.*(4.0./3.75e+2);
t1978 = t46.*t49.*t558;
t1979 = t46.*t50.*t559;
t1980 = t46.*t52.*t560;
t1981 = t46.*t53.*t561;
t1982 = t46.*t55.*t562;
t1983 = t46.*t56.*t563;
t1984 = t46.*t58.*t564;
t1985 = t46.*t59.*t565;
t1986 = t16.*t47.*t61.*t92.*zeta_dot.*(4.0./3.75e+2);
t1987 = t16.*t47.*t62.*t92.*zeta_dot.*(4.0./3.75e+2);
t1988 = t16.*t47.*t64.*t92.*zeta_dot.*(4.0./3.75e+2);
t1989 = t16.*t47.*t65.*t92.*zeta_dot.*(4.0./3.75e+2);
t1990 = t16.*t47.*t67.*t92.*zeta_dot.*(4.0./3.75e+2);
t1991 = t16.*t47.*t68.*t92.*zeta_dot.*(4.0./3.75e+2);
t1992 = t16.*t47.*t70.*t92.*zeta_dot.*(4.0./3.75e+2);
t1993 = t16.*t47.*t71.*t92.*zeta_dot.*(4.0./3.75e+2);
t2002 = (phi_dot.*t16.*t74.*t76.*t92)./3.75e+2;
t2003 = (phi_dot.*t16.*t74.*t77.*t92)./3.75e+2;
t2004 = (phi_dot.*t16.*t74.*t79.*t92)./3.75e+2;
t2005 = (phi_dot.*t16.*t74.*t80.*t92)./3.75e+2;
t2006 = (phi_dot.*t16.*t74.*t82.*t92)./3.75e+2;
t2007 = (phi_dot.*t16.*t74.*t83.*t92)./3.75e+2;
t2008 = (phi_dot.*t16.*t74.*t85.*t92)./3.75e+2;
t2009 = (phi_dot.*t16.*t74.*t86.*t92)./3.75e+2;
t2010 = (psi_dot.*t16.*t74.*t76.*t92)./3.75e+2;
t2011 = (psi_dot.*t16.*t74.*t77.*t92)./3.75e+2;
t2012 = (psi_dot.*t16.*t74.*t79.*t92)./3.75e+2;
t2013 = (psi_dot.*t16.*t74.*t80.*t92)./3.75e+2;
t2014 = (psi_dot.*t16.*t74.*t82.*t92)./3.75e+2;
t2015 = (psi_dot.*t16.*t74.*t83.*t92)./3.75e+2;
t2016 = (psi_dot.*t16.*t74.*t85.*t92)./3.75e+2;
t2017 = (psi_dot.*t16.*t74.*t86.*t92)./3.75e+2;
t2018 = t92.*t1107;
t2019 = t92.*t1108;
t2020 = t92.*t1110;
t2021 = t92.*t1111;
t2022 = t92.*t1113;
t2023 = t92.*t1114;
t2024 = t92.*t1116;
t2025 = t92.*t1117;
t2026 = t3.*t92.*t692;
t2027 = t3.*t92.*t694;
t2028 = t3.*t92.*t696;
t2029 = t3.*t92.*t698;
t2030 = t3.*t92.*t704;
t2031 = t3.*t92.*t706;
t2032 = t3.*t92.*t712;
t2033 = t3.*t92.*t714;
t2042 = t16.*t18.*t92.*t438;
t2043 = t16.*t18.*t92.*t439;
t2044 = t16.*t18.*t92.*t440;
t2045 = t16.*t18.*t92.*t441;
t2046 = t16.*t18.*t92.*t442;
t2047 = t16.*t18.*t92.*t443;
t2048 = t16.*t18.*t92.*t444;
t2049 = t16.*t18.*t92.*t445;
t2050 = phi_dot.*t3.*t18.*t20.*t73.*t92.*(3.0./1.0e+3);
t2051 = phi_dot.*t3.*t18.*t21.*t73.*t92.*(3.0./1.0e+3);
t2052 = phi_dot.*t3.*t18.*t23.*t73.*t92.*(3.0./1.0e+3);
t2053 = phi_dot.*t3.*t18.*t24.*t73.*t92.*(3.0./1.0e+3);
t2054 = phi_dot.*t3.*t18.*t26.*t73.*t92.*(3.0./1.0e+3);
t2055 = phi_dot.*t3.*t18.*t27.*t73.*t92.*(3.0./1.0e+3);
t2056 = phi_dot.*t3.*t18.*t29.*t73.*t92.*(3.0./1.0e+3);
t2057 = phi_dot.*t3.*t18.*t30.*t73.*t92.*(3.0./1.0e+3);
t2058 = psi_dot.*t5.*t16.*t46.*t92.*(-1.05e-2);
t2059 = psi_dot.*t9.*t16.*t46.*t92.*(-1.05e-2);
t2060 = psi_dot.*t12.*t16.*t46.*t92.*(-1.05e-2);
t2061 = psi_dot.*t14.*t16.*t46.*t92.*(-1.05e-2);
t2062 = t6.*t16.*t46.*t92.*th13_dot.*(-2.25e-3);
t2063 = t9.*t16.*t46.*t92.*th23_dot.*(-2.25e-3);
t2064 = t12.*t16.*t46.*t92.*th33_dot.*(-2.25e-3);
t2065 = t15.*t16.*t46.*t92.*th43_dot.*(-2.25e-3);
t2075 = t16.*t46.*t50.*t92.*th13_dot.*(-1.0./3.75e+2);
t2076 = t16.*t46.*t53.*t92.*th23_dot.*(-1.0./3.75e+2);
t2077 = t16.*t46.*t56.*t92.*th33_dot.*(-1.0./3.75e+2);
t2078 = t16.*t46.*t59.*t92.*th43_dot.*(-1.0./3.75e+2);
t2079 = (phi_dot.*t18.*t49.*t72.*t92)./7.5e+2;
t2080 = (phi_dot.*t18.*t50.*t72.*t92)./7.5e+2;
t2081 = (phi_dot.*t18.*t52.*t72.*t92)./7.5e+2;
t2082 = (phi_dot.*t18.*t53.*t72.*t92)./7.5e+2;
t2083 = (phi_dot.*t18.*t55.*t72.*t92)./7.5e+2;
t2084 = (phi_dot.*t18.*t56.*t72.*t92)./7.5e+2;
t2085 = (phi_dot.*t18.*t58.*t72.*t92)./7.5e+2;
t2086 = (phi_dot.*t18.*t59.*t72.*t92)./7.5e+2;
t2087 = phi_dot.*t5.*t74.*t87.*t92.*1.5e-3;
t2088 = phi_dot.*t6.*t74.*t87.*t92.*1.5e-3;
t2089 = phi_dot.*t8.*t74.*t87.*t92.*1.5e-3;
t2090 = phi_dot.*t9.*t74.*t87.*t92.*1.5e-3;
t2091 = phi_dot.*t11.*t74.*t87.*t92.*1.5e-3;
t2092 = phi_dot.*t12.*t74.*t87.*t92.*1.5e-3;
t2093 = phi_dot.*t14.*t74.*t87.*t92.*1.5e-3;
t2094 = phi_dot.*t15.*t74.*t87.*t92.*1.5e-3;
t2100 = phi_dot.*t3.*t18.*t61.*t73.*t92.*(4.0./3.75e+2);
t2101 = phi_dot.*t3.*t18.*t62.*t73.*t92.*(4.0./3.75e+2);
t2102 = phi_dot.*t3.*t18.*t64.*t73.*t92.*(4.0./3.75e+2);
t2103 = phi_dot.*t3.*t18.*t65.*t73.*t92.*(4.0./3.75e+2);
t2104 = phi_dot.*t3.*t18.*t67.*t73.*t92.*(4.0./3.75e+2);
t2105 = phi_dot.*t3.*t18.*t68.*t73.*t92.*(4.0./3.75e+2);
t2106 = phi_dot.*t3.*t18.*t70.*t73.*t92.*(4.0./3.75e+2);
t2107 = phi_dot.*t3.*t18.*t71.*t73.*t92.*(4.0./3.75e+2);
t2108 = phi_dot.*t5.*t20.*t47.*t73.*t92.*(4.0./3.75e+2);
t2109 = phi_dot.*t6.*t21.*t47.*t73.*t92.*(4.0./3.75e+2);
t2110 = phi_dot.*t8.*t23.*t47.*t73.*t92.*(4.0./3.75e+2);
t2111 = phi_dot.*t9.*t24.*t47.*t73.*t92.*(4.0./3.75e+2);
t2112 = phi_dot.*t11.*t26.*t47.*t73.*t92.*(4.0./3.75e+2);
t2113 = phi_dot.*t12.*t27.*t47.*t73.*t92.*(4.0./3.75e+2);
t2114 = phi_dot.*t14.*t29.*t47.*t73.*t92.*(4.0./3.75e+2);
t2115 = phi_dot.*t15.*t30.*t47.*t73.*t92.*(4.0./3.75e+2);
t2124 = phi_dot.*t20.*t47.*t73.*t92.*(9.0./1.0e+3);
t2125 = phi_dot.*t21.*t47.*t73.*t92.*(9.0./1.0e+3);
t2126 = phi_dot.*t23.*t47.*t73.*t92.*(9.0./1.0e+3);
t2127 = phi_dot.*t24.*t47.*t73.*t92.*(9.0./1.0e+3);
t2128 = phi_dot.*t26.*t47.*t73.*t92.*(9.0./1.0e+3);
t2129 = phi_dot.*t27.*t47.*t73.*t92.*(9.0./1.0e+3);
t2130 = phi_dot.*t29.*t47.*t73.*t92.*(9.0./1.0e+3);
t2131 = phi_dot.*t30.*t47.*t73.*t92.*(9.0./1.0e+3);
t2140 = phi_dot.*t20.*t74.*t87.*t92.*2.25e-3;
t2141 = phi_dot.*t21.*t74.*t87.*t92.*2.25e-3;
t2142 = phi_dot.*t23.*t74.*t87.*t92.*2.25e-3;
t2143 = phi_dot.*t24.*t74.*t87.*t92.*2.25e-3;
t2144 = phi_dot.*t26.*t74.*t87.*t92.*2.25e-3;
t2145 = phi_dot.*t27.*t74.*t87.*t92.*2.25e-3;
t2146 = phi_dot.*t29.*t74.*t87.*t92.*2.25e-3;
t2147 = phi_dot.*t30.*t74.*t87.*t92.*2.25e-3;
t2158 = phi_dot.*t3.*t5.*t18.*t73.*t92.*4.5e-3;
t2159 = phi_dot.*t3.*t6.*t18.*t73.*t92.*4.5e-3;
t2160 = phi_dot.*t3.*t8.*t18.*t73.*t92.*4.5e-3;
t2161 = phi_dot.*t3.*t9.*t18.*t73.*t92.*4.5e-3;
t2162 = phi_dot.*t3.*t11.*t18.*t73.*t92.*4.5e-3;
t2163 = phi_dot.*t3.*t12.*t18.*t73.*t92.*4.5e-3;
t2164 = phi_dot.*t3.*t14.*t18.*t73.*t92.*4.5e-3;
t2165 = phi_dot.*t3.*t15.*t18.*t73.*t92.*4.5e-3;
t110 = -t98;
t111 = -t99;
t325 = t31.*t165;
t326 = t31.*t166;
t327 = t31.*t167;
t328 = t31.*t168;
t341 = t3.*t188;
t343 = t3.*t194;
t345 = t3.*t200;
t347 = t3.*t206;
t359 = t88+t100;
t360 = t91+t101;
t658 = t31.*t342;
t659 = t16.*t18.*t188;
t660 = t31.*t344;
t661 = t16.*t18.*t194;
t662 = t31.*t346;
t663 = t16.*t18.*t200;
t664 = t31.*t348;
t665 = t16.*t18.*t206;
t853 = t48.*t252;
t854 = t49.*t253;
t855 = t50.*t254;
t856 = t51.*t255;
t857 = t52.*t256;
t858 = t53.*t257;
t859 = t54.*t258;
t860 = t55.*t259;
t861 = t56.*t260;
t862 = t57.*t261;
t863 = t58.*t262;
t864 = t59.*t263;
t865 = t61.*t264;
t867 = t62.*t264;
t868 = t64.*t264;
